simulink model "MIL4L3_SW6_V1_20220211"  (R2018b)
settings: Solver=FixedStepAuto  StartTime=0.0  StopTime=inf  FixedStep=0.001  RelTol=1e-3
PreLoadFcn:
  | A0_MILtest;
undefined symbols (not defined in the file or in its folder): Clb_ICADirect_LaneDisp_StateFive, Clb_ICADirect_LaneDisp_StateFour, Clb_ICADirect_LaneDisp_StateOne, Clb_ICADirect_LaneDisp_StateThree, Clb_ICADirect_LaneDisp_StateTwo, Clb_ICADirect_LaneDisp_StateZero, Clb_ICADirect_LaneDispSW, Clb_ICADirect_TrnLghtsCom_Switch, Clb_ICADirect_TrnLghtsCom_Value, Clb_ICADirect_TrnLghtsCrtl_Inhb, IMAP_Clb_ACU_Driver_Belt, IMAP_Clb_ACU_Driver_Belt_Over, IMAP_Clb_ACU_Passenger_Belt, IMAP_Clb_ACU_Passenger_Belt_Over, IMAP_Clb_ACU_RearLeft_Belt, IMAP_Clb_ACU_RearLeft_Belt_Over, IMAP_Clb_ACU_RearMiddle_Belt, IMAP_Clb_ACU_RearMiddle_Belt_Over, IMAP_Clb_ACU_RearRight_Belt, IMAP_Clb_ACU_RearRight_Belt_Over, IMAP_Clb_AEB_Switch, IMAP_Clb_AEB_Switch_Over, IMAP_Clb_ALC_TLC_Mode, IMAP_Clb_ALC_TLC_Mode_Over, IMAP_Clb_BCM_Battery_Voltage, IMAP_Clb_BCM_Battery_Voltage_Over, IMAP_Clb_BCM_BrakeLamp_State, IMAP_Clb_BCM_BrakeLamp_State_Over, IMAP_Clb_BCM_CHMSL_Status, IMAP_Clb_BCM_CHMSL_Status_Over, IMAP_Clb_BCM_Door_Lock_State, IMAP_Clb_BCM_Door_Lock_State_Over, IMAP_Clb_BCM_FrontWiper_State, IMAP_Clb_BCM_FrontWiper_State_Over, IMAP_Clb_BCM_FrontWiper_Switch, IMAP_Clb_BCM_FrontWiper_Switch_Over, IMAP_Clb_BCM_HazardLamp, IMAP_Clb_BCM_HazardLamp_Over, IMAP_Clb_BCM_HazardLamp_Switch, IMAP_Clb_BCM_HazardLamp_Switch_Over, IMAP_Clb_BCM_HighBeam_State, IMAP_Clb_BCM_HighBeam_State_Over, IMAP_Clb_BCM_Ignition_State, IMAP_Clb_BCM_Ignition_State_Over, IMAP_Clb_BCM_IHBC_Enabled, IMAP_Clb_BCM_IHBC_Enabled_Over, IMAP_Clb_BCM_Left_Light, IMAP_Clb_BCM_Left_Light_Over, IMAP_Clb_BCM_LeftTurn_Switch, IMAP_Clb_BCM_LeftTurn_Switch_Over, IMAP_Clb_BCM_LF_Door_State, IMAP_Clb_BCM_LF_Door_State_Over, IMAP_Clb_BCM_LowBeam_State, IMAP_Clb_BCM_LowBeam_State_Over, IMAP_Clb_BCM_LR_Door_State, IMAP_Clb_BCM_LR_Door_State_Over, IMAP_Clb_BCM_RF_Door_State, IMAP_Clb_BCM_RF_Door_State_Over, IMAP_Clb_BCM_Right_Light, IMAP_Clb_BCM_Right_Light_Over ... (+547)
libraries: CarMaker4SL x2153, simulink x292, dspstat3 x3, canmsglib x2, simulink_extras x1
(part 21 of 52)

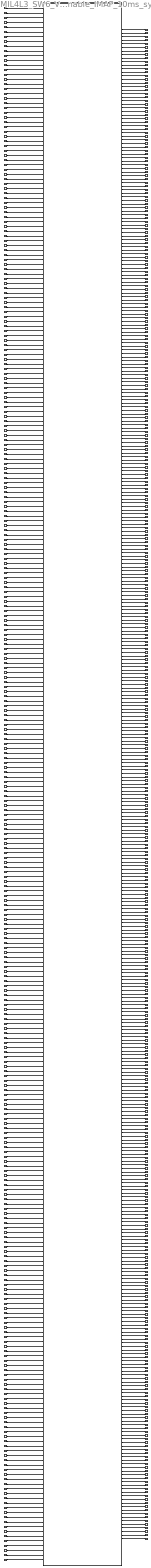
== system MIL4L3_SW6_V1_20220211/CarMaker/VehicleControl/Data Inport/IMAP/Runnable_IMAP_10ms_sys ==
  SWINve_y_ESC_ABSWorkLable : Inport  OutDataTypeStr=UInt8  PortDimensions=1
  SWINve_g_ESC_LongitudinalAcceleration : Inport  Port=2  OutDataTypeStr=T_M_Nm_Float32  PortDimensions=1
  SWINve_y_ESC_ESCOFF : Inport  Port=3  OutDataTypeStr=UInt8  PortDimensions=1
  SWINve_y_ESC_TCSCtlActive : Inport  Port=4  OutDataTypeStr=UInt8  PortDimensions=1
  SWINve_y_BCM_BrakeLampStaus : Inport  Port=5  OutDataTypeStr=UInt8  PortDimensions=1
  SWINve_y_BCM_CHMSLStaus : Inport  Port=6  OutDataTypeStr=UInt8  PortDimensions=1
  SWINve_y_BCM_FrontWiperWorkSt : Inport  Port=7  OutDataTypeStr=UInt8  PortDimensions=1
  SWINve_y_BCM_HazardLampSt : Inport  Port=8  OutDataTypeStr=UInt8  PortDimensions=1
  SWINve_y_EMS_BrakePedalSignal : Inport  Port=9  OutDataTypeStr=UInt8  PortDimensions=1
  SWINve_y_ESC_BrakingEffort : Inport  Port=10  OutDataTypeStr=UInt8  PortDimensions=1
  SWINve_y_ESC_DynamicSlope : Inport  Port=11  OutDataTypeStr=SInt8  PortDimensions=1
  SWINve_y_ESC_DynamicSlopeAccuracy : Inport  Port=12  OutDataTypeStr=UInt8  PortDimensions=1
  SWINve_y_EMS_WhetherACCRequestRealized : Inport  Port=13  OutDataTypeStr=UInt8  PortDimensions=1
  SWINve_y_EMS_ACCcontrolTorqueAvailable : Inport  Port=14  OutDataTypeStr=UInt8  PortDimensions=1
  SWINve_g_EMS_AccPedalPositionRaw : Inport  Port=15  OutDataTypeStr=T_M_Nm_Float32  PortDimensions=1
  SWINve_g_EMS_EngActualFlwTorque : Inport  Port=16  OutDataTypeStr=T_M_Nm_Float32  PortDimensions=1
  SWINve_d_EMS_RealizedPowertrainWheelTorq : Inport  Port=17  OutDataTypeStr=SInt16  PortDimensions=1
  SWINve_g_EMS_AccPedalPos : Inport  Port=18  OutDataTypeStr=T_M_Nm_Float32  PortDimensions=1
  SWINve_g_EMS_DriverTorque : Inport  Port=19  OutDataTypeStr=T_M_Nm_Float32  PortDimensions=1
  SWINve_g_EMS_EngSpd : Inport  Port=20  OutDataTypeStr=T_M_Nm_Float32  PortDimensions=1
  SWINve_y_EMS_EngRunningStatus : Inport  Port=21  OutDataTypeStr=UInt8  PortDimensions=1
  SWINve_y_EMS_ACCcontrolGearAvailable : Inport  Port=22  OutDataTypeStr=UInt8  PortDimensions=1
  SWINve_g_EMS_MaxPowertrainWheelTorque : Inport  Port=23  OutDataTypeStr=T_M_Nm_Float32  PortDimensions=1
  SWINve_g_EMS_NotControlableMaxPowertra : Inport  Port=24  OutDataTypeStr=T_M_Nm_Float32  PortDimensions=1
  SWINve_g_EMS_MinPowertrainWheelTorque : Inport  Port=25  OutDataTypeStr=T_M_Nm_Float32  PortDimensions=1
  SWINve_g_EMS_NotControlableMinPowertra : Inport  Port=26  OutDataTypeStr=T_M_Nm_Float32  PortDimensions=1
  SWINve_y_ESC_ESCWorkStatus : Inport  Port=27  OutDataTypeStr=UInt8  PortDimensions=1
  SWINve_y_ESC_FLWHeelPulseCounterValidity : Inport  Port=28  OutDataTypeStr=UInt8  PortDimensions=1
  SWINve_y_ESC_FRWHeelPulseCounterValidity : Inport  Port=29  OutDataTypeStr=UInt8  PortDimensions=1
  SWINve_y_BCM_IgnitionSt : Inport  Port=30  OutDataTypeStr=UInt8  PortDimensions=1
  SWINve_y_EMS_ACCFunctionIhibition : Inport  Port=31  OutDataTypeStr=UInt8  PortDimensions=1
  SWINve_y_EMS_ACCResponseStatus : Inport  Port=32  OutDataTypeStr=UInt8  PortDimensions=1
  SWINve_g_EMS_LowerestGearMaxTorque : Inport  Port=33  OutDataTypeStr=T_M_Nm_Float32  PortDimensions=1
  SWINve_g_EMS_HighestGearMinTorque : Inport  Port=34  OutDataTypeStr=T_M_Nm_Float32  PortDimensions=1
  SWINve_y_Mp5_ISASwitch : Inport  Port=35  OutDataTypeStr=UInt8  PortDimensions=1
  SWINve_y_Mp5_TSRSwitch : Inport  Port=36  OutDataTypeStr=UInt8  PortDimensions=1
  SWINve_y_SCC_LeftSteeringWheelSwitchSig : Inport  Port=37  OutDataTypeStr=UInt8  PortDimensions=1
  SWINve_y_SCC_RightSteeringWheelSwitchSig : Inport  Port=38  OutDataTypeStr=UInt8  PortDimensions=1
  SWINve_y_BCM_HazardSwitchrSt : Inport  Port=39  OutDataTypeStr=uint8  PortDimensions=1
  SWINve_y_MP5_HazardLampCtrlReq : Inport  Port=40  OutDataTypeStr=uint8  PortDimensions=1
  SWINve_y_T_box_RemoteHazardReq : Inport  Port=41  OutDataTypeStr=uint8  PortDimensions=1
  SWINve_y_BCM_HighBeamStatus : Inport  Port=42  OutDataTypeStr=UInt8  PortDimensions=1
  SWINve_y_MP5_FCWSwitch : Inport  Port=43  OutDataTypeStr=UInt8  PortDimensions=1
  SWINve_y_MP5_FCWSensitivity : Inport  Port=44  OutDataTypeStr=UInt8  PortDimensions=1
  SWINve_y_ACU_PassengerBeltSwitchSig : Inport  Port=45  OutDataTypeStr=UInt8  PortDimensions=1
  SWINve_y_ACU_DriverBeltSwitchSig : Inport  Port=46  OutDataTypeStr=UInt8  PortDimensions=1
  SWINve_y_SAS_SASFailureSts : Inport  Port=47  OutDataTypeStr=UInt8  PortDimensions=1
  SWINve_g_ESC_LateralAccelaration : Inport  Port=48  OutDataTypeStr=T_M_Nm_Float32  PortDimensions=1
  SWINve_y_Mp5_LSSMode : Inport  Port=49  OutDataTypeStr=UInt8  PortDimensions=1
  SWINve_y_Mp5_LSSSwitch : Inport  Port=50  OutDataTypeStr=UInt8  PortDimensions=1
  SWINve_y_ESC_BrakeReleasedFailsafe : Inport  Port=51  OutDataTypeStr=UInt8  PortDimensions=1
  SWINve_y_MP5_AEBSwitch : Inport  Port=52  OutDataTypeStr=UInt8  PortDimensions=1
  SWINve_y_ESC_MSRinRegulation : Inport  Port=53  OutDataTypeStr=UInt8  PortDimensions=1
  SWINve_g_ESC_FrontLeftWHeelSpd : Inport  Port=54  OutDataTypeStr=T_M_Nm_Float32  PortDimensions=1
  SWINve_g_ESC_FrontRightWHeelSpd : Inport  Port=55  OutDataTypeStr=T_M_Nm_Float32  PortDimensions=1
  SWINve_g_ESC_RearLeftWheelSpd : Inport  Port=56  OutDataTypeStr=T_M_Nm_Float32  PortDimensions=1
  SWINve_g_ESC_RearRightWheelSpd : Inport  Port=57  OutDataTypeStr=T_M_Nm_Float32  PortDimensions=1
  SWINve_g_IC_TotalOdemeter : Inport  Port=58  OutDataTypeStr=UInt32  PortDimensions=1
  SWINve_y_ESC_EPBStaus : Inport  Port=59  OutDataTypeStr=UInt8  PortDimensions=1
  SWINve_d_ESC_FLWHeelPulseCounter : Inport  Port=60  OutDataTypeStr=UInt16  PortDimensions=1
  SWINve_d_ESC_FRWHeelPulseCounter : Inport  Port=61  OutDataTypeStr=UInt16  PortDimensions=1
  SWINve_d_ESC_RLWHeelPulseCounter : Inport  Port=62  OutDataTypeStr=UInt16  PortDimensions=1
  SWINve_d_ESC_RRWHeelPulseCounter : Inport  Port=63  OutDataTypeStr=UInt16  PortDimensions=1
  SWINve_y_ESC_RLWHeelPulseCounterValidity : Inport  Port=64  OutDataTypeStr=UInt8  PortDimensions=1
  SWINve_y_ESC_RRWHeelPulseCounterValidity : Inport  Port=65  OutDataTypeStr=UInt8  PortDimensions=1
  SWINve_y_ESC_ESCAlarmSig : Inport  Port=66  OutDataTypeStr=UInt8  PortDimensions=1
  SWINve_y_EPS_SteeringHoldState : Inport  Port=67  OutDataTypeStr=UInt8  PortDimensions=1
  SWINve_y_EPS_LKAState : Inport  Port=68  OutDataTypeStr=UInt8  PortDimensions=1
  SWINve_y_ESC_Static_slope : Inport  Port=69  OutDataTypeStr=SInt8  PortDimensions=1
  SWINve_g_SAS_SteeringAngle : Inport  Port=70  OutDataTypeStr=T_M_Nm_Float32  PortDimensions=1
  SWINve_g_SAS_SteeringRotSpd : Inport  Port=71  OutDataTypeStr=T_M_Nm_Float32  PortDimensions=1
  SWINve_g_EPS_SteeringTorqueValue : Inport  Port=72  OutDataTypeStr=T_M_Nm_Float32  PortDimensions=1
  SWINve_y_SAS_CalibratedStatus : Inport  Port=73  OutDataTypeStr=UInt8  PortDimensions=1
  SWINve_y_SAS_TrimmingStatus : Inport  Port=74  OutDataTypeStr=UInt8  PortDimensions=1
  SWINve_y_TCU_TargetGear : Inport  Port=75  OutDataTypeStr=UInt8  PortDimensions=1
  SWINve_y_TCU_ATFailure : Inport  Port=76  OutDataTypeStr=UInt8  PortDimensions=1
  SWINve_y_GW_TCU_DCTClutchStatus : Inport  Port=77  OutDataTypeStr=UInt8  PortDimensions=1
  SWINve_y_TCU_ActialGear : Inport  Port=78  OutDataTypeStr=UInt8  PortDimensions=1
  SWINve_y_TCU_GearEngagement : Inport  Port=79  OutDataTypeStr=UInt8  PortDimensions=1
  SWINve_y_TCU_SelectedATMode : Inport  Port=80  OutDataTypeStr=UInt8  PortDimensions=1
  SWINve_g_ESC_BrakeOilPress : Inport  Port=81  OutDataTypeStr=T_M_Nm_Float32  PortDimensions=1
  SWINve_y_EPS_TorqueLimitationState : Inport  Port=82  OutDataTypeStr=UInt8  PortDimensions=1
  SWINve_y_ESC_VehicleStandstill : Inport  Port=83  OutDataTypeStr=UInt8  PortDimensions=1
  SWINve_y_ESC_VehDrivingDirection : Inport  Port=84  OutDataTypeStr=UInt8  PortDimensions=1
  SWINve_y_ESC_VehicleHoldStatus : Inport  Port=85  OutDataTypeStr=UInt8  PortDimensions=1
  SWINve_g_ESC_VeSpd : Inport  Port=86  OutDataTypeStr=T_M_Nm_Float32  PortDimensions=1
  SWINve_y_ESC_VehSpdValidFlag : Inport  Port=87  OutDataTypeStr=UInt8  PortDimensions=1
  SWINve_g_ESC_YawRate : Inport  Port=88  OutDataTypeStr=T_M_Nm_Float32  PortDimensions=1
  SWINve_g_ESC_UnfilteredYawRate : Inport  Port=89  OutDataTypeStr=T_M_Nm_Float32  PortDimensions=1
  System_Clock : Inport  Port=90  OutDataTypeStr=UInt16  PortDimensions=1
  SDFAve_d_sensor_status : Inport  Port=91  OutDataTypeStr=UInt16  PortDimensions=1
  SDFAve_d_sen_sta_LF_radar : Inport  Port=92  OutDataTypeStr=UInt16  PortDimensions=1
  SDFAve_d_sen_sta_RF_radar : Inport  Port=93  OutDataTypeStr=UInt16  PortDimensions=1
  SDFAve_d_sen_sta_LB_radar : Inport  Port=94  OutDataTypeStr=UInt16  PortDimensions=1
  SDFAve_d_sen_sta_RB_radar : Inport  Port=95  OutDataTypeStr=UInt16  PortDimensions=1
  SDFAve_d_fusion_status : Inport  Port=96  OutDataTypeStr=UInt16  PortDimensions=1
  SDFAve_d_fusion_time_stamp : Inport  Port=97  OutDataTypeStr=UInt16  PortDimensions=1
  SDFAve_d_obj_Num : Inport  Port=98  OutDataTypeStr=UInt16  PortDimensions=1
  SDFAva_y_obj_id : Inport  Port=99  OutDataTypeStr=UInt8  PortDimensions=40
  SDFAva_g_obj_pos_x : Inport  Port=100  OutDataTypeStr=T_M_Nm_Float32  PortDimensions=40
  SDFAva_g_obj_pos_y : Inport  Port=101  OutDataTypeStr=T_M_Nm_Float32  PortDimensions=40
  SDFAva_g_obj_vel_x : Inport  Port=102  OutDataTypeStr=T_M_Nm_Float32  PortDimensions=40
  SDFAva_g_obj_vel_y : Inport  Port=103  OutDataTypeStr=T_M_Nm_Float32  PortDimensions=40
  SDFAva_g_obj_acc_x : Inport  Port=104  OutDataTypeStr=T_M_Nm_Float32  PortDimensions=40
  SDFAva_g_obj_acc_y : Inport  Port=105  OutDataTypeStr=T_M_Nm_Float32  PortDimensions=40
  SDFAva_g_obj_pos_var_x : Inport  Port=106  OutDataTypeStr=T_M_Nm_Float32  PortDimensions=40
  SDFAva_g_obj_pos_var_y : Inport  Port=107  OutDataTypeStr=T_M_Nm_Float32  PortDimensions=40
  SDFAva_g_obj_pos_var_xy : Inport  Port=108  OutDataTypeStr=T_M_Nm_Float32  PortDimensions=40
  SDFAva_g_obj_width : Inport  Port=109  OutDataTypeStr=T_M_Nm_Float32  PortDimensions=40
  SDFAva_g_obj_length : Inport  Port=110  OutDataTypeStr=T_M_Nm_Float32  PortDimensions=40
  SDFAva_y_obj_class : Inport  Port=111  OutDataTypeStr=UInt8  PortDimensions=40
  SDFAva_y_obj_lane : Inport  Port=112  OutDataTypeStr=UInt8  PortDimensions=40
  SDFAva_d_obj_status : Inport  Port=113  OutDataTypeStr=UInt16  PortDimensions=40
  SDFAva_d_obj_age : Inport  Port=114  OutDataTypeStr=UInt16  PortDimensions=40
  SDFAva_y_obj_TurnLight : Inport  Port=115  OutDataTypeStr=UInt8  PortDimensions=40
  SDFAva_y_obj_BrakeLight : Inport  Port=116  OutDataTypeStr=UInt8  PortDimensions=40
  SDFAva_y_obj_MotionStatus : Inport  Port=117  OutDataTypeStr=UInt8  PortDimensions=40
  SDFAve_y_ROAD_TYPE : Inport  Port=118  OutDataTypeStr=UInt8  PortDimensions=1
  SDFAve_g_L0_C0_COEF : Inport  Port=119  OutDataTypeStr=T_M_Nm_Float32  PortDimensions=1
  SDFAve_g_L0_C1_COEF : Inport  Port=120  OutDataTypeStr=T_M_Nm_Float32  PortDimensions=1
  SDFAve_g_L0_C2_COEF : Inport  Port=121  OutDataTypeStr=T_M_Nm_Float32  PortDimensions=1
  SDFAve_g_L0_C3_COEF : Inport  Port=122  OutDataTypeStr=T_M_Nm_Float32  PortDimensions=1
  SDFAve_g_L0_VIEW_RANGE : Inport  Port=123  OutDataTypeStr=T_M_Nm_Float32  PortDimensions=1
  SDFAve_y_L0_DETECT_QUALITY : Inport  Port=124  OutDataTypeStr=UInt8  PortDimensions=1
  SDFAve_d_L0_LINE_TYPE : Inport  Port=125  OutDataTypeStr=UInt16  PortDimensions=1
  SDFAve_g_L0_MARK_WIDTH : Inport  Port=126  OutDataTypeStr=T_M_Nm_Float32  PortDimensions=1
  SDFAve_g_R0_C0_COEF : Inport  Port=127  OutDataTypeStr=T_M_Nm_Float32  PortDimensions=1
  SDFAve_g_R0_C1_COEF : Inport  Port=128  OutDataTypeStr=T_M_Nm_Float32  PortDimensions=1
  SDFAve_g_R0_C2_COEF : Inport  Port=129  OutDataTypeStr=T_M_Nm_Float32  PortDimensions=1
  SDFAve_g_R0_C3_COEF : Inport  Port=130  OutDataTypeStr=T_M_Nm_Float32  PortDimensions=1
  SDFAve_g_R0_VIEW_RANGE : Inport  Port=131  OutDataTypeStr=T_M_Nm_Float32  PortDimensions=1
  SDFAve_y_R0_DETECT_QUALITY : Inport  Port=132  OutDataTypeStr=UInt8  PortDimensions=1
  SDFAve_d_R0_LINE_TYPE : Inport  Port=133  OutDataTypeStr=UInt16  PortDimensions=1
  SDFAve_g_R0_MARK_WIDTH : Inport  Port=134  OutDataTypeStr=T_M_Nm_Float32  PortDimensions=1
  SDFAve_g_L1_C0_COEF : Inport  Port=135  OutDataTypeStr=T_M_Nm_Float32  PortDimensions=1
  SDFAve_g_L1_C1_COEF : Inport  Port=136  OutDataTypeStr=T_M_Nm_Float32  PortDimensions=1
  SDFAve_g_L1_C2_COEF : Inport  Port=137  OutDataTypeStr=T_M_Nm_Float32  PortDimensions=1
  SDFAve_g_L1_C3_COEF : Inport  Port=138  OutDataTypeStr=T_M_Nm_Float32  PortDimensions=1
  SDFAve_g_L1_VIEW_RANGE : Inport  Port=139  OutDataTypeStr=T_M_Nm_Float32  PortDimensions=1
  SDFAve_y_L1_DETECT_QUALITY : Inport  Port=140  OutDataTypeStr=UInt8  PortDimensions=1
  SDFAve_d_L1_LINE_TYPE : Inport  Port=141  OutDataTypeStr=UInt16  PortDimensions=1
  SDFAve_g_L1_MARK_WIDTH : Inport  Port=142  OutDataTypeStr=T_M_Nm_Float32  PortDimensions=1
  SDFAve_g_R1_C0_COEF : Inport  Port=143  OutDataTypeStr=T_M_Nm_Float32  PortDimensions=1
  SDFAve_g_R1_C1_COEF : Inport  Port=144  OutDataTypeStr=T_M_Nm_Float32  PortDimensions=1
  SDFAve_g_R1_C2_COEF : Inport  Port=145  OutDataTypeStr=T_M_Nm_Float32  PortDimensions=1
  SDFAve_g_R1_C3_COEF : Inport  Port=146  OutDataTypeStr=T_M_Nm_Float32  PortDimensions=1
  SDFAve_g_R1_VIEW_RANGE : Inport  Port=147  OutDataTypeStr=T_M_Nm_Float32  PortDimensions=1
  SDFAve_y_R1_DETECT_QUALITY : Inport  Port=148  OutDataTypeStr=UInt8  PortDimensions=1
  SDFAve_d_R1_LINE_TYPE : Inport  Port=149  OutDataTypeStr=UInt16  PortDimensions=1
  SDFAve_g_R1_MARK_WIDTH : Inport  Port=150  OutDataTypeStr=T_M_Nm_Float32  PortDimensions=1
  SDFAve_g_L0_C0_BACK_COEF : Inport  Port=151  OutDataTypeStr=T_M_Nm_Float32  PortDimensions=1
  SDFAve_g_L0_C1_BACK_COEF : Inport  Port=152  OutDataTypeStr=T_M_Nm_Float32  PortDimensions=1
  SDFAve_g_L0_C2_BACK_COEF : Inport  Port=153  OutDataTypeStr=T_M_Nm_Float32  PortDimensions=1
  SDFAve_g_L0_C3_BACK_COEF : Inport  Port=154  OutDataTypeStr=T_M_Nm_Float32  PortDimensions=1
  SDFAve_g_L0_BACK_RANGE : Inport  Port=155  OutDataTypeStr=T_M_Nm_Float32  PortDimensions=1
  SDFAve_g_R0_C0_BACK_COEF : Inport  Port=156  OutDataTypeStr=T_M_Nm_Float32  PortDimensions=1
  SDFAve_g_R0_C1_BACK_COEF : Inport  Port=157  OutDataTypeStr=T_M_Nm_Float32  PortDimensions=1
  SDFAve_g_R0_C2_BACK_COEF : Inport  Port=158  OutDataTypeStr=T_M_Nm_Float32  PortDimensions=1
  SDFAve_g_R0_C3_BACK_COEF : Inport  Port=159  OutDataTypeStr=T_M_Nm_Float32  PortDimensions=1
  SDFAve_g_R0_BACK_RANGE : Inport  Port=160  OutDataTypeStr=T_M_Nm_Float32  PortDimensions=1
  SDFAve_g_L1_C0_BACK_COEF : Inport  Port=161  OutDataTypeStr=T_M_Nm_Float32  PortDimensions=1
  SDFAve_g_L1_C1_BACK_COEF : Inport  Port=162  OutDataTypeStr=T_M_Nm_Float32  PortDimensions=1
  SDFAve_g_L1_C2_BACK_COEF : Inport  Port=163  OutDataTypeStr=T_M_Nm_Float32  PortDimensions=1
  SDFAve_g_L1_C3_BACK_COEF : Inport  Port=164  OutDataTypeStr=T_M_Nm_Float32  PortDimensions=1
  SDFAve_g_L1_BACK_RANGE : Inport  Port=165  OutDataTypeStr=T_M_Nm_Float32  PortDimensions=1
  SDFAve_g_R1_C0_BACK_COEF : Inport  Port=166  OutDataTypeStr=T_M_Nm_Float32  PortDimensions=1
  SDFAve_g_R1_C1_BACK_COEF : Inport  Port=167  OutDataTypeStr=T_M_Nm_Float32  PortDimensions=1
  SDFAve_g_R1_C2_BACK_COEF : Inport  Port=168  OutDataTypeStr=T_M_Nm_Float32  PortDimensions=1
  SDFAve_g_R1_C3_BACK_COEF : Inport  Port=169  OutDataTypeStr=T_M_Nm_Float32  PortDimensions=1
  SDFAve_g_R1_BACK_RANGE : Inport  Port=170  OutDataTypeStr=T_M_Nm_Float32  PortDimensions=1
  SDFAve_g_Lrg_C0_BACK_COEF : Inport  Port=171  OutDataTypeStr=T_M_Nm_Float32
  SDFAve_g_Lrg_C1_BACK_COEF : Inport  Port=172  OutDataTypeStr=T_M_Nm_Float32
  SDFAve_g_Lrg_C2_BACK_COEF : Inport  Port=173  OutDataTypeStr=T_M_Nm_Float32
  SDFAve_g_Lrg_C3_BACK_COEF : Inport  Port=174  OutDataTypeStr=T_M_Nm_Float32
  SDFAve_g_Lrg_VIEW_RANGE_start : Inport  Port=175  OutDataTypeStr=T_M_Nm_Float32
  SDFAve_g_Lrg_VIEW_RANGE_end : Inport  Port=176  OutDataTypeStr=T_M_Nm_Float32
  SDFAve_y_Lrg_DETECT_QUALITY : Inport  Port=177  OutDataTypeStr=UInt8
  SDFAve_y_Lrg_LINE_TYPE : Inport  Port=178  OutDataTypeStr=UInt8
  SDFAve_g_Rrg_C0_BACK_COEF : Inport  Port=179  OutDataTypeStr=T_M_Nm_Float32
  SDFAve_g_Rrg_C1_BACK_COEF : Inport  Port=180  OutDataTypeStr=T_M_Nm_Float32
  SDFAve_g_Rrg_C2_BACK_COEF : Inport  Port=181  OutDataTypeStr=T_M_Nm_Float32
  SDFAve_g_Rrg_C3_BACK_COEF : Inport  Port=182  OutDataTypeStr=T_M_Nm_Float32
  SDFAve_g_Rrg_VIEW_RANGE_start : Inport  Port=183  OutDataTypeStr=T_M_Nm_Float32
  SDFAve_g_Rrg_VIEW_RANGE_end : Inport  Port=184  OutDataTypeStr=T_M_Nm_Float32
  SDFAve_y_Rrg_DETECT_QUALITY : Inport  Port=185  OutDataTypeStr=UInt8
  SDFAve_y_Rrg_LINE_TYPE : Inport  Port=186  OutDataTypeStr=UInt8
  SDFAve_y_ISAValue : Inport  Port=187  OutDataTypeStr=UInt8  PortDimensions=1
  SDFAve_y_ISAPopupMessage : Inport  Port=188  OutDataTypeStr=uint8
  SDFAve_y_ISASignType : Inport  Port=189  OutDataTypeStr=uint8
  SDFAve_y_ISAStatus : Inport  Port=190  OutDataTypeStr=uint8
  SDFAve_y_TSR_Sign_Type : Inport  Port=191  OutDataTypeStr=UInt8  PortDimensions=1
  SDFAve_g_CameraSignalFault : Inport  Port=192  OutDataTypeStr=T_M_Nm_Float32  PortDimensions=1
  SDFAve_y_Radar_State : Inport  Port=193  OutDataTypeStr=UInt8  PortDimensions=1
  SDFAve_y_OperatingStatus : Inport  Port=194  OutDataTypeStr=UInt8  PortDimensions=1
  SDFAve_y_Radar_FaultBitSetting_Signal : Inport  Port=195
  SWINve_y_ESC_FLWDirection : Inport  Port=196  OutDataTypeStr=UInt8  PortDimensions=1
  SWINve_y_ESC_FRWDirection : Inport  Port=197  OutDataTypeStr=UInt8  PortDimensions=1
  SWINve_y_ESC_TCSErrorStatus : Inport  Port=198  OutDataTypeStr=UInt8  PortDimensions=1
  SWINve_y_ESC-RLWDirection : Inport  Port=199  OutDataTypeStr=UInt8  PortDimensions=1
  SWINve_y_ESC_RRWDirection : Inport  Port=200  OutDataTypeStr=UInt8  PortDimensions=1
  SWINve_y_ESC_EPBErrorStatus : Inport  Port=201  OutDataTypeStr=UInt8  PortDimensions=1
  SWINve_y_EPS_SteeringAngle_Flag : Inport  Port=202  OutDataTypeStr=UInt8  PortDimensions=1
  SWINve_g_EPS_SteeringAngle : Inport  Port=203  OutDataTypeStr=T_M_Nm_Float32  PortDimensions=1
  SWINve_y_EPS_DriverOverride : Inport  Port=204  OutDataTypeStr=UInt8  PortDimensions=1
  SWINve_y_EPS_DriverInitializedESA : Inport  Port=205  OutDataTypeStr=UInt8
  SWINve_y_EPS_ESAState : Inport  Port=206  OutDataTypeStr=UInt8
  SWINve_y_ACU_RearLeftBeltSwitchSig : Inport  Port=207  OutDataTypeStr=UInt8
  SWINve_y_ACU_RearMiddleBeltSwitchSig : Inport  Port=208  OutDataTypeStr=UInt8
  SWINve_y_ACU_RearRightBeltSwitchSig : Inport  Port=209  OutDataTypeStr=UInt8
  SWINve_y_EMS_PowertrainControlSt : Inport  Port=210  OutDataTypeStr=UInt8
  SWINve_y_TCU_TCUAvailable : Inport  Port=211  OutDataTypeStr=UInt8
  SWINve_y_BCM_LeftTurnSwitchSt : Inport  Port=212  OutDataTypeStr=UInt8
  SWINve_y_BCM_RightTurnSwitchSt : Inport  Port=213  OutDataTypeStr=UInt8
  SWINve_y_BCM_FrontWiperSwitchSt : Inport  Port=214  OutDataTypeStr=UInt8
  SWINve_y_BCM_IHBC_Function_Enable : Inport  Port=215  OutDataTypeStr=UInt8
  SWINve_y_MP5_WorkSt : Inport  Port=216  OutDataTypeStr=UInt8
  SWINve_y_MP5_APAModeSelect : Inport  Port=217  OutDataTypeStr=UInt8
  SWINve_y_MP5_Language_Set : Inport  Port=218  OutDataTypeStr=UInt8
  SWINve_y_MP5_UPA_switch : Inport  Port=219  OutDataTypeStr=UInt8
  SWINve_y_MP5_FLKAActivation : Inport  Port=220  OutDataTypeStr=UInt8
  SWINve_y_MP5_AutoPilotSwitch : Inport  Port=221  OutDataTypeStr=UInt8
  SWINve_y_MP5_MDS_Message_type : Inport  Port=222  OutDataTypeStr=UInt8
  SWINve_y_MP5_DMS_SystemEnable : Inport  Port=223  OutDataTypeStr=UInt8
  SWINve_y_MP5_DMS_DeleteUserNum : Inport  Port=224  OutDataTypeStr=UInt8
  SWINve_y_MP5_DMS_Sensity : Inport  Port=225  OutDataTypeStr=UInt8
  SWINve_y_MP5_DMS_EyeFatigueMonitor : Inport  Port=226  OutDataTypeStr=UInt8
  SWINve_y_MP5_DMS_LongtimeDriveMonitor : Inport  Port=227  OutDataTypeStr=UInt8
  SWINve_y_MP5_DMS_SideViewMonitor : Inport  Port=228  OutDataTypeStr=UInt8
  SWINve_y_MP5_DMS_UsingPhoneMonitor : Inport  Port=229  OutDataTypeStr=UInt8
  SWINve_y_MP5_DMS_SmokingMonitor : Inport  Port=230  OutDataTypeStr=UInt8
  SWINve_y_MP5_DMS_DrinkWaterMonitor : Inport  Port=231  OutDataTypeStr=UInt8
  SWINve_y_MP5_DMS_UserAccount : Inport  Port=232  OutDataTypeStr=UInt8
  SWINve_y_Mp5_ISAMode : Inport  Port=233  OutDataTypeStr=UInt8  PortDimensions=1
  SWINve_y_Mp5_LDWWarningMode : Inport  Port=234  OutDataTypeStr=UInt8  PortDimensions=1
  SWINve_y_MP5_ADASSpeedLimit : Inport  Port=235  OutDataTypeStr=UInt8  PortDimensions=1
  SWINve_y_MP5_TLCModeSelection : Inport  Port=236  OutDataTypeStr=UInt8  PortDimensions=1
  SWINve_y_MP5_ESASwitch : Inport  Port=237  OutDataTypeStr=UInt8  PortDimensions=1
  SWINve_y_Mp5_ELKSwitch : Inport  Port=238  OutDataTypeStr=UInt8  PortDimensions=1
  SWINve_y_PEPS_RKECommand : Inport  Port=239  OutDataTypeStr=UInt8  PortDimensions=1
  SWINve_y_MP5_BSD_LCW_Activation : Inport  Port=240  OutDataTypeStr=UInt8  PortDimensions=1
  SWINve_y_MP5_FCTAActivation : Inport  Port=241  OutDataTypeStr=UInt8  PortDimensions=1
  SWINve_y_MP5_RCTAActivation : Inport  Port=242  OutDataTypeStr=UInt8  PortDimensions=1
  SWINve_y_MP5_DOWActivation : Inport  Port=243  OutDataTypeStr=UInt8
  SWINve_y_MP5_JA_Modes : Inport  Port=244  OutDataTypeStr=UInt8
  SWINve_y_MP5_JA_Alert_Switch : Inport  Port=245  OutDataTypeStr=UInt8
  SWINve_y_ESC_BLRequest : Inport  Port=246  OutDataTypeStr=UInt8  PortDimensions=1
  SWINve_y_PEPS_DoorLockReq : Inport  Port=247  OutDataTypeStr=UInt8  PortDimensions=1
  SWINve_y_BCM_DoorLockSt : Inport  Port=248  OutDataTypeStr=UInt8  PortDimensions=1
  SWINve_y_BCM_LowBeamStatus : Inport  Port=249  OutDataTypeStr=UInt8  PortDimensions=1
  SWINve_g_BCM_BattVolt : Inport  Port=250  OutDataTypeStr=T_M_Nm_Float32  PortDimensions=1
  SWINve_d_TBOX_LocalTimeYear : Inport  Port=251  OutDataTypeStr=UInt16  PortDimensions=1
  SWINve_y_TBOX_LocalTimeMounth : Inport  Port=252  OutDataTypeStr=UInt8  PortDimensions=1
  SWINve_y_TBOX_LocalTimeDate : Inport  Port=253  OutDataTypeStr=UInt8  PortDimensions=1
  SWINve_y_TBOX_LocalTimeHour : Inport  Port=254  OutDataTypeStr=UInt8  PortDimensions=1
  SWINve_y_TBOX_LocalTimeMinute : Inport  Port=255  OutDataTypeStr=UInt8
  SWINve_y_TBOX_LocalTimeSecond : Inport  Port=256  OutDataTypeStr=UInt8
  SWINve_y_TBOX_LocalTimeValid : Inport  Port=257  OutDataTypeStr=UInt8
  SWINve_g_AC_AmbTemp : Inport  Port=258  OutDataTypeStr=T_M_Nm_Float32
  SWINve_y_EPS_SteerintTorqueSensorSt : Inport  Port=259  OutDataTypeStr=UInt8  PortDimensions=1
  SWINve_g_EPS_LKACurrentOverlay : Inport  Port=260  OutDataTypeStr=T_M_Nm_Float32  PortDimensions=1
  SWINve_y_EPS_WarmingLampSt : Inport  Port=261  OutDataTypeStr=UInt8  PortDimensions=1
  SWINve_g_EPS_ElectPowerConsumption : Inport  Port=262  OutDataTypeStr=T_M_Nm_Float32  PortDimensions=1
  SWINve_g_EMS_EngActualIndTorque : Inport  Port=263  OutDataTypeStr=T_M_Nm_Float32  PortDimensions=1
  SWINve_y_EMS_AccPedalFaultBit : Inport  Port=264  OutDataTypeStr=UInt8  PortDimensions=1
  SWINve_y_TCU_PRNDLStatus : Inport  Port=265  OutDataTypeStr=UInt8  PortDimensions=1
  SWINve_y_TCU_ShiftLeverPosValidFlag : Inport  Port=266  OutDataTypeStr=UInt8  PortDimensions=1
  SWINve_y_ESC_LateralAccelarationValidity : Inport  Port=267  OutDataTypeStr=UInt8  PortDimensions=1
  SWINve_y_ESC_YawrateValidity : Inport  Port=268  OutDataTypeStr=UInt8
  SWINve_y_ESC_LongitudinalAccelervalidity : Inport  Port=269  OutDataTypeStr=UInt8
  SWINve_y_ESC_ABSValidity : Inport  Port=270  OutDataTypeStr=UInt8
  SWINve_y_ESC_ABSAlarmSig : Inport  Port=271  OutDataTypeStr=UInt8
  SWINve_y_ESC_FLWHeelSpdFaultSignal : Inport  Port=272  OutDataTypeStr=UInt8
  SWINve_y_ESC_FRWHeelSpdFaultSignal : Inport  Port=273  OutDataTypeStr=UInt8
  SWINve_y_ESC_RLWHeelSpdFaultSignal : Inport  Port=274  OutDataTypeStr=UInt8
  SWINve_y_ESC_RRWHeelSpdFaultSignal : Inport  Port=275  OutDataTypeStr=UInt8
  SWINve_y_ESC_AEBAvailable : Inport  Port=276  OutDataTypeStr=UInt8
  SWINve_y_ESC_AEBActive : Inport  Port=277  OutDataTypeStr=UInt8
  SWINve_y_ESC_ACCAvailable : Inport  Port=278  OutDataTypeStr=UInt8
  SWINve_y_ESC_ACCActive : Inport  Port=279  OutDataTypeStr=UInt8
  SWINve_y_ESC_EPBDisplayMessageReq : Inport  Port=280  OutDataTypeStr=UInt8
  SWINve_y_ESC_EPBWarmingIndicationReq : Inport  Port=281  OutDataTypeStr=UInt8
  SWINve_y_ESC_EPBSwitchStatics : Inport  Port=282  OutDataTypeStr=UInt8
  SWINve_y_ESC_EPBSwitchStaticsValidity : Inport  Port=283  OutDataTypeStr=UInt8
  SWINve_y_ESC_EBDAlarmSig : Inport  Port=284  OutDataTypeStr=UInt8
  SWINve_y_ESC_AVHStatus : Inport  Port=285  OutDataTypeStr=UInt8
  SWINve_y_BCM_LeftlightSt : Inport  Port=286  OutDataTypeStr=UInt8  PortDimensions=1
  SWINve_y_BCM_RightlightSt : Inport  Port=287  OutDataTypeStr=UInt8  PortDimensions=1
  SWINve_y_BCM_TrunkSt : Inport  Port=288  OutDataTypeStr=UInt8  PortDimensions=1
  SWINve_y_BCM_LFDoorSwitchSt : Inport  Port=289  OutDataTypeStr=UInt8  PortDimensions=1
  SWINve_y_BCM_RFDoorSwitchSt : Inport  Port=290  OutDataTypeStr=UInt8  PortDimensions=1
  SWINve_y_BCM_RRDoorSwitchSt : Inport  Port=291  OutDataTypeStr=UInt8  PortDimensions=1
  SWINve_y_BCM_LRDoorSwitchSt : Inport  Port=292  OutDataTypeStr=UInt8  PortDimensions=1
  SWINve_g_ESC_BrakeWheelCylinderPressure : Inport  Port=293  OutDataTypeStr=T_M_Nm_Float32  PortDimensions=1
  FAPAve_Cnt_AdvancedParkingAssist : Inport  Port=294  OutDataTypeStr=T_Cnt_Num_1_1_u8
  SDFAve_d_ORI_CIPV_ID : Inport  Port=295  OutDataTypeStr=uint16
  SDFAve_d_ORI_Obj_Num : Inport  Port=296  OutDataTypeStr=uint16
  SDFAva_d_ORI_Obj_Class : Inport  Port=297  OutDataTypeStr=uint16  PortDimensions=20
  SDFAva_d_ORI_Obj_ID : Inport  Port=298  OutDataTypeStr=uint16  PortDimensions=20
  SDFAva_g_ORI_Obj_AbsAx : Inport  Port=299  OutDataTypeStr=single  PortDimensions=20
  SDFAva_g_ORI_Obj_AbsAy : Inport  Port=300  OutDataTypeStr=single  PortDimensions=20
  SDFAva_g_ORI_Obj_RelVel : Inport  Port=301  OutDataTypeStr=single  PortDimensions=20
  SDFAva_g_ORI_Obj_RelVely : Inport  Port=302  OutDataTypeStr=single  PortDimensions=20
  SDFAva_g_ORI_Obj_LongDis : Inport  Port=303  OutDataTypeStr=single  PortDimensions=20
  SDFAva_g_ORI_Obj_LateralDis : Inport  Port=304  OutDataTypeStr=single  PortDimensions=20
  SDFAve_g_ORI_L0_C3 : Inport  Port=305  OutDataTypeStr=single
  SDFAve_g_ORI_L0_C2 : Inport  Port=306  OutDataTypeStr=single
  SDFAve_g_ORI_L0_C1 : Inport  Port=307  OutDataTypeStr=single
  SDFAve_g_ORI_L0_C0 : Inport  Port=308  OutDataTypeStr=single
  SDFAve_d_ORI_L0_Type : Inport  Port=309  OutDataTypeStr=uint16
  SDFAve_g_ORI_L0_VR : Inport  Port=310  OutDataTypeStr=single
  SDFAve_g_ORI_L1_C3 : Inport  Port=311  OutDataTypeStr=single
  SDFAve_g_ORI_L1_C2 : Inport  Port=312  OutDataTypeStr=single
  SDFAve_g_ORI_L1_C1 : Inport  Port=313  OutDataTypeStr=single
  SDFAve_g_ORI_L1_C0 : Inport  Port=314  OutDataTypeStr=single
  SDFAve_d_ORI_L1_Type : Inport  Port=315  OutDataTypeStr=uint16
  SDFAve_g_ORI_L1_VR : Inport  Port=316  OutDataTypeStr=single
  SDFAve_g_ORI_R0_C3 : Inport  Port=317  OutDataTypeStr=single
  SDFAve_g_ORI_R0_C2 : Inport  Port=318  OutDataTypeStr=single
  SDFAve_g_ORI_R0_C1 : Inport  Port=319  OutDataTypeStr=single
  SDFAve_g_ORI_R0_C0 : Inport  Port=320  OutDataTypeStr=single
  SDFAve_d_ORI_R0_LT : Inport  Port=321  OutDataTypeStr=uint16
  SDFAve_g_ORI_R0_VR : Inport  Port=322  OutDataTypeStr=single
  SDFAve_g_ORI_R1_C3 : Inport  Port=323  OutDataTypeStr=single
  SDFAve_g_ORI_R1_C2 : Inport  Port=324  OutDataTypeStr=single
  SDFAve_g_ORI_R1_C1 : Inport  Port=325  OutDataTypeStr=single
  SDFAve_g_ORI_R1_C0 : Inport  Port=326  OutDataTypeStr=single
  SDFAve_d_ORI_R1_LT : Inport  Port=327  OutDataTypeStr=uint16
  SDFAve_g_ORI_R1_VR : Inport  Port=328  OutDataTypeStr=single
  Runnable_IMAP_10ms_sys : Subsystem  TreatAsAtomicUnit=on
  IMAPve_d_LKA_Main_Switch : Outport  OutDataTypeStr=UInt16  PortDimensions=1
  IMAPve_d_LKA_Mode : Outport  Port=2  OutDataTypeStr=UInt16  PortDimensions=1
  IMAPve_d_AEB_Switch : Outport  Port=3  OutDataTypeStr=UInt16  PortDimensions=1
  IMAPve_d_FCW_Switch : Outport  Port=4  OutDataTypeStr=UInt16  PortDimensions=1
  IMAPve_d_FCW_Sensitivity : Outport  Port=5  OutDataTypeStr=UInt16  PortDimensions=1
  IMAPve_d_ISA_Switch : Outport  Port=6  OutDataTypeStr=UInt16  PortDimensions=1
  IMAPve_d_TSR_Switch : Outport  Port=7  OutDataTypeStr=UInt16  PortDimensions=1
  IMAPve_d_ISA_ISLC_Mode : Outport  Port=8  OutDataTypeStr=UInt16  PortDimensions=1
  IMAPve_d_LDW_Warn_Mode : Outport  Port=9  OutDataTypeStr=UInt16  PortDimensions=1
  IMAPve_d_Speed_Limit : Outport  Port=10  OutDataTypeStr=UInt16  PortDimensions=1
  IMAPve_d_ALC_TLC_Mode : Outport  Port=11  OutDataTypeStr=UInt16  PortDimensions=1
  IMAPve_d_ESA_Switch : Outport  Port=12  OutDataTypeStr=UInt16  PortDimensions=1
  IMAPve_d_ELK_Switch : Outport  Port=13  OutDataTypeStr=UInt16  PortDimensions=1
  IMAPve_d_PEPS_RKE_Command : Outport  Port=14  OutDataTypeStr=UInt16  PortDimensions=1
  IMAPve_d_BSD_LCW_Switch : Outport  Port=15  OutDataTypeStr=UInt16  PortDimensions=1
  IMAPve_d_FCTA_Switch : Outport  Port=16  OutDataTypeStr=UInt16  PortDimensions=1
  IMAPve_d_RCTA_Swtich : Outport  Port=17  OutDataTypeStr=UInt16  PortDimensions=1
  IMAPve_d_DOW_Switch : Outport  Port=18  OutDataTypeStr=UInt16  PortDimensions=1
  IMAPve_d_JA_Brake_Switch : Outport  Port=19  OutDataTypeStr=UInt16  PortDimensions=1
  IMAPve_d_JA_Alert_Switch : Outport  Port=20  OutDataTypeStr=UInt16  PortDimensions=1
  IMAPve_d_EPS_LKA_State : Outport  Port=21  OutDataTypeStr=UInt16  PortDimensions=1
  IMAPve_g_EPS_SW_Trq : Outport  Port=22  OutDataTypeStr=T_M_Nm_Float32  PortDimensions=1
  IMAPve_d_EPS_Trq_State : Outport  Port=23  OutDataTypeStr=UInt16  PortDimensions=1
  IMAPve_d_SAS_Clb_State : Outport  Port=24  OutDataTypeStr=UInt16  PortDimensions=1
  IMAPve_d_SAS_Trim_State : Outport  Port=25  OutDataTypeStr=UInt16  PortDimensions=1
  IMAPve_d_EPS_TrqLim_State : Outport  Port=26  OutDataTypeStr=UInt16  PortDimensions=1
  IMAPve_g_EPS_LKA_Current : Outport  Port=27  OutDataTypeStr=T_M_Nm_Float32  PortDimensions=1
  IMAPve_g_ESC_LatAcc : Outport  Port=28  OutDataTypeStr=T_M_Nm_Float32  PortDimensions=1
  IMAPve_d_ESC_LatAcc_Valid : Outport  Port=29  OutDataTypeStr=UInt16  PortDimensions=1
  IMAPve_g_ESC_YawRate : Outport  Port=30  OutDataTypeStr=T_M_Nm_Float32  PortDimensions=1
  IMAPve_d_ESC_YawRate_Valid : Outport  Port=31  OutDataTypeStr=UInt16  PortDimensions=1
  IMAPve_g_ESC_UnYawRate : Outport  Port=32  OutDataTypeStr=T_M_Nm_Float32  PortDimensions=1
  IMAPve_g_ESC_VehSpd : Outport  Port=33  OutDataTypeStr=T_M_Nm_Float32  PortDimensions=1
  IMAPve_g_ESC_LonAcc : Outport  Port=34  OutDataTypeStr=T_M_Nm_Float32  PortDimensions=1
  IMAPve_d_ESC_LonAcc_Valid : Outport  Port=35  OutDataTypeStr=UInt16  PortDimensions=1
  IMAPve_g_ESC_Brake_Press : Outport  Port=36  OutDataTypeStr=T_M_Nm_Float32  PortDimensions=1
  IMAPve_g_ESC_Static_Slope : Outport  Port=37  OutDataTypeStr=T_M_Nm_Float32  PortDimensions=1
  IMAPve_g_ESC_DySlope_Accuracy : Outport  Port=38  OutDataTypeStr=T_M_Nm_Float32  PortDimensions=1
  IMAPve_g_ESC_DySlope : Outport  Port=39  OutDataTypeStr=T_M_Nm_Float32  PortDimensions=1
  IMAPve_g_SW_Angle : Outport  Port=40  OutDataTypeStr=T_M_Nm_Float32  PortDimensions=1
  IMAPve_g_SW_Angle_Speed : Outport  Port=41  OutDataTypeStr=T_M_Nm_Float32  PortDimensions=1
  IMAPve_d_BCM_HazardLamp : Outport  Port=42  OutDataTypeStr=UInt16  PortDimensions=1
  IMAPve_d_BCM_Left_Light : Outport  Port=43  OutDataTypeStr=UInt16  PortDimensions=1
  IMAPve_d_BCM_Right_Light : Outport  Port=44  OutDataTypeStr=UInt16  PortDimensions=1
  IMAPve_d_ESC_BrakeLamp_Req : Outport  Port=45  OutDataTypeStr=UInt16  PortDimensions=1
  IMAPve_d_BCM_Opening_State : Outport  Port=46  OutDataTypeStr=UInt16  PortDimensions=1
  IMAPve_d_BCM_Trunk_State : Outport  Port=47  OutDataTypeStr=UInt16  PortDimensions=1
  IMAPve_d_BCM_LF_Door_State : Outport  Port=48  OutDataTypeStr=UInt16  PortDimensions=1
  IMAPve_d_BCM_RF_Door_State : Outport  Port=49  OutDataTypeStr=UInt16  PortDimensions=1
  IMAPve_d_BCM_RR_Door_State : Outport  Port=50  OutDataTypeStr=UInt16  PortDimensions=1
  IMAPve_d_BCM_LR_Door_State : Outport  Port=51  OutDataTypeStr=UInt16  PortDimensions=1
  IMAPve_d_SCC_Left_SwitchSig : Outport  Port=52  OutDataTypeStr=UInt16  PortDimensions=1
  IMAPve_d_SCC_Right_SwitchSig : Outport  Port=53  OutDataTypeStr=UInt16  PortDimensions=1
  IMAPve_d_BCM_HazardLamp_Switch : Outport  Port=54  OutDataTypeStr=UInt16
  IMAPve_d_PEPS_Door_Lock_Req : Outport  Port=55  OutDataTypeStr=UInt16  PortDimensions=1
  IMAPve_d_BCM_Door_Lock_State : Outport  Port=56  OutDataTypeStr=UInt16  PortDimensions=1
  IMAPve_d_EMS_ACC_Status : Outport  Port=57  OutDataTypeStr=UInt16  PortDimensions=1
  IMAPve_g_EMS_Pot_WhlT_Max : Outport  Port=58  OutDataTypeStr=T_M_Nm_Float32  PortDimensions=1
  IMAPve_g_EMS_Pot_WhlT_Min : Outport  Port=59  OutDataTypeStr=T_M_Nm_Float32  PortDimensions=1
  IMAPve_g_EMS_RealPedal : Outport  Port=60  OutDataTypeStr=T_M_Nm_Float32  PortDimensions=1
  IMAPve_g_EMS_MaxTWhl : Outport  Port=61  OutDataTypeStr=T_M_Nm_Float32  PortDimensions=1
  IMAPve_g_EMS_MaxTWhl_Offset : Outport  Port=62  OutDataTypeStr=T_M_Nm_Float32  PortDimensions=1
  IMAPve_g_EMS_MinTWhl : Outport  Port=63  OutDataTypeStr=T_M_Nm_Float32  PortDimensions=1
  IMAPve_g_EMS_MinTWhl_Offset : Outport  Port=64  OutDataTypeStr=T_M_Nm_Float32  PortDimensions=1
  IMAPve_g_EMS_Actual_FlwT : Outport  Port=65  OutDataTypeStr=T_M_Nm_Float32  PortDimensions=1
  IMAPve_g_EMS_Actual_IndT : Outport  Port=66  OutDataTypeStr=T_M_Nm_Float32  PortDimensions=1
  IMAPve_g_EMS_Realize_TWhl : Outport  Port=67  OutDataTypeStr=T_M_Nm_Float32  PortDimensions=1
  IMAPve_g_EMS_ACC_VirtualPedal : Outport  Port=68  OutDataTypeStr=T_M_Nm_Float32  PortDimensions=1
  IMAPve_d_EMS_AccPedal_Fault : Outport  Port=69  OutDataTypeStr=UInt16  PortDimensions=1
  IMAPve_g_EMS_Driver_Torque : Outport  Port=70  OutDataTypeStr=T_M_Nm_Float32  PortDimensions=1
  IMAPve_d_ESC_Brake_Effort : Outport  Port=71  OutDataTypeStr=UInt16  PortDimensions=1
  IMAPve_g_EMS_Engine_Speed : Outport  Port=72  OutDataTypeStr=T_M_Nm_Float32  PortDimensions=1
  IMAPve_d_ESC_Veh_Standstill : Outport  Port=73  OutDataTypeStr=UInt16  PortDimensions=1
  IMAPve_d_TCU_Actual_Gear : Outport  Port=74  OutDataTypeStr=UInt16  PortDimensions=1
  IMAPve_d_TCU_Target_Gear : Outport  Port=75  OutDataTypeStr=UInt16  PortDimensions=1
  IMAPve_d_TCU_PRND_State : Outport  Port=76  OutDataTypeStr=UInt16  PortDimensions=1
  IMAPve_d_BCM_Ignition_State : Outport  Port=77  OutDataTypeStr=UInt16  PortDimensions=1
  IMAPve_d_ACU_Driver_Belt : Outport  Port=78  OutDataTypeStr=UInt16  PortDimensions=1
  IMAPve_d_SWS_Failure_Status : Outport  Port=79  OutDataTypeStr=UInt16  PortDimensions=1
  IMAPve_d_ESC_OFF : Outport  Port=80  OutDataTypeStr=UInt16  PortDimensions=1
  IMAPve_d_ESC_AlarmSig : Outport  Port=81  OutDataTypeStr=UInt16  PortDimensions=1
  IMAPve_d_ESC_ESC_Active : Outport  Port=82  OutDataTypeStr=UInt16  PortDimensions=1
  IMAPve_d_ESC_MSR_Active : Outport  Port=83  OutDataTypeStr=UInt16  PortDimensions=1
  IMAPve_d_ESC_TCS_Active : Outport  Port=84  OutDataTypeStr=UInt16  PortDimensions=1
  IMAPve_d_ESC_VehSpd_Valid : Outport  Port=85  OutDataTypeStr=UInt16  PortDimensions=1
  IMAPve_d_ESC_ABS_Active : Outport  Port=86  OutDataTypeStr=UInt16  PortDimensions=1
  IMAPve_d_ESC_ABS_Valid : Outport  Port=87  OutDataTypeStr=UInt16  PortDimensions=1
  IMAPve_d_ESC_ABS_AlarmSig : Outport  Port=88  OutDataTypeStr=UInt16  PortDimensions=1
  IMAPve_d_ESC_FL_WheelPulVal : Outport  Port=89  OutDataTypeStr=UInt16  PortDimensions=1
  IMAPve_d_ESC_FR_WheelPulVal : Outport  Port=90  OutDataTypeStr=UInt16  PortDimensions=1
  IMAPve_d_ESC_RL_WheelPulVal : Outport  Port=91  OutDataTypeStr=UInt16  PortDimensions=1
  IMAPve_d_ESC_RR_WheelPulVal : Outport  Port=92  OutDataTypeStr=UInt16  PortDimensions=1
  IMAPve_g_ESC_FL_WhlSpd : Outport  Port=93  OutDataTypeStr=T_M_Nm_Float32  PortDimensions=1
  IMAPve_d_ESC_FL_WhlSpd_Fault : Outport  Port=94  OutDataTypeStr=UInt16  PortDimensions=1
  IMAPve_g_ESC_FR_WhlSpd : Outport  Port=95  OutDataTypeStr=T_M_Nm_Float32  PortDimensions=1
  IMAPve_d_ESC_FR_WhlSpd_Fault : Outport  Port=96  OutDataTypeStr=UInt16  PortDimensions=1
  IMAPve_g_ESC_RL_WhlSpd : Outport  Port=97  OutDataTypeStr=T_M_Nm_Float32  PortDimensions=1
  IMAPve_d_ESC_RL_WhlSpd_Fault : Outport  Port=98  OutDataTypeStr=UInt16  PortDimensions=1
  IMAPve_g_ESC_RR_WhlSpd : Outport  Port=99  OutDataTypeStr=T_M_Nm_Float32  PortDimensions=1
  IMAPve_d_ESC_RR_WhlSpd_Fault : Outport  Port=100  OutDataTypeStr=UInt16  PortDimensions=1
  IMAPve_d_ESC_FL_Wheel_Pulse : Outport  Port=101  OutDataTypeStr=UInt16  PortDimensions=1
  IMAPve_d_ESC_FR_Wheel_Pulse : Outport  Port=102  OutDataTypeStr=UInt16  PortDimensions=1
  IMAPve_d_ESC_RL_Wheel_Pulse : Outport  Port=103  OutDataTypeStr=UInt16  PortDimensions=1
  IMAPve_d_ESC_RR_Wheel_Pulse : Outport  Port=104  OutDataTypeStr=UInt16  PortDimensions=1
  IMAPve_d_TCU_AT_Failure : Outport  Port=105  OutDataTypeStr=UInt16  PortDimensions=1
  IMAPve_d_TCU_Shift_Valid : Outport  Port=106  OutDataTypeStr=UInt16  PortDimensions=1
  IMAPve_d_TCU_DCT_Clutch_State : Outport  Port=107  OutDataTypeStr=UInt16  PortDimensions=1
  IMAPve_d_TCU_Gear_Engage : Outport  Port=108  OutDataTypeStr=UInt16  PortDimensions=1
  IMAPve_d_TCU_Select_ATMode : Outport  Port=109  OutDataTypeStr=UInt16  PortDimensions=1
  IMAPve_d_EMS_Engine_Status : Outport  Port=110  OutDataTypeStr=UInt16  PortDimensions=1
  IMAPve_d_EMS_Gearbox_CtlAvail : Outport  Port=111  OutDataTypeStr=UInt16  PortDimensions=1
  IMAPve_d_ESC_Brake_Failsafe : Outport  Port=112  OutDataTypeStr=UInt16  PortDimensions=1
  IMAPve_d_ESC_AEB_Available : Outport  Port=113  OutDataTypeStr=UInt16  PortDimensions=1
  IMAPve_d_ESC_AEB_Active : Outport  Port=114  OutDataTypeStr=UInt16  PortDimensions=1
  IMAPve_d_ESC_ACC_Available : Outport  Port=115  OutDataTypeStr=UInt16  PortDimensions=1
  IMAPve_d_ESC_ACC_Active : Outport  Port=116  OutDataTypeStr=UInt16  PortDimensions=1
  IMAPve_d_EMS_ACC_Effective : Outport  Port=117  OutDataTypeStr=UInt16  PortDimensions=1
  IMAPve_d_BCM_FrontWiper_State : Outport  Port=118  OutDataTypeStr=UInt16  PortDimensions=1
  IMAPve_d_BCM_CHMSL_Status : Outport  Port=119  OutDataTypeStr=UInt16  PortDimensions=1
  IMAPve_d_BCM_BrakeLamp_State : Outport  Port=120  OutDataTypeStr=UInt16  PortDimensions=1
  IMAPve_d_ACU_Passenger_Belt : Outport  Port=121  OutDataTypeStr=UInt16  PortDimensions=1
  IMAPve_d_EMS_ACC_CtlAvail : Outport  Port=122  OutDataTypeStr=UInt16  PortDimensions=1
  IMAPve_d_EMS_ACC_Inhibited : Outport  Port=123  OutDataTypeStr=UInt16  PortDimensions=1
  IMAPve_d_EMS_Brake_Pedal : Outport  Port=124  OutDataTypeStr=UInt16  PortDimensions=1
  IMAPve_d_BCM_LowBeam_State : Outport  Port=125  OutDataTypeStr=UInt16  PortDimensions=1
  IMAPve_d_BCM_HighBeam_State : Outport  Port=126  OutDataTypeStr=UInt16  PortDimensions=1
  IMAPve_d_EPB_Status : Outport  Port=127  OutDataTypeStr=UInt16  PortDimensions=1
  IMAPve_d_EPB_Display_Req : Outport  Port=128  OutDataTypeStr=UInt16  PortDimensions=1
  IMAPve_d_EPB_Warn_Req : Outport  Port=129  OutDataTypeStr=UInt16  PortDimensions=1
  IMAPve_d_EPB_Switch_State : Outport  Port=130  OutDataTypeStr=UInt16  PortDimensions=1
  IMAPve_d_EPB_Switch_Valid : Outport  Port=131  OutDataTypeStr=UInt16  PortDimensions=1
  IMAPve_d_ESC_Drive_Direction : Outport  Port=132  OutDataTypeStr=UInt16  PortDimensions=1
  IMAPve_d_ESC_Hold_State : Outport  Port=133  OutDataTypeStr=UInt16  PortDimensions=1
  IMAPve_d_EPS_Steer_Hold_State : Outport  Port=134  OutDataTypeStr=UInt16  PortDimensions=1
  IMAPve_d_EPS_Warning_State : Outport  Port=135  OutDataTypeStr=UInt16  PortDimensions=1
  IMAPve_g_EPS_PowerCon : Outport  Port=136  OutDataTypeStr=T_M_Nm_Float32  PortDimensions=1
  IMAPve_d_ESC_EBD_AlarmSig : Outport  Port=137  OutDataTypeStr=UInt16  PortDimensions=1
  IMAPve_d_ESC_AVH_Status : Outport  Port=138  OutDataTypeStr=UInt16  PortDimensions=1
  IMAPve_g_BCM_Battery_Voltage : Outport  Port=139  OutDataTypeStr=T_M_Nm_Float32  PortDimensions=1
  IMAPve_d_TBOX_LocalTimeY : Outport  Port=140  OutDataTypeStr=UInt16  PortDimensions=1
  IMAPve_d_TBOX_LocalTimeM : Outport  Port=141  OutDataTypeStr=UInt16  PortDimensions=1
  IMAPve_d_TBOX_LocalTimeD : Outport  Port=142  OutDataTypeStr=UInt16  PortDimensions=1
  IMAPve_d_TBOX_LocalTimeH : Outport  Port=143  OutDataTypeStr=UInt16  PortDimensions=1
  IMAPve_d_TBOX_LocalTimeMin : Outport  Port=144  OutDataTypeStr=UInt16  PortDimensions=1
  IMAPve_d_TBOX_LocalTimeS : Outport  Port=145  OutDataTypeStr=UInt16  PortDimensions=1
  IMAPve_d_TBOX_LocalTime_Valid : Outport  Port=146  OutDataTypeStr=UInt16  PortDimensions=1
  IMAPve_d_Radar_State : Outport  Port=147  OutDataTypeStr=UInt16  PortDimensions=1
  IMAPve_d_Time_System_Clock : Outport  Port=148  OutDataTypeStr=UInt16  PortDimensions=1
  IMAPve_g_GW_IC_Odometer : Outport  Port=149  OutDataTypeStr=UInt32  PortDimensions=1
  IMAPve_d_Outside_Temp : Outport  Port=150  OutDataTypeStr=UInt16  PortDimensions=1
  IMAPve_d_ORI_CIPV_ID : Outport  Port=151  OutDataTypeStr=UInt16  PortDimensions=1
  IMAPve_d_ORI_Obj_Num : Outport  Port=152  OutDataTypeStr=UInt16  PortDimensions=1
  IMAPva_d_ORI_Obj_Class : Outport  Port=153  OutDataTypeStr=UInt16  PortDimensions=20
  IMAPva_g_ORI_Obj_RelVel : Outport  Port=154  OutDataTypeStr=T_M_Nm_Float32  PortDimensions=20
  IMAPva_g_ORI_Obj_LongDis : Outport  Port=155  OutDataTypeStr=T_M_Nm_Float32  PortDimensions=20
  IMAPva_g_ORI_Obj_LAngle : Outport  Port=156  OutDataTypeStr=T_M_Nm_Float32  PortDimensions=20
  IMAPva_g_ORI_Obj_RAngle : Outport  Port=157  OutDataTypeStr=T_M_Nm_Float32  PortDimensions=20
  IMAPva_g_ORI_Obj_Width : Outport  Port=158  OutDataTypeStr=T_M_Nm_Float32  PortDimensions=20
  IMAPva_d_ORI_Obj_ID : Outport  Port=159  OutDataTypeStr=UInt16  PortDimensions=20
  IMAPve_g_ORI_L0_C3 : Outport  Port=160  OutDataTypeStr=T_M_Nm_Float32  PortDimensions=1
  IMAPve_g_ORI_L0_C2 : Outport  Port=161  OutDataTypeStr=T_M_Nm_Float32  PortDimensions=1
  IMAPve_g_ORI_L0_C1 : Outport  Port=162  OutDataTypeStr=T_M_Nm_Float32  PortDimensions=1
  IMAPve_g_ORI_L0_C0 : Outport  Port=163  OutDataTypeStr=T_M_Nm_Float32  PortDimensions=1
  IMAPve_d_ORI_L0_Type : Outport  Port=164  OutDataTypeStr=UInt16  PortDimensions=1
  IMAPve_g_ORI_L0_VR : Outport  Port=165  OutDataTypeStr=T_M_Nm_Float32  PortDimensions=1
  IMAPve_g_ORI_L0_W : Outport  Port=166  OutDataTypeStr=T_M_Nm_Float32  PortDimensions=1
  IMAPve_g_ORI_L1_C3 : Outport  Port=167  OutDataTypeStr=T_M_Nm_Float32  PortDimensions=1
  IMAPve_g_ORI_L1_C2 : Outport  Port=168  OutDataTypeStr=T_M_Nm_Float32  PortDimensions=1
  IMAPve_g_ORI_L1_C1 : Outport  Port=169  OutDataTypeStr=T_M_Nm_Float32  PortDimensions=1
  IMAPve_g_ORI_L1_C0 : Outport  Port=170  OutDataTypeStr=T_M_Nm_Float32  PortDimensions=1
  IMAPve_d_ORI_L1_Type : Outport  Port=171  OutDataTypeStr=UInt16  PortDimensions=1
  IMAPve_g_ORI_L1_VR : Outport  Port=172  OutDataTypeStr=T_M_Nm_Float32  PortDimensions=1
  IMAPve_g_ORI_L1_W : Outport  Port=173  OutDataTypeStr=T_M_Nm_Float32  PortDimensions=1
  IMAPve_g_ORI_R0_C3 : Outport  Port=174  OutDataTypeStr=T_M_Nm_Float32  PortDimensions=1
  IMAPve_g_ORI_R0_C2 : Outport  Port=175  OutDataTypeStr=T_M_Nm_Float32  PortDimensions=1
  IMAPve_g_ORI_R0_C1 : Outport  Port=176  OutDataTypeStr=T_M_Nm_Float32  PortDimensions=1
  IMAPve_g_ORI_R0_C0 : Outport  Port=177  OutDataTypeStr=T_M_Nm_Float32  PortDimensions=1
  IMAPve_d_ORI_R0_LT : Outport  Port=178  OutDataTypeStr=UInt16  PortDimensions=1
  IMAPve_g_ORI_R0_VR : Outport  Port=179  OutDataTypeStr=T_M_Nm_Float32  PortDimensions=1
  IMAPve_g_ORI_R0_W : Outport  Port=180  OutDataTypeStr=T_M_Nm_Float32  PortDimensions=1
  IMAPve_g_ORI_R1_C3 : Outport  Port=181  OutDataTypeStr=T_M_Nm_Float32  PortDimensions=1
  IMAPve_g_ORI_R1_C2 : Outport  Port=182  OutDataTypeStr=T_M_Nm_Float32  PortDimensions=1
  IMAPve_g_ORI_R1_C1 : Outport  Port=183  OutDataTypeStr=T_M_Nm_Float32  PortDimensions=1
  IMAPve_g_ORI_R1_C0 : Outport  Port=184  OutDataTypeStr=T_M_Nm_Float32  PortDimensions=1
  IMAPve_d_ORI_R1_LT : Outport  Port=185  OutDataTypeStr=UInt16  PortDimensions=1
  IMAPve_g_ORI_R1_VR : Outport  Port=186  OutDataTypeStr=T_M_Nm_Float32  PortDimensions=1
  IMAPve_g_ORI_R1_W : Outport  Port=187  OutDataTypeStr=T_M_Nm_Float32  PortDimensions=1
  IMAPve_d_Sensor_Status : Outport  Port=188  OutDataTypeStr=UInt16  PortDimensions=1
  IMAPve_d_LF_Radar_Status : Outport  Port=189  OutDataTypeStr=UInt16  PortDimensions=1
  IMAPve_d_RF_Radar_Status : Outport  Port=190  OutDataTypeStr=UInt16  PortDimensions=1
  IMAPve_d_LR_Radar_Status : Outport  Port=191  OutDataTypeStr=UInt16  PortDimensions=1
  IMAPve_d_RR_Radar_Status : Outport  Port=192  OutDataTypeStr=UInt16  PortDimensions=1
  IMAPve_d_Fusion_Status : Outport  Port=193  OutDataTypeStr=UInt16  PortDimensions=1
  IMAPve_d_Fusion_Time_Stamp : Outport  Port=194  OutDataTypeStr=UInt16  PortDimensions=1
  IMAPve_d_obj_Num : Outport  Port=195  OutDataTypeStr=UInt16  PortDimensions=1
  IMAPva_d_obj_id : Outport  Port=196  OutDataTypeStr=UInt16  PortDimensions=40
  IMAPva_g_obj_pos_x : Outport  Port=197  OutDataTypeStr=T_M_Nm_Float32  PortDimensions=40
  IMAPva_g_obj_pos_y : Outport  Port=198  OutDataTypeStr=T_M_Nm_Float32  PortDimensions=40
  IMAPva_g_obj_vel_x : Outport  Port=199  OutDataTypeStr=T_M_Nm_Float32  PortDimensions=40
  IMAPva_g_obj_vel_y : Outport  Port=200  OutDataTypeStr=T_M_Nm_Float32  PortDimensions=40
  IMAPva_g_obj_acc_x : Outport  Port=201  OutDataTypeStr=T_M_Nm_Float32  PortDimensions=40
  IMAPva_g_obj_acc_y : Outport  Port=202  OutDataTypeStr=T_M_Nm_Float32  PortDimensions=40
  IMAPva_g_obj_pos_var_x : Outport  Port=203  OutDataTypeStr=T_M_Nm_Float32  PortDimensions=40
  IMAPva_g_obj_pos_var_y : Outport  Port=204  OutDataTypeStr=T_M_Nm_Float32  PortDimensions=40
  IMAPva_g_obj_pos_var_xy : Outport  Port=205  OutDataTypeStr=T_M_Nm_Float32  PortDimensions=40
  IMAPva_g_obj_width : Outport  Port=206  OutDataTypeStr=T_M_Nm_Float32  PortDimensions=40
  IMAPva_g_obj_length : Outport  Port=207  OutDataTypeStr=T_M_Nm_Float32  PortDimensions=40
  IMAPva_d_obj_class : Outport  Port=208  OutDataTypeStr=UInt16  PortDimensions=40
  IMAPva_d_obj_lane : Outport  Port=209  OutDataTypeStr=UInt16  PortDimensions=40
  IMAPva_d_obj_status : Outport  Port=210  OutDataTypeStr=UInt16  PortDimensions=40
  IMAPva_d_obj_age : Outport  Port=211  OutDataTypeStr=UInt16  PortDimensions=40
  IMAPva_d_obj_TurnLight : Outport  Port=212  OutDataTypeStr=UInt16  PortDimensions=40
  IMAPva_d_obj_BrakeLight : Outport  Port=213  OutDataTypeStr=UInt16  PortDimensions=40
  IMAPva_d_obj_MotionStatus : Outport  Port=214  OutDataTypeStr=UInt16  PortDimensions=40
  IMAPve_d_Road_Type : Outport  Port=215  OutDataTypeStr=UInt16  PortDimensions=1
  IMAPve_g_L0_C0 : Outport  Port=216  OutDataTypeStr=T_M_Nm_Float32  PortDimensions=1
  IMAPve_g_L0_C1 : Outport  Port=217  OutDataTypeStr=T_M_Nm_Float32  PortDimensions=1
  IMAPve_g_L0_C2 : Outport  Port=218  OutDataTypeStr=T_M_Nm_Float32  PortDimensions=1
  IMAPve_g_L0_C3 : Outport  Port=219  OutDataTypeStr=T_M_Nm_Float32  PortDimensions=1
  IMAPve_g_L0_VR : Outport  Port=220  OutDataTypeStr=T_M_Nm_Float32  PortDimensions=1
  IMAPve_d_L0_Q : Outport  Port=221  OutDataTypeStr=UInt16  PortDimensions=1
  IMAPve_d_L0_Type : Outport  Port=222  OutDataTypeStr=UInt16  PortDimensions=1
  IMAPve_g_L0_W : Outport  Port=223  OutDataTypeStr=T_M_Nm_Float32  PortDimensions=1
  IMAPve_g_R0_C0 : Outport  Port=224  OutDataTypeStr=T_M_Nm_Float32  PortDimensions=1
  IMAPve_g_R0_C1 : Outport  Port=225  OutDataTypeStr=T_M_Nm_Float32  PortDimensions=1
  IMAPve_g_R0_C2 : Outport  Port=226  OutDataTypeStr=T_M_Nm_Float32  PortDimensions=1
  IMAPve_g_R0_C3 : Outport  Port=227  OutDataTypeStr=T_M_Nm_Float32  PortDimensions=1
  IMAPve_g_R0_VR : Outport  Port=228  OutDataTypeStr=T_M_Nm_Float32  PortDimensions=1
  IMAPve_d_R0_Q : Outport  Port=229  OutDataTypeStr=UInt16  PortDimensions=1
  IMAPve_d_R0_Type : Outport  Port=230  OutDataTypeStr=UInt16  PortDimensions=1
  IMAPve_g_R0_W : Outport  Port=231  OutDataTypeStr=T_M_Nm_Float32  PortDimensions=1
  IMAPve_g_L1_C0 : Outport  Port=232  OutDataTypeStr=T_M_Nm_Float32  PortDimensions=1
  IMAPve_g_L1_C1 : Outport  Port=233  OutDataTypeStr=T_M_Nm_Float32  PortDimensions=1
  IMAPve_g_L1_C2 : Outport  Port=234  OutDataTypeStr=T_M_Nm_Float32  PortDimensions=1
  IMAPve_g_L1_C3 : Outport  Port=235  OutDataTypeStr=T_M_Nm_Float32  PortDimensions=1
  IMAPve_g_L1_VR : Outport  Port=236  OutDataTypeStr=T_M_Nm_Float32  PortDimensions=1
  IMAPve_d_L1_Q : Outport  Port=237  OutDataTypeStr=UInt16  PortDimensions=1
  IMAPve_d_L1_Type : Outport  Port=238  OutDataTypeStr=UInt16  PortDimensions=1
  IMAPve_g_L1_W : Outport  Port=239  OutDataTypeStr=T_M_Nm_Float32  PortDimensions=1
  IMAPve_g_R1_C0 : Outport  Port=240  OutDataTypeStr=T_M_Nm_Float32  PortDimensions=1
  IMAPve_g_R1_C1 : Outport  Port=241  OutDataTypeStr=T_M_Nm_Float32  PortDimensions=1
  IMAPve_g_R1_C2 : Outport  Port=242  OutDataTypeStr=T_M_Nm_Float32  PortDimensions=1
  IMAPve_g_R1_C3 : Outport  Port=243  OutDataTypeStr=T_M_Nm_Float32  PortDimensions=1
  IMAPve_g_R1_VR : Outport  Port=244  OutDataTypeStr=T_M_Nm_Float32  PortDimensions=1
  IMAPve_d_R1_Q : Outport  Port=245  OutDataTypeStr=UInt16  PortDimensions=1
  IMAPve_d_R1_Type : Outport  Port=246  OutDataTypeStr=UInt16  PortDimensions=1
  IMAPve_g_R1_W : Outport  Port=247  OutDataTypeStr=T_M_Nm_Float32  PortDimensions=1
  IMAPve_g_L0_C0_Back : Outport  Port=248  OutDataTypeStr=T_M_Nm_Float32  PortDimensions=1
  IMAPve_g_L0_C1_Back : Outport  Port=249  OutDataTypeStr=T_M_Nm_Float32  PortDimensions=1
  IMAPve_g_L0_C2_Back : Outport  Port=250  OutDataTypeStr=T_M_Nm_Float32  PortDimensions=1
  IMAPve_g_L0_C3_Back : Outport  Port=251  OutDataTypeStr=T_M_Nm_Float32  PortDimensions=1
  IMAPve_g_L0_Range_Back : Outport  Port=252  OutDataTypeStr=T_M_Nm_Float32  PortDimensions=1
  IMAPve_g_R0_C0_Back : Outport  Port=253  OutDataTypeStr=T_M_Nm_Float32  PortDimensions=1
  IMAPve_g_R0_C1_Back : Outport  Port=254  OutDataTypeStr=T_M_Nm_Float32  PortDimensions=1
  IMAPve_g_R0_C2_Back : Outport  Port=255  OutDataTypeStr=T_M_Nm_Float32  PortDimensions=1
  IMAPve_g_R0_C3_Back : Outport  Port=256  OutDataTypeStr=T_M_Nm_Float32  PortDimensions=1
  IMAPve_g_R0_Range_Back : Outport  Port=257  OutDataTypeStr=T_M_Nm_Float32  PortDimensions=1
  IMAPve_g_L1_C0_Back : Outport  Port=258  OutDataTypeStr=T_M_Nm_Float32  PortDimensions=1
  IMAPve_g_L1_C1_Back : Outport  Port=259  OutDataTypeStr=T_M_Nm_Float32  PortDimensions=1
  IMAPve_g_L1_C2_Back : Outport  Port=260  OutDataTypeStr=T_M_Nm_Float32  PortDimensions=1
  IMAPve_g_L1_C3_Back : Outport  Port=261  OutDataTypeStr=T_M_Nm_Float32  PortDimensions=1
  IMAPve_g_L1_Range_Back : Outport  Port=262  OutDataTypeStr=T_M_Nm_Float32  PortDimensions=1
  IMAPve_g_R1_C0_Back : Outport  Port=263  OutDataTypeStr=T_M_Nm_Float32  PortDimensions=1
  IMAPve_g_R1_C1_Back : Outport  Port=264  OutDataTypeStr=T_M_Nm_Float32  PortDimensions=1
  IMAPve_g_R1_C2_Back : Outport  Port=265  OutDataTypeStr=T_M_Nm_Float32  PortDimensions=1
  IMAPve_g_R1_C3_Back : Outport  Port=266  OutDataTypeStr=T_M_Nm_Float32  PortDimensions=1
  IMAPve_g_R1_Range_Back : Outport  Port=267  OutDataTypeStr=T_M_Nm_Float32  PortDimensions=1
  IMAPve_g_Lrg_C0_BACK : Outport  Port=268  OutDataTypeStr=T_M_Nm_Float32
  IMAPve_g_Lrg_C1_BACK : Outport  Port=269  OutDataTypeStr=T_M_Nm_Float32
  IMAPve_g_Lrg_C2_BACK : Outport  Port=270  OutDataTypeStr=T_M_Nm_Float32
  IMAPve_g_Lrg_C3_BACK : Outport  Port=271  OutDataTypeStr=T_M_Nm_Float32
  IMAPve_g_Lrg_VR_Start_BACK : Outport  Port=272  OutDataTypeStr=T_M_Nm_Float32
  IMAPve_g_Lrg_VR_End_BACK : Outport  Port=273  OutDataTypeStr=T_M_Nm_Float32
  IMAPve_d_Lrg_Q_BACK : Outport  Port=274  OutDataTypeStr=UInt16
  IMAPve_d_Lrg_TYPE_BACK : Outport  Port=275  OutDataTypeStr=UInt16
  IMAPve_g_Rrg_C0_BACK : Outport  Port=276  OutDataTypeStr=T_M_Nm_Float32
  IMAPve_g_Rrg_C1_BACK : Outport  Port=277  OutDataTypeStr=T_M_Nm_Float32
  IMAPve_g_Rrg_C2_BACK : Outport  Port=278  OutDataTypeStr=T_M_Nm_Float32
  IMAPve_g_Rrg_C3_BACK : Outport  Port=279  OutDataTypeStr=T_M_Nm_Float32
  IMAPve_g_Rrg_VR_Start_BACK : Outport  Port=280  OutDataTypeStr=T_M_Nm_Float32
  IMAPve_g_Rrg_VR_End_BACK : Outport  Port=281  OutDataTypeStr=T_M_Nm_Float32
  IMAPve_d_Rrg_Q_BACK : Outport  Port=282  OutDataTypeStr=UInt16
  IMAPve_d_Rrg_TYPE_BACK : Outport  Port=283  OutDataTypeStr=UInt16
  IMAPve_d_Sign_ISA_Value : Outport  Port=284  OutDataTypeStr=UInt16  PortDimensions=1
  IMAPve_d_ISA_Popup_Message : Outport  Port=285  OutDataTypeStr=UInt16
  IMAPve_d_ISA_Sign_Type : Outport  Port=286  OutDataTypeStr=UInt16
  IMAPve_d_ISA_Status : Outport  Port=287  OutDataTypeStr=UInt16
  IMAPve_d_TSR_Sign_Type : Outport  Port=288  OutDataTypeStr=UInt16  PortDimensions=1
  IMAPve_g_Camera_Signal_Fault : Outport  Port=289  OutDataTypeStr=T_M_Nm_Float32  PortDimensions=1
  IMAPve_d_Camera_State : Outport  Port=290  OutDataTypeStr=UInt16  PortDimensions=1
  IMAPve_d_Radar_FaultBitSetting_Signal : Outport  Port=291
  IMAPve_d_Camera_Status : Outport  Port=292  OutDataTypeStr=UInt16  PortDimensions=1
  IMAPve_d_ESC_FLW_Direction : Outport  Port=293  OutDataTypeStr=UInt16
  IMAPve_d_ESC_FRW_Direction : Outport  Port=294  OutDataTypeStr=UInt16
  IMAPve_d_ESC_TCS_ErrorStatus : Outport  Port=295  OutDataTypeStr=UInt16
  IMAPve_d_ESC_RLW_Direction : Outport  Port=296  OutDataTypeStr=UInt16
  IMAPve_d_ESC_RRW_Direction : Outport  Port=297  OutDataTypeStr=UInt16
  IMAPve_d_ESC_EPB_ErrorStatus : Outport  Port=298  OutDataTypeStr=UInt16
  IMAPve_d_EPS_SteeringAngle_Flag : Outport  Port=299  OutDataTypeStr=UInt16
  IMAPve_g_EPS_SteeringAngle : Outport  Port=300  OutDataTypeStr=T_M_Nm_Float32
  IMAPve_d_EPS_Driver_Override : Outport  Port=301  OutDataTypeStr=UInt16
  IMAPve_d_EPS_Driver_Active_ESA : Outport  Port=302  OutDataTypeStr=UInt16
  IMAPve_d_EPS_ESA_State : Outport  Port=303  OutDataTypeStr=UInt16
  IMAPve_d_ACU_RearLeft_Belt : Outport  Port=304  OutDataTypeStr=UInt16
  IMAPve_d_ACU_RearMiddle_Belt : Outport  Port=305  OutDataTypeStr=UInt16
  IMAPve_d_ACU_RearRight_Belt : Outport  Port=306  OutDataTypeStr=UInt16
  IMAPve_d_EMS_PowertrainCtl_State : Outport  Port=307  OutDataTypeStr=UInt16
  IMAPve_d_TCU_TCU_Available : Outport  Port=308  OutDataTypeStr=UInt16
  IMAPve_d_BCM_LeftTurn_Switch : Outport  Port=309  OutDataTypeStr=UInt16
  IMAPve_d_BCM_RightTurn_Switch : Outport  Port=310  OutDataTypeStr=UInt16
  IMAPve_d_BCM_FrontWiper_Switch : Outport  Port=311  OutDataTypeStr=UInt16
  IMAPve_d_BCM_IHBC_Enabled : Outport  Port=312  OutDataTypeStr=UInt16
  IMAPve_d_MP5_Work_State : Outport  Port=313  OutDataTypeStr=UInt16
  IMAPve_d_MP5_APA_ModeSelect : Outport  Port=314  OutDataTypeStr=UInt16
  IMAPve_d_MP5_LanguageSet : Outport  Port=315  OutDataTypeStr=UInt16
  IMAPve_d_MP5_UPA_Switch : Outport  Port=316  OutDataTypeStr=UInt16
  IMAPve_d_MP5_FLK_Activation : Outport  Port=317  OutDataTypeStr=UInt16
  IMAPve_d_MP5_AutoPilot_Switch : Outport  Port=318  OutDataTypeStr=UInt16
  IMAPve_d_MP5_DMS_MessageType : Outport  Port=319  OutDataTypeStr=UInt16
  IMAPve_d_MP5_DMS_SystemEnable : Outport  Port=320  OutDataTypeStr=UInt16
  IMAPve_d_MP5_DMS_DelUserNum : Outport  Port=321  OutDataTypeStr=UInt16
  IMAPve_d_MP5_DMS_Sensity : Outport  Port=322  OutDataTypeStr=UInt16
  IMAPve_d_MP5_DMS_EyeFatigue : Outport  Port=323  OutDataTypeStr=UInt16
  IMAPve_d_MP5_DMS_LongtimeDrive : Outport  Port=324  OutDataTypeStr=UInt16
  IMAPve_d_MP5_DMS_SideView : Outport  Port=325  OutDataTypeStr=UInt16
  IMAPve_d_MP5_DMS_UsingPhone : Outport  Port=326  OutDataTypeStr=UInt16
  IMAPve_d_MP5_DMS_Smoking : Outport  Port=327  OutDataTypeStr=UInt16
  IMAPve_d_MP5_DMS_DrinkWater : Outport  Port=328  OutDataTypeStr=UInt16
  IMAPve_d_MP5_DMS_UserAccount : Outport  Port=329  OutDataTypeStr=UInt16
  IMAPve_g_ESC_BrkWhlCylinder_Pressure : Outport  Port=330  OutDataTypeStr=T_M_Nm_Float32
  IMAPva_d_ORI_Obj_TimeStamp : Outport  Port=331  OutDataTypeStr=UInt16  PortDimensions=20
  IMAPve_d_ORI_FS_OutOfCalib : Outport  Port=332  OutDataTypeStr=UInt16
  IMAPve_d_ORI_FS_Rain : Outport  Port=333  OutDataTypeStr=UInt16
  IMAPve_d_ORI_FS_Fog : Outport  Port=334  OutDataTypeStr=UInt16
  IMAPve_d_ORI_FS_Splashes0 : Outport  Port=335  OutDataTypeStr=UInt16
  IMAPve_d_ORI_FS_SunRay0 : Outport  Port=336  OutDataTypeStr=UInt16
  IMAPve_d_ORI_FS_LowSun0 : Outport  Port=337  OutDataTypeStr=UInt16
  IMAPve_d_ORI_FS_BlurImage0 : Outport  Port=338  OutDataTypeStr=UInt16
  IMAPve_d_ORI_FS_PartialBlockage0 : Outport  Port=339  OutDataTypeStr=UInt16
  IMAPve_d_ORI_FS_FullBlockage0 : Outport  Port=340  OutDataTypeStr=UInt16
  IMAPve_d_ORI_FS_FrozenWindshield0 : Outport  Port=341  OutDataTypeStr=UInt16
  IMAPve_d_ORI_FS_OutOfFocus0 : Outport  Port=342  OutDataTypeStr=UInt16
  IMAPva_g_ORI_Obj_AbsAx : Outport  Port=343  OutDataTypeStr=T_M_Nm_Float32  PortDimensions=20
  IMAPva_g_ORI_Obj_AbsAy : Outport  Port=344  OutDataTypeStr=T_M_Nm_Float32  PortDimensions=20
  IMAPva_g_ORI_Obj_TTIPCStdDev : Outport  Port=345  OutDataTypeStr=T_M_Nm_Float32  PortDimensions=20
  IMAPva_g_ORI_Obj_RelVely : Outport  Port=346  OutDataTypeStr=T_M_Nm_Float32  PortDimensions=20
  IMAPva_g_ORI_Obj_LateralDis : Outport  Port=347  OutDataTypeStr=T_M_Nm_Float32  PortDimensions=20
  IMAPva_g_ORI_Obj_AbsAxStdDev : Outport  Port=348  OutDataTypeStr=T_M_Nm_Float32  PortDimensions=20
  IMAPva_g_ORI_Obj_AbsAyStdDev : Outport  Port=349  OutDataTypeStr=T_M_Nm_Float32  PortDimensions=20
  IMAPva_g_ORI_Obj_RelVelStdDev : Outport  Port=350  OutDataTypeStr=T_M_Nm_Float32  PortDimensions=20
  IMAPva_g_ORI_Obj_RelVelyStdDev : Outport  Port=351  OutDataTypeStr=T_M_Nm_Float32  PortDimensions=20
  IMAPva_g_ORI_Obj_LongDisStdDev : Outport  Port=352  OutDataTypeStr=T_M_Nm_Float32  PortDimensions=20
  IMAPva_g_ORI_Obj_LateralDisStdDev : Outport  Port=353  OutDataTypeStr=T_M_Nm_Float32  PortDimensions=20
  IMAPva_d_ORI_Obj_RelVelValid : Outport  Port=354  OutDataTypeStr=UInt16  PortDimensions=20
  IMAPva_d_ORI_Obj_RelVelyValid : Outport  Port=355  OutDataTypeStr=UInt16  PortDimensions=20
  IMAPva_d_ORI_Obj_RelVelStdDevValid : Outport  Port=356  OutDataTypeStr=UInt16  PortDimensions=20
  IMAPva_d_ORI_Obj_RelVelyStdDevValid : Outport  Port=357  OutDataTypeStr=UInt16  PortDimensions=20
  IMAPva_g_ORI_Obj_ExistProb : Outport  Port=358  OutDataTypeStr=T_M_Nm_Float32  PortDimensions=20
  IMAPva_g_ORI_Obj_ClassProb : Outport  Port=359  OutDataTypeStr=T_M_Nm_Float32  PortDimensions=20
  IMAPva_g_ORI_Obj_Height : Outport  Port=360  OutDataTypeStr=T_M_Nm_Float32  PortDimensions=20
  IMAPva_g_ORI_Obj_LengthStdDev : Outport  Port=361  OutDataTypeStr=T_M_Nm_Float32  PortDimensions=20
  IMAPva_g_ORI_Obj_WidthStdDev : Outport  Port=362  OutDataTypeStr=T_M_Nm_Float32  PortDimensions=20
  IMAPva_g_ORI_Obj_HeightStdDev : Outport  Port=363  OutDataTypeStr=T_M_Nm_Float32  PortDimensions=20
  IMAPva_g_ORI_Obj_3DAngle : Outport  Port=364  OutDataTypeStr=T_M_Nm_Float32  PortDimensions=20
  IMAPva_g_ORI_Obj_LAngleStdDev : Outport  Port=365  OutDataTypeStr=T_M_Nm_Float32  PortDimensions=20
  IMAPva_g_ORI_Obj_RAngleStdDev : Outport  Port=366  OutDataTypeStr=T_M_Nm_Float32  PortDimensions=20
  IMAPva_g_ORI_Obj_3DAngleStdDev : Outport  Port=367  OutDataTypeStr=T_M_Nm_Float32  PortDimensions=20
  IMAPva_g_ORI_Obj_AngleRate : Outport  Port=368  OutDataTypeStr=T_M_Nm_Float32  PortDimensions=20
  IMAPva_g_ORI_Obj_AngleRateStdDev : Outport  Port=369  OutDataTypeStr=T_M_Nm_Float32  PortDimensions=20
  IMAPva_g_ORI_Obj_PhiBottom : Outport  Port=370  OutDataTypeStr=T_M_Nm_Float32  PortDimensions=20
  IMAPva_g_ORI_Obj_PhiBottomStdDev : Outport  Port=371  OutDataTypeStr=T_M_Nm_Float32  PortDimensions=20
  IMAPva_d_ORI_Obj_Measured : Outport  Port=372  OutDataTypeStr=UInt16  PortDimensions=20
  IMAPva_g_ORI_Obj_Heading : Outport  Port=373  OutDataTypeStr=T_M_Nm_Float32  PortDimensions=20
  IMAPva_g_ORI_Obj_HeadingStdDev : Outport  Port=374  OutDataTypeStr=T_M_Nm_Float32  PortDimensions=20
  IMAPva_d_ORI_Obj_HeadOrientation : Outport  Port=375  OutDataTypeStr=UInt16  PortDimensions=20
  IMAPva_g_ORI_Obj_TTIPC : Outport  Port=376  OutDataTypeStr=T_M_Nm_Float32  PortDimensions=20
  IMAPva_d_ORI_Obj_DirectionIndicator : Outport  Port=377  OutDataTypeStr=UInt16  PortDimensions=20
  IMAPva_d_ORI_Obj_BrakeLight : Outport  Port=378  OutDataTypeStr=UInt16  PortDimensions=20
  IMAPve_d_ORI_L0_ID : Outport  Port=379  OutDataTypeStr=UInt16
  IMAPve_g_ORI_L0_ExistProb : Outport  Port=380  OutDataTypeStr=T_M_Nm_Float32
  IMAPve_g_ORI_L0_DxStart : Outport  Port=381  OutDataTypeStr=T_M_Nm_Float32
  IMAPve_d_ORI_L0_ColorClass : Outport  Port=382  OutDataTypeStr=UInt16
  IMAPve_d_ORI_L0_MeasureType : Outport  Port=383  OutDataTypeStr=UInt16
  IMAPve_g_ORI_L0_TypeConf : Outport  Port=384  OutDataTypeStr=T_M_Nm_Float32
  IMAPve_d_ORI_R0_ID : Outport  Port=385  OutDataTypeStr=UInt16
  IMAPve_g_ORI_R0_ExistProb : Outport  Port=386  OutDataTypeStr=T_M_Nm_Float32
  IMAPve_g_ORI_R0_Dxstart : Outport  Port=387  OutDataTypeStr=T_M_Nm_Float32
  IMAPve_d_ORI_R0_ColorClass : Outport  Port=388  OutDataTypeStr=UInt16
  IMAPve_d_ORI_R0_MeasureType : Outport  Port=389  OutDataTypeStr=UInt16
  IMAPve_g_ORI_R0_TypeConf : Outport  Port=390  OutDataTypeStr=T_M_Nm_Float32
  IMAPve_d_ORI_L1_ID : Outport  Port=391  OutDataTypeStr=UInt16
  IMAPve_g_ORI_L1_ExistProb : Outport  Port=392  OutDataTypeStr=T_M_Nm_Float32
  IMAPve_g_ORI_L1_Dxstart : Outport  Port=393  OutDataTypeStr=T_M_Nm_Float32
  IMAPve_d_ORI_L1_ColorClass : Outport  Port=394  OutDataTypeStr=UInt16
  IMAPve_d_ORI_L1_MeasureType : Outport  Port=395  OutDataTypeStr=UInt16
  IMAPve_g_ORI_L1_TypeConf : Outport  Port=396  OutDataTypeStr=T_M_Nm_Float32
  IMAPve_d_ORI_R1_ID : Outport  Port=397  OutDataTypeStr=UInt16
  IMAPve_g_ORI_R1_ExistProb : Outport  Port=398  OutDataTypeStr=T_M_Nm_Float32
  IMAPve_g_ORI_R1_Dxstart : Outport  Port=399  OutDataTypeStr=T_M_Nm_Float32
  IMAPve_d_ORI_R1_ColorClass : Outport  Port=400  OutDataTypeStr=UInt16
  IMAPve_d_ORI_R1_MeasureType : Outport  Port=401  OutDataTypeStr=UInt16
  IMAPve_g_ORI_R1_TypeConf : Outport  Port=402  OutDataTypeStr=T_M_Nm_Float32
  IMAPve_d_ORI_RoadedgeL0_ID : Outport  Port=403  OutDataTypeStr=UInt16
  IMAPve_g_ORI_RoadedgeL0_ExistProb : Outport  Port=404  OutDataTypeStr=T_M_Nm_Float32
  IMAPve_g_ORI_RoadedgeL0_DxStart : Outport  Port=405  OutDataTypeStr=T_M_Nm_Float32
  IMAPve_g_ORI_RoadedgeL0_DxEnd : Outport  Port=406  OutDataTypeStr=T_M_Nm_Float32
  IMAPve_g_ORI_RoadedgeL0_C1 : Outport  Port=407  OutDataTypeStr=T_M_Nm_Float32
  IMAPve_g_ORI_RoadedgeL0_C0 : Outport  Port=408  OutDataTypeStr=T_M_Nm_Float32
  IMAPve_g_ORI_RoadedgeL0_C3 : Outport  Port=409  OutDataTypeStr=T_M_Nm_Float32
  IMAPve_g_ORI_RoadedgeL0_C2 : Outport  Port=410  OutDataTypeStr=T_M_Nm_Float32
  IMAPve_d_ORI_RoadedgeL0_MeasureType : Outport  Port=411  OutDataTypeStr=UInt16
  IMAPve_d_ORI_RoadedgeL0_Type : Outport  Port=412  OutDataTypeStr=UInt16
  IMAPve_d_ORI_RoadedgeR0_ID : Outport  Port=413  OutDataTypeStr=UInt16
  IMAPve_g_ORI_RoadedgeR0_ExistProb : Outport  Port=414  OutDataTypeStr=T_M_Nm_Float32
  IMAPve_g_ORI_RoadedgeR0_DxStart : Outport  Port=415  OutDataTypeStr=T_M_Nm_Float32
  IMAPve_g_ORI_RoadedgeR0_DxEnd : Outport  Port=416  OutDataTypeStr=T_M_Nm_Float32
  IMAPve_g_ORI_RoadedgeR0_C1 : Outport  Port=417  OutDataTypeStr=T_M_Nm_Float32
  IMAPve_g_ORI_RoadedgeR0_C0 : Outport  Port=418  OutDataTypeStr=T_M_Nm_Float32
  IMAPve_g_ORI_RoadedgeR0_C3 : Outport  Port=419  OutDataTypeStr=T_M_Nm_Float32
  IMAPve_g_ORI_RoadedgeR0_C2 : Outport  Port=420  OutDataTypeStr=T_M_Nm_Float32
  IMAPve_d_ORI_RoadedgeR0_MeasureType : Outport  Port=421  OutDataTypeStr=UInt16
  IMAPve_d_ORI_RoadedgeR0_Type : Outport  Port=422  OutDataTypeStr=UInt16
  IMAPve_d_APA_AutoPark_WorkSt : Outport  Port=423  OutDataTypeStr=UInt16
  IMAPve_g_ob020H_100 : Outport  Port=424  OutDataTypeStr=UInt32
  IMAPve_g_ob020L_100 : Outport  Port=425  OutDataTypeStr=UInt32
  wires:
  SDFAva_g_ORI_Obj_RelVely/1 -> Runnable_IMAP_10ms_sys/302(SDFAva_g_ORI_Obj_RelVely)
  SWINve_y_EMS_ACCResponseStatus/1 -> Runnable_IMAP_10ms_sys/32(SWINve_y_GW_EMS_EMS_Status_ACC)
  Runnable_IMAP_10ms_sys/397(IMAPve_d_ORI_R1_ID) -> IMAPve_d_ORI_R1_ID/1
  SDFAve_y_Lrg_LINE_TYPE/1 -> Runnable_IMAP_10ms_sys/178(SDFAve_y_Lrg_LINE_TYPE)
  Runnable_IMAP_10ms_sys/141(IMAPve_d_TBOX_LocalTimeM) -> IMAPve_d_TBOX_LocalTimeM/1
  Runnable_IMAP_10ms_sys/309(IMAPve_d_BCM_LeftTurn_Switch) -> IMAPve_d_BCM_LeftTurn_Switch/1
  Runnable_IMAP_10ms_sys/303(IMAPve_d_EPS_ESA_State) -> IMAPve_d_EPS_ESA_State/1
  SDFAva_g_ORI_Obj_LateralDis/1 -> Runnable_IMAP_10ms_sys/304(SDFAva_g_ORI_Obj_LateralDis)
  Runnable_IMAP_10ms_sys/352(IMAPva_g_ORI_Obj_LongDisStdDev) -> IMAPva_g_ORI_Obj_LongDisStdDev/1
  SWINve_g_ESC_BrakeWheelCylinderPressure/1 -> Runnable_IMAP_10ms_sys/293(SWINve_g_ESC_BrakeWheelCylinderPressure)
  Runnable_IMAP_10ms_sys/425(IMAPve_g_ob020L_100) -> IMAPve_g_ob020L_100/1
  SDFAva_d_ORI_Obj_ID/1 -> Runnable_IMAP_10ms_sys/298(SDFAva_d_ORI_Obj_ID)
  Runnable_IMAP_10ms_sys/16(IMAPve_d_FCTA_Switch) -> IMAPve_d_FCTA_Switch/1
  Runnable_IMAP_10ms_sys/129(IMAPve_d_EPB_Warn_Req) -> IMAPve_d_EPB_Warn_Req/1
  SDFAva_g_obj_acc_x/1 -> Runnable_IMAP_10ms_sys/104(SDFAva_g_obj_acc_x)
  SDFAve_g_ORI_R0_C0/1 -> Runnable_IMAP_10ms_sys/320(SDFAve_g_ORI_R0_C0)
  SDFAve_d_ORI_Obj_Num/1 -> Runnable_IMAP_10ms_sys/296(SDFAve_d_ORI_Obj_Num)
  SWINve_y_ESC_EPBErrorStatus/1 -> Runnable_IMAP_10ms_sys/201(SWINve_y_ESC_EPBErrorStatus)
  Runnable_IMAP_10ms_sys/273(IMAPve_g_Lrg_VR_End_BACK) -> IMAPve_g_Lrg_VR_End_BACK/1
  SDFAve_g_ORI_R0_C1/1 -> Runnable_IMAP_10ms_sys/319(SDFAve_g_ORI_R0_C1)
  SDFAva_d_obj_status/1 -> Runnable_IMAP_10ms_sys/113(SDFAva_d_obj_status)
  SDFAve_g_ORI_L1_C1/1 -> Runnable_IMAP_10ms_sys/313(SDFAve_g_ORI_L1_C1)
  System_Clock/1 -> Runnable_IMAP_10ms_sys/90(System_Clock)
  Runnable_IMAP_10ms_sys/406(IMAPve_g_ORI_RoadedgeL0_DxEnd) -> IMAPve_g_ORI_RoadedgeL0_DxEnd/1
  Runnable_IMAP_10ms_sys/228(IMAPve_g_R0_VR) -> IMAPve_g_R0_VR/1
  Runnable_IMAP_10ms_sys/52(IMAPve_d_SCC_Left_SwitchSig) -> IMAPve_d_SCC_Left_SwitchSig/1
  SDFAve_g_ORI_L0_C1/1 -> Runnable_IMAP_10ms_sys/307(SDFAve_g_ORI_L0_C1)
  Runnable_IMAP_10ms_sys/84(IMAPve_d_ESC_TCS_Active) -> IMAPve_d_ESC_TCS_Active/1
  Runnable_IMAP_10ms_sys/88(IMAPve_d_ESC_ABS_AlarmSig) -> IMAPve_d_ESC_ABS_AlarmSig/1
  Runnable_IMAP_10ms_sys/419(IMAPve_g_ORI_RoadedgeR0_C3) -> IMAPve_g_ORI_RoadedgeR0_C3/1
  SDFAva_d_ORI_Obj_Class/1 -> Runnable_IMAP_10ms_sys/297(SDFAva_d_ORI_Obj_Class)
  SDFAve_g_R0_C1_COEF/1 -> Runnable_IMAP_10ms_sys/128(SDFAve_g_R0_C1_COEF)
  Runnable_IMAP_10ms_sys/376(IMAPva_g_ORI_Obj_TTIPC) -> IMAPva_g_ORI_Obj_TTIPC/1
  Runnable_IMAP_10ms_sys/404(IMAPve_g_ORI_RoadedgeL0_ExistProb) -> IMAPve_g_ORI_RoadedgeL0_ExistProb/1
  SDFAve_g_ORI_L1_C3/1 -> Runnable_IMAP_10ms_sys/311(SDFAve_g_ORI_L1_C3)
  SDFAve_d_ORI_L1_Type/1 -> Runnable_IMAP_10ms_sys/315(SDFAve_d_ORI_L1_Type)
  Runnable_IMAP_10ms_sys/86(IMAPve_d_ESC_ABS_Active) -> IMAPve_d_ESC_ABS_Active/1
  Runnable_IMAP_10ms_sys/41(IMAPve_g_SW_Angle_Speed) -> IMAPve_g_SW_Angle_Speed/1
  SDFAve_g_ORI_R0_C3/1 -> Runnable_IMAP_10ms_sys/317(SDFAve_g_ORI_R0_C3)
  SDFAve_g_ORI_R0_C2/1 -> Runnable_IMAP_10ms_sys/318(SDFAve_g_ORI_R0_C2)
  SWINve_y_BCM_RFDoorSwitchSt/1 -> Runnable_IMAP_10ms_sys/290(SWINve_y_BCM_RFDoorSwitchSt)
  SWINve_g_EPS_ElectPowerConsumption/1 -> Runnable_IMAP_10ms_sys/262(SWINve_g_EPS_ElectPowerConsumption)
  Runnable_IMAP_10ms_sys/357(IMAPva_d_ORI_Obj_RelVelyStdDevValid) -> IMAPva_d_ORI_Obj_RelVelyStdDevValid/1
  Runnable_IMAP_10ms_sys/270(IMAPve_g_Lrg_C2_BACK) -> IMAPve_g_Lrg_C2_BACK/1
  SDFAve_g_ORI_R0_VR/1 -> Runnable_IMAP_10ms_sys/322(SDFAve_g_ORI_R0_VR)
  Runnable_IMAP_10ms_sys/377(IMAPva_d_ORI_Obj_DirectionIndicator) -> IMAPva_d_ORI_Obj_DirectionIndicator/1
  SDFAva_g_ORI_Obj_RelVel/1 -> Runnable_IMAP_10ms_sys/301(SDFAva_g_ORI_Obj_RelVel)
  Runnable_IMAP_10ms_sys/386(IMAPve_g_ORI_R0_ExistProb) -> IMAPve_g_ORI_R0_ExistProb/1
  Runnable_IMAP_10ms_sys/154(IMAPva_g_ORI_Obj_RelVel) -> IMAPva_g_ORI_Obj_RelVel/1
  SWINve_y_SAS_CalibratedStatus/1 -> Runnable_IMAP_10ms_sys/73(SWINve_y_SWS_calibration)
  Runnable_IMAP_10ms_sys/202(IMAPva_g_obj_acc_y) -> IMAPva_g_obj_acc_y/1
  Runnable_IMAP_10ms_sys/203(IMAPva_g_obj_pos_var_x) -> IMAPva_g_obj_pos_var_x/1
  Runnable_IMAP_10ms_sys/317(IMAPve_d_MP5_FLK_Activation) -> IMAPve_d_MP5_FLK_Activation/1
  SDFAve_g_ORI_L0_VR/1 -> Runnable_IMAP_10ms_sys/310(SDFAve_g_ORI_L0_VR)
  SDFAve_d_ORI_R1_LT/1 -> Runnable_IMAP_10ms_sys/327(SDFAve_d_ORI_R1_LT)
  Runnable_IMAP_10ms_sys/362(IMAPva_g_ORI_Obj_WidthStdDev) -> IMAPva_g_ORI_Obj_WidthStdDev/1
  SDFAva_g_ORI_Obj_LongDis/1 -> Runnable_IMAP_10ms_sys/303(SDFAva_g_ORI_Obj_LongDis)
  Runnable_IMAP_10ms_sys/382(IMAPve_d_ORI_L0_ColorClass) -> IMAPve_d_ORI_L0_ColorClass/1
  Runnable_IMAP_10ms_sys/333(IMAPve_d_ORI_FS_Rain) -> IMAPve_d_ORI_FS_Rain/1
  SDFAve_d_ORI_CIPV_ID/1 -> Runnable_IMAP_10ms_sys/295(SDFAve_d_ORI_CIPV_ID)
  Runnable_IMAP_10ms_sys/85(IMAPve_d_ESC_VehSpd_Valid) -> IMAPve_d_ESC_VehSpd_Valid/1
  Runnable_IMAP_10ms_sys/56(IMAPve_d_BCM_Door_Lock_State) -> IMAPve_d_BCM_Door_Lock_State/1
  Runnable_IMAP_10ms_sys/307(IMAPve_d_EMS_PowertrainCtl_State) -> IMAPve_d_EMS_PowertrainCtl_State/1
  Runnable_IMAP_10ms_sys/398(IMAPve_g_ORI_R1_ExistProb) -> IMAPve_g_ORI_R1_ExistProb/1
  Runnable_IMAP_10ms_sys/48(IMAPve_d_BCM_LF_Door_State) -> IMAPve_d_BCM_LF_Door_State/1
  Runnable_IMAP_10ms_sys/78(IMAPve_d_ACU_Driver_Belt) -> IMAPve_d_ACU_Driver_Belt/1
  SDFAve_d_ORI_L0_Type/1 -> Runnable_IMAP_10ms_sys/309(SDFAve_d_ORI_L0_Type)
  SDFAve_g_ORI_L0_C0/1 -> Runnable_IMAP_10ms_sys/308(SDFAve_g_ORI_L0_C0)
  SWINve_y_BCM_LFDoorSwitchSt/1 -> Runnable_IMAP_10ms_sys/289(SWINve_y_BCM_LFDoorSwitchSt)
  Runnable_IMAP_10ms_sys/215(IMAPve_d_Road_Type) -> IMAPve_d_Road_Type/1
  Runnable_IMAP_10ms_sys/300(IMAPve_g_EPS_SteeringAngle) -> IMAPve_g_EPS_SteeringAngle/1
  SDFAve_d_sen_sta_LF_radar/1 -> Runnable_IMAP_10ms_sys/92(SDFAve_d_sen_sta_LF_radar)
  Runnable_IMAP_10ms_sys/363(IMAPva_g_ORI_Obj_HeightStdDev) -> IMAPva_g_ORI_Obj_HeightStdDev/1
  SDFAve_g_ORI_L0_C3/1 -> Runnable_IMAP_10ms_sys/305(SDFAve_g_ORI_L0_C3)
  Runnable_IMAP_10ms_sys/392(IMAPve_g_ORI_L1_ExistProb) -> IMAPve_g_ORI_L1_ExistProb/1
  SDFAve_d_ORI_R0_LT/1 -> Runnable_IMAP_10ms_sys/321(SDFAve_d_ORI_R0_LT)
  Runnable_IMAP_10ms_sys/385(IMAPve_d_ORI_R0_ID) -> IMAPve_d_ORI_R0_ID/1
  Runnable_IMAP_10ms_sys/383(IMAPve_d_ORI_L0_MeasureType) -> IMAPve_d_ORI_L0_MeasureType/1
  SDFAve_g_ORI_L1_VR/1 -> Runnable_IMAP_10ms_sys/316(SDFAve_g_ORI_L1_VR)
  SDFAve_y_OperatingStatus/1 -> Runnable_IMAP_10ms_sys/194(SDFAve_y_OperatingStatus)
  Runnable_IMAP_10ms_sys/395(IMAPve_d_ORI_L1_MeasureType) -> IMAPve_d_ORI_L1_MeasureType/1
  Runnable_IMAP_10ms_sys/411(IMAPve_d_ORI_RoadedgeL0_MeasureType) -> IMAPve_d_ORI_RoadedgeL0_MeasureType/1
  Runnable_IMAP_10ms_sys/407(IMAPve_g_ORI_RoadedgeL0_C1) -> IMAPve_g_ORI_RoadedgeL0_C1/1
  SWINve_g_EMS_EngActualFlwTorque/1 -> Runnable_IMAP_10ms_sys/16(SWINve_g_EMS_Actual_torque)
  SWINve_g_EMS_DriverTorque/1 -> Runnable_IMAP_10ms_sys/19(SWINve_g_EMS_Driver_wheel_torque)
  SWINve_y_BCM_CHMSLStaus/1 -> Runnable_IMAP_10ms_sys/6(SWINve_y_BCM_CHMSLStatus)
  SWINve_g_ESC_LongitudinalAcceleration/1 -> Runnable_IMAP_10ms_sys/2(SWINve_g_ACCEL_LONGI_CALIB)
  SWINve_y_ESC_BrakingEffort/1 -> Runnable_IMAP_10ms_sys/10(SWINve_y_Braking_effort)
  Runnable_IMAP_10ms_sys/308(IMAPve_d_TCU_TCU_Available) -> IMAPve_d_TCU_TCU_Available/1
  Runnable_IMAP_10ms_sys/348(IMAPva_g_ORI_Obj_AbsAxStdDev) -> IMAPva_g_ORI_Obj_AbsAxStdDev/1
  SWINve_y_EMS_WhetherACCRequestRealized/1 -> Runnable_IMAP_10ms_sys/13(SWINve_y_EMS_ACC_Effecitive_EMS)
  SWINve_y_ESC_ACCAvailable/1 -> Runnable_IMAP_10ms_sys/278(SWINve_y_ESC_ACCAvailable)
  SWINve_y_ESC_EPBSwitchStatics/1 -> Runnable_IMAP_10ms_sys/282(SWINve_y_ESC_EPBSwitchStatics)
  SWINve_y_ESC_EPBSwitchStaticsValidity/1 -> Runnable_IMAP_10ms_sys/283(SWINve_y_ESC_EPBSwitchStaticsValidity)
  SWINve_g_EMS_EngActualIndTorque/1 -> Runnable_IMAP_10ms_sys/263(SWINve_g_EMS_EngActualIndTorque)
  SWINve_y_ESC_FLWHeelSpdFaultSignal/1 -> Runnable_IMAP_10ms_sys/272(SWINve_y_ESC_FLWHeelSpdFaultSignal)
  SWINve_y_ESC_ABSValidity/1 -> Runnable_IMAP_10ms_sys/270(SWINve_y_ESC_ABSValidity)
  SWINve_g_AC_AmbTemp/1 -> Runnable_IMAP_10ms_sys/258(SWINve_g_AC_AmbTemp)
  SWINve_y_MP5_WorkSt/1 -> Runnable_IMAP_10ms_sys/216(SWINve_y_MP5_WorkSt)
  SWINve_y_ESC_FRWHeelSpdFaultSignal/1 -> Runnable_IMAP_10ms_sys/273(SWINve_y_ESC_FRWHeelSpdFaultSignal)
  SWINve_y_Mp5_ISAMode/1 -> Runnable_IMAP_10ms_sys/233(SWINve_y_Mp5_ISAMode)
  SWINve_y_MP5_RCTAActivation/1 -> Runnable_IMAP_10ms_sys/242(SWINve_y_MP5_RCTAActivation)
  SWINve_y_Mp5_LDWWarningMode/1 -> Runnable_IMAP_10ms_sys/234(SWINve_y_Mp5_LDWWarningMode)
  SWINve_y_MP5_BSD_LCW_Activation/1 -> Runnable_IMAP_10ms_sys/240(SWINve_y_MP5_BSD_LCW_Activation)
  SWINve_y_MP5_DMS_SideViewMonitor/1 -> Runnable_IMAP_10ms_sys/228(SWINve_y_MP5_DMS_SideViewMonitor)
  SWINve_y_ESC_EPBWarmingIndicationReq/1 -> Runnable_IMAP_10ms_sys/281(SWINve_y_ESC_EPBWarningIndicationReq)
  SWINve_y_MP5_DMS_SystemEnable/1 -> Runnable_IMAP_10ms_sys/223(SWINve_y_MP5_DMS_SystemEnable)
  SWINve_y_MP5_DMS_LongtimeDriveMonitor/1 -> Runnable_IMAP_10ms_sys/227(SWINve_y_MP5_DMS_LongtimeDriveMonitor)
  SDFAve_g_R0_C3_BACK_COEF/1 -> Runnable_IMAP_10ms_sys/159(SDFAve_g_R0_C3_BACK_COEF)
  SWINve_y_MP5_FLKAActivation/1 -> Runnable_IMAP_10ms_sys/220(SWINve_y_MP5_FLKActivation)
  SWINve_y_MP5_APAModeSelect/1 -> Runnable_IMAP_10ms_sys/217(SWINve_y_MP5_APAModeSelect)
  SWINve_y_BCM_IHBC_Function_Enable/1 -> Runnable_IMAP_10ms_sys/215(SWINve_y_BCM_IHBC_Function_Enabled)
  SWINve_y_EPS_ESAState/1 -> Runnable_IMAP_10ms_sys/206(SWINve_y_EPS_ESAState)
  SWINve_y_BCM_RightTurnSwitchSt/1 -> Runnable_IMAP_10ms_sys/213(SWINve_y_BCM_RightTurnSwitchSt)
  SWINve_y_BCM_LeftTurnSwitchSt/1 -> Runnable_IMAP_10ms_sys/212(SWINve_y_BCM_LeftTurnSwitchSt)
  SWINve_y_ESC_FRWDirection/1 -> Runnable_IMAP_10ms_sys/197(SWINve_y_ESC_FRWDirection)
  SWINve_y_ACU_RearMiddleBeltSwitchSig/1 -> Runnable_IMAP_10ms_sys/208(SWINve_y_ACU_RearMiddleBeltSwitchSig)
  SWINve_y_ESC_RRWDirection/1 -> Runnable_IMAP_10ms_sys/200(SWINve_y_ESC_RRWDirection)
  SWINve_y_EPS_DriverOverride/1 -> Runnable_IMAP_10ms_sys/204(SWINve_y_EPS_DriverOverride)
  SWINve_y_ESC_TCSErrorStatus/1 -> Runnable_IMAP_10ms_sys/198(SWINve_y_ESC_TCSErrorStatus)
  SWINve_y_MP5_UPA_switch/1 -> Runnable_IMAP_10ms_sys/219(SWINve_y_MP5_UPASwitch)
  SWINve_y_ESC_FLWDirection/1 -> Runnable_IMAP_10ms_sys/196(SWINve_y_ESC_FLWDirection)
  SDFAve_g_ORI_L0_C2/1 -> Runnable_IMAP_10ms_sys/306(SDFAve_g_ORI_L0_C2)
  SWINve_g_EPS_SteeringAngle/1 -> Runnable_IMAP_10ms_sys/203(SWINve_g_EPS_SteeringAngle)
  SDFAve_y_Rrg_DETECT_QUALITY/1 -> Runnable_IMAP_10ms_sys/185(SDFAve_y_Rrg_DETECT_QUALITY)
  SDFAve_g_Rrg_VIEW_RANGE_start/1 -> Runnable_IMAP_10ms_sys/183(SDFAve_g_Rrg_VIEW_RANGE_start)
  SDFAve_y_ISAPopupMessage/1 -> Runnable_IMAP_10ms_sys/188(SDFAve_y_ISAPopupMessage)
  Runnable_IMAP_10ms_sys/334(IMAPve_d_ORI_FS_Fog) -> IMAPve_d_ORI_FS_Fog/1
  SDFAve_g_Lrg_C3_BACK_COEF/1 -> Runnable_IMAP_10ms_sys/174(SDFAve_g_Lrg_C3_BACK_COEF)
  SDFAve_g_Rrg_C3_BACK_COEF/1 -> Runnable_IMAP_10ms_sys/182(SDFAve_g_Rrg_C3_BACK_COEF)
  SDFAve_g_Lrg_VIEW_RANGE_end/1 -> Runnable_IMAP_10ms_sys/176(SDFAve_g_Lrg_VIEW_RANGE_end)
  SDFAve_g_Lrg_VIEW_RANGE_start/1 -> Runnable_IMAP_10ms_sys/175(SDFAve_g_Lrg_VIEW_RANGE_start)
  SWINve_y_TCU_ATFailure/1 -> Runnable_IMAP_10ms_sys/76(SWINve_y_TCU_ATFailure)
  SDFAve_g_Lrg_C2_BACK_COEF/1 -> Runnable_IMAP_10ms_sys/173(SDFAve_g_Lrg_C2_BACK_COEF)
  SDFAve_g_R0_C2_BACK_COEF/1 -> Runnable_IMAP_10ms_sys/158(SDFAve_g_R0_C2_BACK_COEF)
  SDFAve_g_Lrg_C0_BACK_COEF/1 -> Runnable_IMAP_10ms_sys/171(SDFAve_g_Lrg_C0_BACK_COEF)
  SDFAve_g_R1_C2_BACK_COEF/1 -> Runnable_IMAP_10ms_sys/168(SDFAve_g_R1_C2_BACK_COEF)
  SDFAve_g_R1_C1_BACK_COEF/1 -> Runnable_IMAP_10ms_sys/167(SDFAve_g_R1_C1_BACK_COEF)
  SWINve_y_MP5_DMS_Sensity/1 -> Runnable_IMAP_10ms_sys/225(SWINve_y_MP5_DMS_Sensity)
  SDFAve_g_L1_BACK_RANGE/1 -> Runnable_IMAP_10ms_sys/165(SDFAve_g_L1_BACK_RANGE)
  SWINve_y_BCM_FrontWiperWorkSt/1 -> Runnable_IMAP_10ms_sys/7(SWINve_y_BCM_State_Front_Wiper)
  SWINve_y_ESC_LongitudinalAccelervalidity/1 -> Runnable_IMAP_10ms_sys/269(SWINve_y_ESC_LongitudinalAccelerationValidity)
  Runnable_IMAP_10ms_sys/71(IMAPve_d_ESC_Brake_Effort) -> IMAPve_d_ESC_Brake_Effort/1
  SDFAve_g_R1_MARK_WIDTH/1 -> Runnable_IMAP_10ms_sys/150(SDFAve_g_R1_MARK_WIDTH)
  SDFAve_g_L0_C3_BACK_COEF/1 -> Runnable_IMAP_10ms_sys/154(SDFAve_g_L0_C3_BACK_COEF)
  SDFAve_g_L0_C2_BACK_COEF/1 -> Runnable_IMAP_10ms_sys/153(SDFAve_g_L0_C2_BACK_COEF)
  SDFAve_g_L1_MARK_WIDTH/1 -> Runnable_IMAP_10ms_sys/142(SDFAve_g_L1_MARK_WIDTH)
  Runnable_IMAP_10ms_sys/240(IMAPve_g_R1_C0) -> IMAPve_g_R1_C0/1
  SDFAve_g_L1_C1_COEF/1 -> Runnable_IMAP_10ms_sys/136(SDFAve_g_L1_C1_COEF)
  SDFAve_g_L1_VIEW_RANGE/1 -> Runnable_IMAP_10ms_sys/139(SDFAve_g_L1_VIEW_RANGE)
  SDFAve_g_R1_C3_COEF/1 -> Runnable_IMAP_10ms_sys/146(SDFAve_g_R1_C3_COEF)
  SDFAve_g_R1_C2_COEF/1 -> Runnable_IMAP_10ms_sys/145(SDFAve_g_R1_C2_COEF)
  SDFAve_d_R0_LINE_TYPE/1 -> Runnable_IMAP_10ms_sys/133(SDFAve_d_R0_LINE_TYPE)
  SDFAve_y_R0_DETECT_QUALITY/1 -> Runnable_IMAP_10ms_sys/132(SDFAve_y_R0_DETECT_QUALITY)
  SDFAve_y_L0_DETECT_QUALITY/1 -> Runnable_IMAP_10ms_sys/124(SDFAve_y_L0_DETECT_QUALITY)
  SWINve_g_EMS_AccPedalPositionRaw/1 -> Runnable_IMAP_10ms_sys/15(SWINve_g_EMS_Acceleration_pedal_position)
  SDFAve_g_R0_C2_COEF/1 -> Runnable_IMAP_10ms_sys/129(SDFAve_g_R0_C2_COEF)
  SDFAve_g_L0_VIEW_RANGE/1 -> Runnable_IMAP_10ms_sys/123(SDFAve_g_L0_VIEW_RANGE)
  SDFAve_g_L0_C0_COEF/1 -> Runnable_IMAP_10ms_sys/119(SDFAve_g_L0_C0_COEF)
  SDFAve_g_L0_C0_BACK_COEF/1 -> Runnable_IMAP_10ms_sys/151(SDFAve_g_L0_C0_BACK_COEF)
  SDFAva_y_obj_class/1 -> Runnable_IMAP_10ms_sys/111(SDFAva_y_obj_class)
  SWINve_y_BCM_LowBeamStatus/1 -> Runnable_IMAP_10ms_sys/249(SWINve_y_BCM_LowBeamStatus)
  SDFAva_y_obj_TurnLight/1 -> Runnable_IMAP_10ms_sys/115(SDFAva_y_obj_TurnLight)
  SDFAve_g_Rrg_C2_BACK_COEF/1 -> Runnable_IMAP_10ms_sys/181(SDFAve_g_Rrg_C2_BACK_COEF)
  SDFAva_g_obj_acc_y/1 -> Runnable_IMAP_10ms_sys/105(SDFAva_g_obj_acc_y)
  SDFAva_y_obj_id/1 -> Runnable_IMAP_10ms_sys/99(SDFAva_y_obj_id)
  SWINve_g_ESC_YawRate/1 -> Runnable_IMAP_10ms_sys/88(SWINve_g_Yaw_speed)
  SWINve_y_EMS_ACCcontrolTorqueAvailable/1 -> Runnable_IMAP_10ms_sys/14(SWINve_y_EMS_ACCcontrol_Available)
  SDFAve_d_sensor_status/1 -> Runnable_IMAP_10ms_sys/91(SDFAve_d_sensor_status)
  SDFAve_d_sen_sta_RB_radar/1 -> Runnable_IMAP_10ms_sys/95(SDFAve_d_sen_sta_RB_radar)
  Runnable_IMAP_10ms_sys/123(IMAPve_d_EMS_ACC_Inhibited) -> IMAPve_d_EMS_ACC_Inhibited/1
  SWINve_g_ESC_VeSpd/1 -> Runnable_IMAP_10ms_sys/86(SWINve_g_Vehicle_speed_of_wheelsensor)
  SWINve_y_ESC_VehicleHoldStatus/1 -> Runnable_IMAP_10ms_sys/85(SWINve_y_Vehicle_Hold_Status)
  SWINve_y_TCU_ActialGear/1 -> Runnable_IMAP_10ms_sys/78(SWINve_y_TCU_Gear_lever_position)
  SWINve_y_GW_TCU_DCTClutchStatus/1 -> Runnable_IMAP_10ms_sys/77(SWINve_y_TCU_DCTClutchStatus)
  SWINve_y_EPS_SteeringHoldState/1 -> Runnable_IMAP_10ms_sys/67(SWINve_y_State_indicating_steer_or_not)
  SWINve_g_EPS_SteeringTorqueValue/1 -> Runnable_IMAP_10ms_sys/72(SWINve_g_Steering_wheel_torque)
  SWINve_y_ESC_Static_slope/1 -> Runnable_IMAP_10ms_sys/69(SWINve_g_Static_slope)
  SWINve_g_SAS_SteeringAngle/1 -> Runnable_IMAP_10ms_sys/70(SWINve_g_Steering_wheel_angle)
  SWINve_y_ESC_EPBStaus/1 -> Runnable_IMAP_10ms_sys/59(SWINve_y_Park_brake_function_status)
  SWINve_d_ESC_FRWHeelPulseCounter/1 -> Runnable_IMAP_10ms_sys/61(SWINve_g_Pulse_counter_front_right_wheel)
  SWINve_d_ESC_RLWHeelPulseCounter/1 -> Runnable_IMAP_10ms_sys/62(SWINve_g_Pulse_counter_rearleft_wheel)
  SDFAve_y_ROAD_TYPE/1 -> Runnable_IMAP_10ms_sys/118(SDFAve_y_ROAD_TYPE)
  SWINve_g_ESC_LateralAccelaration/1 -> Runnable_IMAP_10ms_sys/48(SWINve_g_Lateral_acceleration)
  SWINve_g_ESC_RearLeftWheelSpd/1 -> Runnable_IMAP_10ms_sys/56(SWINve_g_No_filtered_rear_left_speed)
  SWINve_g_ESC_FrontLeftWHeelSpd/1 -> Runnable_IMAP_10ms_sys/54(SWINve_g_No_filtered_front_left_speed)
  SDFAve_g_L1_C0_COEF/1 -> Runnable_IMAP_10ms_sys/135(SDFAve_g_L1_C0_COEF)
  SWINve_y_ACU_DriverBeltSwitchSig/1 -> Runnable_IMAP_10ms_sys/46(SWINve_y_IC_seat_bealt_driver_state)
  SDFAve_y_Rrg_LINE_TYPE/1 -> Runnable_IMAP_10ms_sys/186(SDFAve_y_Rrg_LINE_TYPE)
  SWINve_y_T_box_RemoteHazardReq/1 -> Runnable_IMAP_10ms_sys/41(SWINve_y_T_box_RemoteHazardReq)
  SDFAva_g_obj_pos_y/1 -> Runnable_IMAP_10ms_sys/101(SDFAva_g_obj_pos_y)
  SWINve_y_SAS_SASFailureSts/1 -> Runnable_IMAP_10ms_sys/47(SWINve_y_Internal_SWS_status)
  SDFAve_d_fusion_time_stamp/1 -> Runnable_IMAP_10ms_sys/97(SDFAve_d_fusion_time_stamp)
  SWINve_y_MP5_FCWSwitch/1 -> Runnable_IMAP_10ms_sys/43(SWINve_y_IC_Fcw_Activation_Config)
  SWINve_y_SCC_RightSteeringWheelSwitchSig/1 -> Runnable_IMAP_10ms_sys/38(SWINve_y_GW_SCC_RightSteeringWheelSwitch)
  SWINve_y_SAS_TrimmingStatus/1 -> Runnable_IMAP_10ms_sys/74(SWINve_y_SWS_trim)
  SWINve_g_EMS_LowerestGearMaxTorque/1 -> Runnable_IMAP_10ms_sys/33(SWINve_g_GW_EMS_Pot_WhlTrq_Max)
  SWINve_g_EMS_NotControlableMinPowertra/1 -> Runnable_IMAP_10ms_sys/26(SWINve_g_EMS_WhlTrq_min_offset)
  Runnable_IMAP_10ms_sys/145(IMAPve_d_TBOX_LocalTimeS) -> IMAPve_d_TBOX_LocalTimeS/1
  SWINve_g_EMS_NotControlableMaxPowertra/1 -> Runnable_IMAP_10ms_sys/24(SWINve_g_EMS_WhlTrq_max_offset)
  Runnable_IMAP_10ms_sys/187(IMAPve_g_ORI_R1_W) -> IMAPve_g_ORI_R1_W/1
  SWINve_g_BCM_BattVolt/1 -> Runnable_IMAP_10ms_sys/250(SWINve_g_BCM_BattVolt)
  Runnable_IMAP_10ms_sys/194(IMAPve_d_Fusion_Time_Stamp) -> IMAPve_d_Fusion_Time_Stamp/1
  SWINve_d_TBOX_LocalTimeYear/1 -> Runnable_IMAP_10ms_sys/251(SWINve_d_TBOX_LocalTimeYear)
  Runnable_IMAP_10ms_sys/185(IMAPve_d_ORI_R1_LT) -> IMAPve_d_ORI_R1_LT/1
  Runnable_IMAP_10ms_sys/175(IMAPve_g_ORI_R0_C2) -> IMAPve_g_ORI_R0_C2/1
  Runnable_IMAP_10ms_sys/168(IMAPve_g_ORI_L1_C2) -> IMAPve_g_ORI_L1_C2/1
  Runnable_IMAP_10ms_sys/260(IMAPve_g_L1_C2_Back) -> IMAPve_g_L1_C2_Back/1
  Runnable_IMAP_10ms_sys/142(IMAPve_d_TBOX_LocalTimeD) -> IMAPve_d_TBOX_LocalTimeD/1
  Runnable_IMAP_10ms_sys/182(IMAPve_g_ORI_R1_C2) -> IMAPve_g_ORI_R1_C2/1
  Runnable_IMAP_10ms_sys/176(IMAPve_g_ORI_R0_C1) -> IMAPve_g_ORI_R0_C1/1
  SDFAve_g_L1_C3_COEF/1 -> Runnable_IMAP_10ms_sys/138(SDFAve_g_L1_C3_COEF)
  Runnable_IMAP_10ms_sys/163(IMAPve_g_ORI_L0_C0) -> IMAPve_g_ORI_L0_C0/1
  Runnable_IMAP_10ms_sys/160(IMAPve_g_ORI_L0_C3) -> IMAPve_g_ORI_L0_C3/1
  Runnable_IMAP_10ms_sys/161(IMAPve_g_ORI_L0_C2) -> IMAPve_g_ORI_L0_C2/1
  Runnable_IMAP_10ms_sys/276(IMAPve_g_Rrg_C0_BACK) -> IMAPve_g_Rrg_C0_BACK/1
  Runnable_IMAP_10ms_sys/164(IMAPve_d_ORI_L0_Type) -> IMAPve_d_ORI_L0_Type/1
  Runnable_IMAP_10ms_sys/54(IMAPve_d_BCM_HazardLamp_Switch) -> IMAPve_d_BCM_HazardLamp_Switch/1
  Runnable_IMAP_10ms_sys/152(IMAPve_d_ORI_Obj_Num) -> IMAPve_d_ORI_Obj_Num/1
  SWINve_y_ESC_BrakeReleasedFailsafe/1 -> Runnable_IMAP_10ms_sys/51(SWINve_y_Message_from_ESC_informing)
  SWINve_y_ESC_RLWHeelPulseCounterValidity/1 -> Runnable_IMAP_10ms_sys/64(SWINve_y_Rear_Left_pulse_malfunction)
  Runnable_IMAP_10ms_sys/133(IMAPve_d_ESC_Hold_State) -> IMAPve_d_ESC_Hold_State/1
  Runnable_IMAP_10ms_sys/131(IMAPve_d_EPB_Switch_Valid) -> IMAPve_d_EPB_Switch_Valid/1
  SWINve_y_ESC_FRWHeelPulseCounterValidity/1 -> Runnable_IMAP_10ms_sys/29(SWINve_y_Front_right_pulse_malfunction)
  Runnable_IMAP_10ms_sys/147(IMAPve_d_Radar_State) -> IMAPve_d_Radar_State/1
  Runnable_IMAP_10ms_sys/184(IMAPve_g_ORI_R1_C0) -> IMAPve_g_ORI_R1_C0/1
  Runnable_IMAP_10ms_sys/148(IMAPve_d_Time_System_Clock) -> IMAPve_d_Time_System_Clock/1
  Runnable_IMAP_10ms_sys/149(IMAPve_g_GW_IC_Odometer) -> IMAPve_g_GW_IC_Odometer/1
  Runnable_IMAP_10ms_sys/132(IMAPve_d_ESC_Drive_Direction) -> IMAPve_d_ESC_Drive_Direction/1
  Runnable_IMAP_10ms_sys/128(IMAPve_d_EPB_Display_Req) -> IMAPve_d_EPB_Display_Req/1
  Runnable_IMAP_10ms_sys/130(IMAPve_d_EPB_Switch_State) -> IMAPve_d_EPB_Switch_State/1
  Runnable_IMAP_10ms_sys/188(IMAPve_d_Sensor_Status) -> IMAPve_d_Sensor_Status/1
  Runnable_IMAP_10ms_sys/111(IMAPve_d_EMS_Gearbox_CtlAvail) -> IMAPve_d_EMS_Gearbox_CtlAvail/1
  SWINve_y_ESC_VehDrivingDirection/1 -> Runnable_IMAP_10ms_sys/84(SWINve_y_Vehicle_driving_direction)
  SWINve_g_EMS_MaxPowertrainWheelTorque/1 -> Runnable_IMAP_10ms_sys/23(SWINve_g_EMS_WhlTrq_max)
  Runnable_IMAP_10ms_sys/180(IMAPve_g_ORI_R0_W) -> IMAPve_g_ORI_R0_W/1
  Runnable_IMAP_10ms_sys/126(IMAPve_d_BCM_HighBeam_State) -> IMAPve_d_BCM_HighBeam_State/1
  SWINve_g_EMS_AccPedalPos/1 -> Runnable_IMAP_10ms_sys/18(SWINve_g_EMS_Driver_request)
  SWINve_y_BCM_DoorLockSt/1 -> Runnable_IMAP_10ms_sys/248(SWINve_y_BCM_DoorLockSt)
  SDFAve_g_R0_BACK_RANGE/1 -> Runnable_IMAP_10ms_sys/160(SDFAve_g_R0_BACK_RANGE)
  Runnable_IMAP_10ms_sys/181(IMAPve_g_ORI_R1_C3) -> IMAPve_g_ORI_R1_C3/1
  SDFAva_g_obj_length/1 -> Runnable_IMAP_10ms_sys/110(SDFAva_g_obj_length)
  SDFAve_g_L0_C1_BACK_COEF/1 -> Runnable_IMAP_10ms_sys/152(SDFAve_g_L0_C1_BACK_COEF)
  Runnable_IMAP_10ms_sys/391(IMAPve_d_ORI_L1_ID) -> IMAPve_d_ORI_L1_ID/1
  Runnable_IMAP_10ms_sys/117(IMAPve_d_EMS_ACC_Effective) -> IMAPve_d_EMS_ACC_Effective/1
  Runnable_IMAP_10ms_sys/109(IMAPve_d_TCU_Select_ATMode) -> IMAPve_d_TCU_Select_ATMode/1
  Runnable_IMAP_10ms_sys/23(IMAPve_d_EPS_Trq_State) -> IMAPve_d_EPS_Trq_State/1
  Runnable_IMAP_10ms_sys/104(IMAPve_d_ESC_RR_Wheel_Pulse) -> IMAPve_d_ESC_RR_Wheel_Pulse/1
  SWINve_y_ESC_AEBAvailable/1 -> Runnable_IMAP_10ms_sys/276(SWINve_y_ESC_AEBAvailable)
  SWINve_y_ESC_ABSAlarmSig/1 -> Runnable_IMAP_10ms_sys/271(SWINve_y_ESC_ABSAlarmSig)
  Runnable_IMAP_10ms_sys/100(IMAPve_d_ESC_RR_WhlSpd_Fault) -> IMAPve_d_ESC_RR_WhlSpd_Fault/1
  Runnable_IMAP_10ms_sys/91(IMAPve_d_ESC_RL_WheelPulVal) -> IMAPve_d_ESC_RL_WheelPulVal/1
  Runnable_IMAP_10ms_sys/107(IMAPve_d_TCU_DCT_Clutch_State) -> IMAPve_d_TCU_DCT_Clutch_State/1
  Runnable_IMAP_10ms_sys/191(IMAPve_d_LR_Radar_Status) -> IMAPve_d_LR_Radar_Status/1
  SWINve_y_ESC_DynamicSlopeAccuracy/1 -> Runnable_IMAP_10ms_sys/12(SWINve_y_Dynamic_slope_accuracy)
  SWINve_y_MP5_DMS_DeleteUserNum/1 -> Runnable_IMAP_10ms_sys/224(SWINve_y_MP5_DMS_DeleteUserNum)
  Runnable_IMAP_10ms_sys/157(IMAPva_g_ORI_Obj_RAngle) -> IMAPva_g_ORI_Obj_RAngle/1
  Runnable_IMAP_10ms_sys/98(IMAPve_d_ESC_RL_WhlSpd_Fault) -> IMAPve_d_ESC_RL_WhlSpd_Fault/1
  Runnable_IMAP_10ms_sys/83(IMAPve_d_ESC_MSR_Active) -> IMAPve_d_ESC_MSR_Active/1
  Runnable_IMAP_10ms_sys/90(IMAPve_d_ESC_FR_WheelPulVal) -> IMAPve_d_ESC_FR_WheelPulVal/1
  Runnable_IMAP_10ms_sys/30(IMAPve_g_ESC_YawRate) -> IMAPve_g_ESC_YawRate/1
  SDFAve_g_ORI_R1_C0/1 -> Runnable_IMAP_10ms_sys/326(SDFAve_g_ORI_R1_C0)
  Runnable_IMAP_10ms_sys/347(IMAPva_g_ORI_Obj_LateralDis) -> IMAPva_g_ORI_Obj_LateralDis/1
  Runnable_IMAP_10ms_sys/81(IMAPve_d_ESC_AlarmSig) -> IMAPve_d_ESC_AlarmSig/1
  SDFAva_y_obj_BrakeLight/1 -> Runnable_IMAP_10ms_sys/116(SDFAva_y_obj_BrakeLight)
  Runnable_IMAP_10ms_sys/103(IMAPve_d_ESC_RL_Wheel_Pulse) -> IMAPve_d_ESC_RL_Wheel_Pulse/1
  Runnable_IMAP_10ms_sys/96(IMAPve_d_ESC_FR_WhlSpd_Fault) -> IMAPve_d_ESC_FR_WhlSpd_Fault/1
  Runnable_IMAP_10ms_sys/87(IMAPve_d_ESC_ABS_Valid) -> IMAPve_d_ESC_ABS_Valid/1
  SDFAve_g_R1_BACK_RANGE/1 -> Runnable_IMAP_10ms_sys/170(SDFAve_g_R1_BACK_RANGE)
  Runnable_IMAP_10ms_sys/94(IMAPve_d_ESC_FL_WhlSpd_Fault) -> IMAPve_d_ESC_FL_WhlSpd_Fault/1
  SWINve_y_BCM_LRDoorSwitchSt/1 -> Runnable_IMAP_10ms_sys/292(SWINve_y_BCM_LRDoorSwitchSt)
  Runnable_IMAP_10ms_sys/82(IMAPve_d_ESC_ESC_Active) -> IMAPve_d_ESC_ESC_Active/1
  Runnable_IMAP_10ms_sys/72(IMAPve_g_EMS_Engine_Speed) -> IMAPve_g_EMS_Engine_Speed/1
  SWINve_y_ESC_ACCActive/1 -> Runnable_IMAP_10ms_sys/279(SWINve_y_ESC_ACCActive)
  Runnable_IMAP_10ms_sys/64(IMAPve_g_EMS_MinTWhl_Offset) -> IMAPve_g_EMS_MinTWhl_Offset/1
  Runnable_IMAP_10ms_sys/93(IMAPve_g_ESC_FL_WhlSpd) -> IMAPve_g_ESC_FL_WhlSpd/1
  Runnable_IMAP_10ms_sys/55(IMAPve_d_PEPS_Door_Lock_Req) -> IMAPve_d_PEPS_Door_Lock_Req/1
  Runnable_IMAP_10ms_sys/69(IMAPve_d_EMS_AccPedal_Fault) -> IMAPve_d_EMS_AccPedal_Fault/1
  Runnable_IMAP_10ms_sys/65(IMAPve_g_EMS_Actual_FlwT) -> IMAPve_g_EMS_Actual_FlwT/1
  SWINve_y_SCC_LeftSteeringWheelSwitchSig/1 -> Runnable_IMAP_10ms_sys/37(SWINve_y_GW_SCC_LeftSteeringWheelSwitch)
  Runnable_IMAP_10ms_sys/192(IMAPve_d_RR_Radar_Status) -> IMAPve_d_RR_Radar_Status/1
  Runnable_IMAP_10ms_sys/105(IMAPve_d_TCU_AT_Failure) -> IMAPve_d_TCU_AT_Failure/1
  Runnable_IMAP_10ms_sys/73(IMAPve_d_ESC_Veh_Standstill) -> IMAPve_d_ESC_Veh_Standstill/1
  Runnable_IMAP_10ms_sys/70(IMAPve_g_EMS_Driver_Torque) -> IMAPve_g_EMS_Driver_Torque/1
  Runnable_IMAP_10ms_sys/127(IMAPve_d_EPB_Status) -> IMAPve_d_EPB_Status/1
  Runnable_IMAP_10ms_sys/66(IMAPve_g_EMS_Actual_IndT) -> IMAPve_g_EMS_Actual_IndT/1
  SDFAve_y_R1_DETECT_QUALITY/1 -> Runnable_IMAP_10ms_sys/148(SDFAve_y_R1_DETECT_QUALITY)
  Runnable_IMAP_10ms_sys/36(IMAPve_g_ESC_Brake_Press) -> IMAPve_g_ESC_Brake_Press/1
  Runnable_IMAP_10ms_sys/190(IMAPve_d_RF_Radar_Status) -> IMAPve_d_RF_Radar_Status/1
  Runnable_IMAP_10ms_sys/97(IMAPve_g_ESC_RL_WhlSpd) -> IMAPve_g_ESC_RL_WhlSpd/1
  Runnable_IMAP_10ms_sys/116(IMAPve_d_ESC_ACC_Active) -> IMAPve_d_ESC_ACC_Active/1
  Runnable_IMAP_10ms_sys/61(IMAPve_g_EMS_MaxTWhl) -> IMAPve_g_EMS_MaxTWhl/1
  Runnable_IMAP_10ms_sys/53(IMAPve_d_SCC_Right_SwitchSig) -> IMAPve_d_SCC_Right_SwitchSig/1
  SWINve_y_EPS_TorqueLimitationState/1 -> Runnable_IMAP_10ms_sys/82(SWINve_y_Torque_limitation_if_DAE_limit)
  SDFAve_d_R1_LINE_TYPE/1 -> Runnable_IMAP_10ms_sys/149(SDFAve_d_R1_LINE_TYPE)
  Runnable_IMAP_10ms_sys/63(IMAPve_g_EMS_MinTWhl) -> IMAPve_g_EMS_MinTWhl/1
  SDFAve_y_ISASignType/1 -> Runnable_IMAP_10ms_sys/189(SDFAve_y_ISASignType)
  SWINve_y_TBOX_LocalTimeHour/1 -> Runnable_IMAP_10ms_sys/254(SWINve_y_TBOX_LocalTimeHour)
  SDFAve_g_Rrg_C0_BACK_COEF/1 -> Runnable_IMAP_10ms_sys/179(SDFAve_g_Rrg_C0_BACK_COEF)
  SWINve_y_EMS_PowertrainControlSt/1 -> Runnable_IMAP_10ms_sys/210(SWINve_y_EMS_PowertrainControlSt)
  Runnable_IMAP_10ms_sys/21(IMAPve_d_EPS_LKA_State) -> IMAPve_d_EPS_LKA_State/1
  Runnable_IMAP_10ms_sys/346(IMAPva_g_ORI_Obj_RelVely) -> IMAPva_g_ORI_Obj_RelVely/1
  Runnable_IMAP_10ms_sys/27(IMAPve_g_EPS_LKA_Current) -> IMAPve_g_EPS_LKA_Current/1
  SDFAve_g_L0_MARK_WIDTH/1 -> Runnable_IMAP_10ms_sys/126(SDFAve_g_L0_MARK_WIDTH)
  Runnable_IMAP_10ms_sys/167(IMAPve_g_ORI_L1_C3) -> IMAPve_g_ORI_L1_C3/1
  SWINve_y_ESC_EBDAlarmSig/1 -> Runnable_IMAP_10ms_sys/284(SWINve_y_ESC_EBDAlarmSig)
  SDFAve_g_R0_C0_COEF/1 -> Runnable_IMAP_10ms_sys/127(SDFAve_g_R0_C0_COEF)
  SDFAve_g_L1_C3_BACK_COEF/1 -> Runnable_IMAP_10ms_sys/164(SDFAve_g_L1_C3_BACK_COEF)
  SDFAve_d_L0_LINE_TYPE/1 -> Runnable_IMAP_10ms_sys/125(SDFAve_d_L0_LINE_TYPE)
  Runnable_IMAP_10ms_sys/156(IMAPva_g_ORI_Obj_LAngle) -> IMAPva_g_ORI_Obj_LAngle/1
  Runnable_IMAP_10ms_sys/18(IMAPve_d_DOW_Switch) -> IMAPve_d_DOW_Switch/1
  Runnable_IMAP_10ms_sys/26(IMAPve_d_EPS_TrqLim_State) -> IMAPve_d_EPS_TrqLim_State/1
  Runnable_IMAP_10ms_sys/29(IMAPve_d_ESC_LatAcc_Valid) -> IMAPve_d_ESC_LatAcc_Valid/1
  SWINve_y_Mp5_ELKSwitch/1 -> Runnable_IMAP_10ms_sys/238(SWINve_y_Mp5_ELKSwitch)
  SDFAve_y_TSR_Sign_Type/1 -> Runnable_IMAP_10ms_sys/191(SDFAve_y_TSR_Sign_Type)
  Runnable_IMAP_10ms_sys/10(IMAPve_d_Speed_Limit) -> IMAPve_d_Speed_Limit/1
  SWINve_y_MP5_JA_Alert_Switch/1 -> Runnable_IMAP_10ms_sys/245(SWINve_y_MP5_JA_Alert_Switch)
  Runnable_IMAP_10ms_sys/5(IMAPve_d_FCW_Sensitivity) -> IMAPve_d_FCW_Sensitivity/1
  SWINve_y_BCM_RRDoorSwitchSt/1 -> Runnable_IMAP_10ms_sys/291(SWINve_y_BCM_RRDoorSwitchSt)
  FAPAve_Cnt_AdvancedParkingAssist/1 -> Runnable_IMAP_10ms_sys/294(FAPAve_Cnt_AdvancedParkingAssist)
  Runnable_IMAP_10ms_sys/8(IMAPve_d_ISA_ISLC_Mode) -> IMAPve_d_ISA_ISLC_Mode/1
  SDFAva_d_obj_age/1 -> Runnable_IMAP_10ms_sys/114(SDFAva_d_obj_age)
  SDFAve_d_L1_LINE_TYPE/1 -> Runnable_IMAP_10ms_sys/141(SDFAve_d_L1_LINE_TYPE)
  Runnable_IMAP_10ms_sys/39(IMAPve_g_ESC_DySlope) -> IMAPve_g_ESC_DySlope/1
  Runnable_IMAP_10ms_sys/3(IMAPve_d_AEB_Switch) -> IMAPve_d_AEB_Switch/1
  SWINve_y_BCM_RightlightSt/1 -> Runnable_IMAP_10ms_sys/287(SWINve_y_BCM_RightlightSt)
  Runnable_IMAP_10ms_sys/279(IMAPve_g_Rrg_C3_BACK) -> IMAPve_g_Rrg_C3_BACK/1
  Runnable_IMAP_10ms_sys/114(IMAPve_d_ESC_AEB_Active) -> IMAPve_d_ESC_AEB_Active/1
  Runnable_IMAP_10ms_sys/4(IMAPve_d_FCW_Switch) -> IMAPve_d_FCW_Switch/1
  Runnable_IMAP_10ms_sys/424(IMAPve_g_ob020H_100) -> IMAPve_g_ob020H_100/1
  SWINve_y_MP5_DMS_SmokingMonitor/1 -> Runnable_IMAP_10ms_sys/230(SWINve_y_MP5_DMS_SmokingMonitor)
  Runnable_IMAP_10ms_sys/230(IMAPve_d_R0_Type) -> IMAPve_d_R0_Type/1
  SDFAve_g_R1_C0_COEF/1 -> Runnable_IMAP_10ms_sys/143(SDFAve_g_R1_C0_COEF)
  SDFAve_g_CameraSignalFault/1 -> Runnable_IMAP_10ms_sys/192(SDFAve_g_CameraSignalFault)
  Runnable_IMAP_10ms_sys/418(IMAPve_g_ORI_RoadedgeR0_C0) -> IMAPve_g_ORI_RoadedgeR0_C0/1
  Runnable_IMAP_10ms_sys/405(IMAPve_g_ORI_RoadedgeL0_DxStart) -> IMAPve_g_ORI_RoadedgeL0_DxStart/1
  SDFAve_g_ORI_R1_C2/1 -> Runnable_IMAP_10ms_sys/324(SDFAve_g_ORI_R1_C2)
  Runnable_IMAP_10ms_sys/57(IMAPve_d_EMS_ACC_Status) -> IMAPve_d_EMS_ACC_Status/1
  Runnable_IMAP_10ms_sys/342(IMAPve_d_ORI_FS_OutOfFocus0) -> IMAPve_d_ORI_FS_OutOfFocus0/1
  Runnable_IMAP_10ms_sys/43(IMAPve_d_BCM_Left_Light) -> IMAPve_d_BCM_Left_Light/1
  Runnable_IMAP_10ms_sys/422(IMAPve_d_ORI_RoadedgeR0_Type) -> IMAPve_d_ORI_RoadedgeR0_Type/1
  SDFAve_g_L0_C2_COEF/1 -> Runnable_IMAP_10ms_sys/121(SDFAve_g_L0_C2_COEF)
  Runnable_IMAP_10ms_sys/125(IMAPve_d_BCM_LowBeam_State) -> IMAPve_d_BCM_LowBeam_State/1
  Runnable_IMAP_10ms_sys/423(IMAPve_d_APA_AutoPark_WorkSt) -> IMAPve_d_APA_AutoPark_WorkSt/1
  Runnable_IMAP_10ms_sys/412(IMAPve_d_ORI_RoadedgeL0_Type) -> IMAPve_d_ORI_RoadedgeL0_Type/1
  SWINve_g_ESC_FrontRightWHeelSpd/1 -> Runnable_IMAP_10ms_sys/55(SWINve_g_No_filtered_front_right_speed)
  Runnable_IMAP_10ms_sys/95(IMAPve_g_ESC_FR_WhlSpd) -> IMAPve_g_ESC_FR_WhlSpd/1
  SWINve_y_ESC_VehSpdValidFlag/1 -> Runnable_IMAP_10ms_sys/87(SWINve_y_Vehiclespd_unavailability_flag)
  SWINve_y_EMS_ACCcontrolGearAvailable/1 -> Runnable_IMAP_10ms_sys/22(SWINve_y_EMS_GearBox_ACC_Ctl_Available)
  Runnable_IMAP_10ms_sys/420(IMAPve_g_ORI_RoadedgeR0_C2) -> IMAPve_g_ORI_RoadedgeR0_C2/1
  SWINve_y_ESC_DynamicSlope/1 -> Runnable_IMAP_10ms_sys/11(SWINve_y_Dynamic_slope)
  SWINve_y_EPS_SteerintTorqueSensorSt/1 -> Runnable_IMAP_10ms_sys/259(SWINve_y_EPS_SteeringTorqueSensorSt)
  Runnable_IMAP_10ms_sys/343(IMAPva_g_ORI_Obj_AbsAx) -> IMAPva_g_ORI_Obj_AbsAx/1
  Runnable_IMAP_10ms_sys/413(IMAPve_d_ORI_RoadedgeR0_ID) -> IMAPve_d_ORI_RoadedgeR0_ID/1
  Runnable_IMAP_10ms_sys/62(IMAPve_g_EMS_MaxTWhl_Offset) -> IMAPve_g_EMS_MaxTWhl_Offset/1
  Runnable_IMAP_10ms_sys/195(IMAPve_d_obj_Num) -> IMAPve_d_obj_Num/1
  Runnable_IMAP_10ms_sys/40(IMAPve_g_SW_Angle) -> IMAPve_g_SW_Angle/1
  Runnable_IMAP_10ms_sys/15(IMAPve_d_BSD_LCW_Switch) -> IMAPve_d_BSD_LCW_Switch/1
  SWINve_y_MP5_DMS_UserAccount/1 -> Runnable_IMAP_10ms_sys/232(SWINve_y_MP5_DMS_UserAccount)
  Runnable_IMAP_10ms_sys/14(IMAPve_d_PEPS_RKE_Command) -> IMAPve_d_PEPS_RKE_Command/1
  SWINve_y_PEPS_RKECommand/1 -> Runnable_IMAP_10ms_sys/239(SWINve_y_PEPS_RKECommand)
  SWINve_y_BCM_HighBeamStatus/1 -> Runnable_IMAP_10ms_sys/42(SWINve_y_High_beam_state)
  Runnable_IMAP_10ms_sys/22(IMAPve_g_EPS_SW_Trq) -> IMAPve_g_EPS_SW_Trq/1
  SDFAve_g_L0_C1_COEF/1 -> Runnable_IMAP_10ms_sys/120(SDFAve_g_L0_C1_COEF)
  Runnable_IMAP_10ms_sys/417(IMAPve_g_ORI_RoadedgeR0_C1) -> IMAPve_g_ORI_RoadedgeR0_C1/1
  Runnable_IMAP_10ms_sys/101(IMAPve_d_ESC_FL_Wheel_Pulse) -> IMAPve_d_ESC_FL_Wheel_Pulse/1
  SWINve_y_ESC_EPBDisplayMessageReq/1 -> Runnable_IMAP_10ms_sys/280(SWINve_y_ESC_EPBDisplayMessageReq)
  SWINve_y_Mp5_TSRSwitch/1 -> Runnable_IMAP_10ms_sys/36(SWINve_y_GW_Mp5_TSR_Switch)
  Runnable_IMAP_10ms_sys/208(IMAPva_d_obj_class) -> IMAPva_d_obj_class/1
  Runnable_IMAP_10ms_sys/408(IMAPve_g_ORI_RoadedgeL0_C0) -> IMAPve_g_ORI_RoadedgeL0_C0/1
  SDFAve_d_sen_sta_RF_radar/1 -> Runnable_IMAP_10ms_sys/93(SDFAve_d_sen_sta_RF_radar)
  SDFAve_g_R1_C1_COEF/1 -> Runnable_IMAP_10ms_sys/144(SDFAve_g_R1_C1_COEF)
  Runnable_IMAP_10ms_sys/338(IMAPve_d_ORI_FS_BlurImage0) -> IMAPve_d_ORI_FS_BlurImage0/1
  Runnable_IMAP_10ms_sys/42(IMAPve_d_BCM_HazardLamp) -> IMAPve_d_BCM_HazardLamp/1
  SWINve_y_BCM_FrontWiperSwitchSt/1 -> Runnable_IMAP_10ms_sys/214(SWINve_y_BCM_FrontWiperSwitchSt)
  Runnable_IMAP_10ms_sys/258(IMAPve_g_L1_C0_Back) -> IMAPve_g_L1_C0_Back/1
  Runnable_IMAP_10ms_sys/399(IMAPve_g_ORI_R1_Dxstart) -> IMAPve_g_ORI_R1_Dxstart/1
  Runnable_IMAP_10ms_sys/400(IMAPve_d_ORI_R1_ColorClass) -> IMAPve_d_ORI_R1_ColorClass/1
  SWINve_y_MP5_Language_Set/1 -> Runnable_IMAP_10ms_sys/218(SWINve_y_MP5_LanguageSet)
  Runnable_IMAP_10ms_sys/38(IMAPve_g_ESC_DySlope_Accuracy) -> IMAPve_g_ESC_DySlope_Accuracy/1
  Runnable_IMAP_10ms_sys/158(IMAPva_g_ORI_Obj_Width) -> IMAPva_g_ORI_Obj_Width/1
  Runnable_IMAP_10ms_sys/403(IMAPve_d_ORI_RoadedgeL0_ID) -> IMAPve_d_ORI_RoadedgeL0_ID/1
  Runnable_IMAP_10ms_sys/262(IMAPve_g_L1_Range_Back) -> IMAPve_g_L1_Range_Back/1
  Runnable_IMAP_10ms_sys/354(IMAPva_d_ORI_Obj_RelVelValid) -> IMAPva_d_ORI_Obj_RelVelValid/1
  SWINve_y_Mp5_LSSSwitch/1 -> Runnable_IMAP_10ms_sys/50(SWINve_y_LKA_main_switch)
  SWINve_y_ESC_RRWHeelPulseCounterValidity/1 -> Runnable_IMAP_10ms_sys/65(SWINve_y_Rear_Right_pulse_malfunction)
  SDFAve_g_L1_C2_COEF/1 -> Runnable_IMAP_10ms_sys/137(SDFAve_g_L1_C2_COEF)
  SDFAve_g_R1_C0_BACK_COEF/1 -> Runnable_IMAP_10ms_sys/166(SDFAve_g_R1_C0_BACK_COEF)
  Runnable_IMAP_10ms_sys/75(IMAPve_d_TCU_Target_Gear) -> IMAPve_d_TCU_Target_Gear/1
  Runnable_IMAP_10ms_sys/393(IMAPve_g_ORI_L1_Dxstart) -> IMAPve_g_ORI_L1_Dxstart/1
  Runnable_IMAP_10ms_sys/304(IMAPve_d_ACU_RearLeft_Belt) -> IMAPve_d_ACU_RearLeft_Belt/1
  Runnable_IMAP_10ms_sys/137(IMAPve_d_ESC_EBD_AlarmSig) -> IMAPve_d_ESC_EBD_AlarmSig/1
  Runnable_IMAP_10ms_sys/396(IMAPve_g_ORI_L1_TypeConf) -> IMAPve_g_ORI_L1_TypeConf/1
  SDFAva_g_ORI_Obj_AbsAy/1 -> Runnable_IMAP_10ms_sys/300(SDFAva_g_ORI_Obj_AbsAy)
  SWINve_y_BCM_TrunkSt/1 -> Runnable_IMAP_10ms_sys/288(SWINve_y_BCM_TrunkSt)
  Runnable_IMAP_10ms_sys/268(IMAPve_g_Lrg_C0_BACK) -> IMAPve_g_Lrg_C0_BACK/1
  Runnable_IMAP_10ms_sys/388(IMAPve_d_ORI_R0_ColorClass) -> IMAPve_d_ORI_R0_ColorClass/1
  SWINve_y_PEPS_DoorLockReq/1 -> Runnable_IMAP_10ms_sys/247(SWINve_y_PEPS_DoorLockReq)
  SDFAve_g_R0_VIEW_RANGE/1 -> Runnable_IMAP_10ms_sys/131(SDFAve_g_R0_VIEW_RANGE)
  SWINve_y_MP5_HazardLampCtrlReq/1 -> Runnable_IMAP_10ms_sys/40(SWINve_y_MP5_HazardLampCtrlReq)
  Runnable_IMAP_10ms_sys/390(IMAPve_g_ORI_R0_TypeConf) -> IMAPve_g_ORI_R0_TypeConf/1
  SWINve_y_BCM_HazardSwitchrSt/1 -> Runnable_IMAP_10ms_sys/39(SWINve_y_BCM_HazardSwitchrSt)
  Runnable_IMAP_10ms_sys/77(IMAPve_d_BCM_Ignition_State) -> IMAPve_d_BCM_Ignition_State/1
  Runnable_IMAP_10ms_sys/35(IMAPve_d_ESC_LonAcc_Valid) -> IMAPve_d_ESC_LonAcc_Valid/1
  Runnable_IMAP_10ms_sys/243(IMAPve_g_R1_C3) -> IMAPve_g_R1_C3/1
  Runnable_IMAP_10ms_sys/159(IMAPva_d_ORI_Obj_ID) -> IMAPva_d_ORI_Obj_ID/1
  Runnable_IMAP_10ms_sys/32(IMAPve_g_ESC_UnYawRate) -> IMAPve_g_ESC_UnYawRate/1
  Runnable_IMAP_10ms_sys/115(IMAPve_d_ESC_ACC_Available) -> IMAPve_d_ESC_ACC_Available/1
  Runnable_IMAP_10ms_sys/140(IMAPve_d_TBOX_LocalTimeY) -> IMAPve_d_TBOX_LocalTimeY/1
  Runnable_IMAP_10ms_sys/284(IMAPve_d_Sign_ISA_Value) -> IMAPve_d_Sign_ISA_Value/1
  Runnable_IMAP_10ms_sys/402(IMAPve_g_ORI_R1_TypeConf) -> IMAPve_g_ORI_R1_TypeConf/1
  Runnable_IMAP_10ms_sys/324(IMAPve_d_MP5_DMS_LongtimeDrive) -> IMAPve_d_MP5_DMS_LongtimeDrive/1
  Runnable_IMAP_10ms_sys/335(IMAPve_d_ORI_FS_Splashes0) -> IMAPve_d_ORI_FS_Splashes0/1
  SDFAve_y_ISAValue/1 -> Runnable_IMAP_10ms_sys/187(SDFAve_y_ISAValue)
  SDFAve_g_L1_C2_BACK_COEF/1 -> Runnable_IMAP_10ms_sys/163(SDFAve_g_L1_C2_BACK_COEF)
  Runnable_IMAP_10ms_sys/380(IMAPve_g_ORI_L0_ExistProb) -> IMAPve_g_ORI_L0_ExistProb/1
  Runnable_IMAP_10ms_sys/34(IMAPve_g_ESC_LonAcc) -> IMAPve_g_ESC_LonAcc/1
  Runnable_IMAP_10ms_sys/237(IMAPve_d_L1_Q) -> IMAPve_d_L1_Q/1
  Runnable_IMAP_10ms_sys/329(IMAPve_d_MP5_DMS_UserAccount) -> IMAPve_d_MP5_DMS_UserAccount/1
  Runnable_IMAP_10ms_sys/381(IMAPve_g_ORI_L0_DxStart) -> IMAPve_g_ORI_L0_DxStart/1
  Runnable_IMAP_10ms_sys/235(IMAPve_g_L1_C3) -> IMAPve_g_L1_C3/1
  Runnable_IMAP_10ms_sys/118(IMAPve_d_BCM_FrontWiper_State) -> IMAPve_d_BCM_FrontWiper_State/1
  Runnable_IMAP_10ms_sys/375(IMAPva_d_ORI_Obj_HeadOrientation) -> IMAPva_d_ORI_Obj_HeadOrientation/1
  Runnable_IMAP_10ms_sys/9(IMAPve_d_LDW_Warn_Mode) -> IMAPve_d_LDW_Warn_Mode/1
  SWINve_y_MP5_ESASwitch/1 -> Runnable_IMAP_10ms_sys/237(SWINve_y_MP5_ESASwitch)
  Runnable_IMAP_10ms_sys/281(IMAPve_g_Rrg_VR_End_BACK) -> IMAPve_g_Rrg_VR_End_BACK/1
  Runnable_IMAP_10ms_sys/31(IMAPve_d_ESC_YawRate_Valid) -> IMAPve_d_ESC_YawRate_Valid/1
  Runnable_IMAP_10ms_sys/60(IMAPve_g_EMS_RealPedal) -> IMAPve_g_EMS_RealPedal/1
  Runnable_IMAP_10ms_sys/369(IMAPva_g_ORI_Obj_AngleRateStdDev) -> IMAPva_g_ORI_Obj_AngleRateStdDev/1
  Runnable_IMAP_10ms_sys/371(IMAPva_g_ORI_Obj_PhiBottomStdDev) -> IMAPva_g_ORI_Obj_PhiBottomStdDev/1
  SDFAve_g_Rrg_VIEW_RANGE_end/1 -> Runnable_IMAP_10ms_sys/184(SDFAve_g_Rrg_VIEW_RANGE_end)
  SDFAva_g_obj_pos_var_x/1 -> Runnable_IMAP_10ms_sys/106(SDFAva_g_obj_pos_var_x)
  SDFAve_g_L1_C1_BACK_COEF/1 -> Runnable_IMAP_10ms_sys/162(SDFAve_g_L1_C1_BACK_COEF)
  Runnable_IMAP_10ms_sys/374(IMAPva_g_ORI_Obj_HeadingStdDev) -> IMAPva_g_ORI_Obj_HeadingStdDev/1
  Runnable_IMAP_10ms_sys/259(IMAPve_g_L1_C1_Back) -> IMAPve_g_L1_C1_Back/1
  Runnable_IMAP_10ms_sys/372(IMAPva_d_ORI_Obj_Measured) -> IMAPva_d_ORI_Obj_Measured/1
  Runnable_IMAP_10ms_sys/76(IMAPve_d_TCU_PRND_State) -> IMAPve_d_TCU_PRND_State/1
  Runnable_IMAP_10ms_sys/421(IMAPve_d_ORI_RoadedgeR0_MeasureType) -> IMAPve_d_ORI_RoadedgeR0_MeasureType/1
  Runnable_IMAP_10ms_sys/370(IMAPva_g_ORI_Obj_PhiBottom) -> IMAPva_g_ORI_Obj_PhiBottom/1
  Runnable_IMAP_10ms_sys/170(IMAPve_g_ORI_L1_C0) -> IMAPve_g_ORI_L1_C0/1
  Runnable_IMAP_10ms_sys/286(IMAPve_d_ISA_Sign_Type) -> IMAPve_d_ISA_Sign_Type/1
  SWINve_y_ESC_ESCWorkStatus/1 -> Runnable_IMAP_10ms_sys/27(SWINve_y_ESP_in_regulation)
  Runnable_IMAP_10ms_sys/359(IMAPva_g_ORI_Obj_ClassProb) -> IMAPva_g_ORI_Obj_ClassProb/1
  Runnable_IMAP_10ms_sys/119(IMAPve_d_BCM_CHMSL_Status) -> IMAPve_d_BCM_CHMSL_Status/1
  SDFAve_d_fusion_status/1 -> Runnable_IMAP_10ms_sys/96(SDFAve_d_fusion_status)
  Runnable_IMAP_10ms_sys/415(IMAPve_g_ORI_RoadedgeR0_DxStart) -> IMAPve_g_ORI_RoadedgeR0_DxStart/1
  Runnable_IMAP_10ms_sys/365(IMAPva_g_ORI_Obj_LAngleStdDev) -> IMAPva_g_ORI_Obj_LAngleStdDev/1
  SDFAve_g_Rrg_C1_BACK_COEF/1 -> Runnable_IMAP_10ms_sys/180(SDFAve_g_Rrg_C1_BACK_COEF)
  Runnable_IMAP_10ms_sys/320(IMAPve_d_MP5_DMS_SystemEnable) -> IMAPve_d_MP5_DMS_SystemEnable/1
  Runnable_IMAP_10ms_sys/183(IMAPve_g_ORI_R1_C1) -> IMAPve_g_ORI_R1_C1/1
  Runnable_IMAP_10ms_sys/173(IMAPve_g_ORI_L1_W) -> IMAPve_g_ORI_L1_W/1
  Runnable_IMAP_10ms_sys/414(IMAPve_g_ORI_RoadedgeR0_ExistProb) -> IMAPve_g_ORI_RoadedgeR0_ExistProb/1
  Runnable_IMAP_10ms_sys/113(IMAPve_d_ESC_AEB_Available) -> IMAPve_d_ESC_AEB_Available/1
  Runnable_IMAP_10ms_sys/360(IMAPva_g_ORI_Obj_Height) -> IMAPva_g_ORI_Obj_Height/1
  SDFAve_d_sen_sta_LB_radar/1 -> Runnable_IMAP_10ms_sys/94(SDFAve_d_sen_sta_LB_radar)
  SWINve_y_MP5_FCTAActivation/1 -> Runnable_IMAP_10ms_sys/241(SWINve_y_MP5_FCTAActivation)
  Runnable_IMAP_10ms_sys/361(IMAPva_g_ORI_Obj_LengthStdDev) -> IMAPva_g_ORI_Obj_LengthStdDev/1
  Runnable_IMAP_10ms_sys/368(IMAPva_g_ORI_Obj_AngleRate) -> IMAPva_g_ORI_Obj_AngleRate/1
  Runnable_IMAP_10ms_sys/314(IMAPve_d_MP5_APA_ModeSelect) -> IMAPve_d_MP5_APA_ModeSelect/1
  SWINve_y_TBOX_LocalTimeMounth/1 -> Runnable_IMAP_10ms_sys/252(SWINve_y_TBOX_LocalTimeMonth)
  Runnable_IMAP_10ms_sys/33(IMAPve_g_ESC_VehSpd) -> IMAPve_g_ESC_VehSpd/1
  Runnable_IMAP_10ms_sys/340(IMAPve_d_ORI_FS_FullBlockage0) -> IMAPve_d_ORI_FS_FullBlockage0/1
  Runnable_IMAP_10ms_sys/186(IMAPve_g_ORI_R1_VR) -> IMAPve_g_ORI_R1_VR/1
  Runnable_IMAP_10ms_sys/351(IMAPva_g_ORI_Obj_RelVelyStdDev) -> IMAPva_g_ORI_Obj_RelVelyStdDev/1
  Runnable_IMAP_10ms_sys/344(IMAPva_g_ORI_Obj_AbsAy) -> IMAPva_g_ORI_Obj_AbsAy/1
  Runnable_IMAP_10ms_sys/366(IMAPva_g_ORI_Obj_RAngleStdDev) -> IMAPva_g_ORI_Obj_RAngleStdDev/1
  SWINve_y_EMS_ACCFunctionIhibition/1 -> Runnable_IMAP_10ms_sys/31(SWINve_y_GW_EMS_ACC_Ihibited_By_Engine)
  Runnable_IMAP_10ms_sys/214(IMAPva_d_obj_MotionStatus) -> IMAPva_d_obj_MotionStatus/1
  Runnable_IMAP_10ms_sys/239(IMAPve_g_L1_W) -> IMAPve_g_L1_W/1
  SWINve_y_ESC_ESCAlarmSig/1 -> Runnable_IMAP_10ms_sys/66(SWINve_y_Request_to_light_fault_lamp)
  SWINve_y_EMS_BrakePedalSignal/1 -> Runnable_IMAP_10ms_sys/9(SWINve_y_Brake_secondary_contact)
  SDFAva_g_obj_pos_var_xy/1 -> Runnable_IMAP_10ms_sys/108(SDFAva_g_obj_pos_var_xy)
  Runnable_IMAP_10ms_sys/355(IMAPva_d_ORI_Obj_RelVelyValid) -> IMAPva_d_ORI_Obj_RelVelyValid/1
  SWINve_y_EPS_LKAState/1 -> Runnable_IMAP_10ms_sys/68(SWINve_y_State_of_EPS_for_LKA_function)
  Runnable_IMAP_10ms_sys/353(IMAPva_g_ORI_Obj_LateralDisStdDev) -> IMAPva_g_ORI_Obj_LateralDisStdDev/1
  SWINve_y_TCU_TargetGear/1 -> Runnable_IMAP_10ms_sys/75(SWINve_y_TCU_AGB_Target_position)
  SDFAva_g_obj_vel_y/1 -> Runnable_IMAP_10ms_sys/103(SDFAva_g_obj_vel_y)
  SDFAva_g_obj_vel_x/1 -> Runnable_IMAP_10ms_sys/102(SDFAva_g_obj_vel_x)
  Runnable_IMAP_10ms_sys/1(IMAPve_d_LKA_Main_Switch) -> IMAPve_d_LKA_Main_Switch/1
  Runnable_IMAP_10ms_sys/330(IMAPve_g_ESC_BrkWhlCylinder_Pressure) -> IMAPve_g_ESC_BrkWhlCylinder_Pressure/1
  Runnable_IMAP_10ms_sys/331(IMAPva_d_ORI_Obj_TimeStamp) -> IMAPva_d_ORI_Obj_TimeStamp/1
  Runnable_IMAP_10ms_sys/250(IMAPve_g_L0_C2_Back) -> IMAPve_g_L0_C2_Back/1
  SDFAva_y_obj_MotionStatus/1 -> Runnable_IMAP_10ms_sys/117(SDFAva_y_obj_MotionStatus)
  Runnable_IMAP_10ms_sys/337(IMAPve_d_ORI_FS_LowSun0) -> IMAPve_d_ORI_FS_LowSun0/1
  Runnable_IMAP_10ms_sys/401(IMAPve_d_ORI_R1_MeasureType) -> IMAPve_d_ORI_R1_MeasureType/1
  Runnable_IMAP_10ms_sys/120(IMAPve_d_BCM_BrakeLamp_State) -> IMAPve_d_BCM_BrakeLamp_State/1
  SWINve_g_EMS_HighestGearMinTorque/1 -> Runnable_IMAP_10ms_sys/34(SWINve_g_GW_EMS_Pot_WhlTrq_Min)
  Runnable_IMAP_10ms_sys/189(IMAPve_d_LF_Radar_Status) -> IMAPve_d_LF_Radar_Status/1
  Runnable_IMAP_10ms_sys/44(IMAPve_d_BCM_Right_Light) -> IMAPve_d_BCM_Right_Light/1
  Runnable_IMAP_10ms_sys/165(IMAPve_g_ORI_L0_VR) -> IMAPve_g_ORI_L0_VR/1
  SWINve_y_ACU_RearLeftBeltSwitchSig/1 -> Runnable_IMAP_10ms_sys/207(SWINve_y_ACU_RearLeftBeltSwitchSig)
  SWINve_y_MP5_DMS_UsingPhoneMonitor/1 -> Runnable_IMAP_10ms_sys/229(SWINve_y_MP5_DMS_UsingPhoneMonitor)
  Runnable_IMAP_10ms_sys/92(IMAPve_d_ESC_RR_WheelPulVal) -> IMAPve_d_ESC_RR_WheelPulVal/1
  SDFAva_y_obj_lane/1 -> Runnable_IMAP_10ms_sys/112(SDFAva_y_obj_lane)
  Runnable_IMAP_10ms_sys/263(IMAPve_g_R1_C0_Back) -> IMAPve_g_R1_C0_Back/1
  Runnable_IMAP_10ms_sys/332(IMAPve_d_ORI_FS_OutOfCalib) -> IMAPve_d_ORI_FS_OutOfCalib/1
  Runnable_IMAP_10ms_sys/221(IMAPve_d_L0_Q) -> IMAPve_d_L0_Q/1
  Runnable_IMAP_10ms_sys/11(IMAPve_d_ALC_TLC_Mode) -> IMAPve_d_ALC_TLC_Mode/1
  Runnable_IMAP_10ms_sys/379(IMAPve_d_ORI_L0_ID) -> IMAPve_d_ORI_L0_ID/1
  Runnable_IMAP_10ms_sys/110(IMAPve_d_EMS_Engine_Status) -> IMAPve_d_EMS_Engine_Status/1
  SDFAve_g_ORI_R1_VR/1 -> Runnable_IMAP_10ms_sys/328(SDFAve_g_ORI_R1_VR)
  Runnable_IMAP_10ms_sys/327(IMAPve_d_MP5_DMS_Smoking) -> IMAPve_d_MP5_DMS_Smoking/1
  Runnable_IMAP_10ms_sys/233(IMAPve_g_L1_C1) -> IMAPve_g_L1_C1/1
  Runnable_IMAP_10ms_sys/74(IMAPve_d_TCU_Actual_Gear) -> IMAPve_d_TCU_Actual_Gear/1
  Runnable_IMAP_10ms_sys/384(IMAPve_g_ORI_L0_TypeConf) -> IMAPve_g_ORI_L0_TypeConf/1
  Runnable_IMAP_10ms_sys/358(IMAPva_g_ORI_Obj_ExistProb) -> IMAPva_g_ORI_Obj_ExistProb/1
  Runnable_IMAP_10ms_sys/17(IMAPve_d_RCTA_Swtich) -> IMAPve_d_RCTA_Swtich/1
  SWINve_y_EPS_WarmingLampSt/1 -> Runnable_IMAP_10ms_sys/261(SWINve_y_EPS_WarningLampSt)
  Runnable_IMAP_10ms_sys/289(IMAPve_g_Camera_Signal_Fault) -> IMAPve_g_Camera_Signal_Fault/1
  Runnable_IMAP_10ms_sys/325(IMAPve_d_MP5_DMS_SideView) -> IMAPve_d_MP5_DMS_SideView/1
  SWINve_y_ESC-RLWDirection/1 -> Runnable_IMAP_10ms_sys/199(SWINve_y_ESC-RLWDirection)
  Runnable_IMAP_10ms_sys/326(IMAPve_d_MP5_DMS_UsingPhone) -> IMAPve_d_MP5_DMS_UsingPhone/1
  Runnable_IMAP_10ms_sys/345(IMAPva_g_ORI_Obj_TTIPCStdDev) -> IMAPva_g_ORI_Obj_TTIPCStdDev/1
  Runnable_IMAP_10ms_sys/45(IMAPve_d_ESC_BrakeLamp_Req) -> IMAPve_d_ESC_BrakeLamp_Req/1
  SDFAve_y_Radar_FaultBitSetting_Signal/1 -> Runnable_IMAP_10ms_sys/195(SDFAve_y_Radar_FaultBitSetting_Signal)
  Runnable_IMAP_10ms_sys/410(IMAPve_g_ORI_RoadedgeL0_C2) -> IMAPve_g_ORI_RoadedgeL0_C2/1
  SDFAve_g_R1_C3_BACK_COEF/1 -> Runnable_IMAP_10ms_sys/169(SDFAve_g_R1_C3_BACK_COEF)
  SDFAve_g_L1_C0_BACK_COEF/1 -> Runnable_IMAP_10ms_sys/161(SDFAve_g_L1_C0_BACK_COEF)
  Runnable_IMAP_10ms_sys/409(IMAPve_g_ORI_RoadedgeL0_C3) -> IMAPve_g_ORI_RoadedgeL0_C3/1
  Runnable_IMAP_10ms_sys/20(IMAPve_d_JA_Alert_Switch) -> IMAPve_d_JA_Alert_Switch/1
  Runnable_IMAP_10ms_sys/37(IMAPve_g_ESC_Static_Slope) -> IMAPve_g_ESC_Static_Slope/1
  Runnable_IMAP_10ms_sys/28(IMAPve_g_ESC_LatAcc) -> IMAPve_g_ESC_LatAcc/1
  SDFAve_g_ORI_L1_C0/1 -> Runnable_IMAP_10ms_sys/314(SDFAve_g_ORI_L1_C0)
  Runnable_IMAP_10ms_sys/251(IMAPve_g_L0_C3_Back) -> IMAPve_g_L0_C3_Back/1
  Runnable_IMAP_10ms_sys/216(IMAPve_g_L0_C0) -> IMAPve_g_L0_C0/1
  Runnable_IMAP_10ms_sys/225(IMAPve_g_R0_C1) -> IMAPve_g_R0_C1/1
  Runnable_IMAP_10ms_sys/318(IMAPve_d_MP5_AutoPilot_Switch) -> IMAPve_d_MP5_AutoPilot_Switch/1
  SWINve_y_ESC_LateralAccelarationValidity/1 -> Runnable_IMAP_10ms_sys/267(SWINve_y_ESC_LateralAccelarationValidity)
  Runnable_IMAP_10ms_sys/146(IMAPve_d_TBOX_LocalTime_Valid) -> IMAPve_d_TBOX_LocalTime_Valid/1
  Runnable_IMAP_10ms_sys/322(IMAPve_d_MP5_DMS_Sensity) -> IMAPve_d_MP5_DMS_Sensity/1
  Runnable_IMAP_10ms_sys/316(IMAPve_d_MP5_UPA_Switch) -> IMAPve_d_MP5_UPA_Switch/1
  Runnable_IMAP_10ms_sys/364(IMAPva_g_ORI_Obj_3DAngle) -> IMAPva_g_ORI_Obj_3DAngle/1
  Runnable_IMAP_10ms_sys/321(IMAPve_d_MP5_DMS_DelUserNum) -> IMAPve_d_MP5_DMS_DelUserNum/1
  Runnable_IMAP_10ms_sys/171(IMAPve_d_ORI_L1_Type) -> IMAPve_d_ORI_L1_Type/1
  SWINve_y_TBOX_LocalTimeMinute/1 -> Runnable_IMAP_10ms_sys/255(SWINve_y_TBOX_LocalTimeMinute)
  SWINve_g_ESC_UnfilteredYawRate/1 -> Runnable_IMAP_10ms_sys/89(SWINve_g_YawRate_Raw)
  SDFAve_y_ISAStatus/1 -> Runnable_IMAP_10ms_sys/190(SDFAve_y_ISAStatus)
  SWINve_y_MP5_JA_Modes/1 -> Runnable_IMAP_10ms_sys/244(SWINve_y_MP5_JA_Modes)
  Runnable_IMAP_10ms_sys/139(IMAPve_g_BCM_Battery_Voltage) -> IMAPve_g_BCM_Battery_Voltage/1
  Runnable_IMAP_10ms_sys/319(IMAPve_d_MP5_DMS_MessageType) -> IMAPve_d_MP5_DMS_MessageType/1
  Runnable_IMAP_10ms_sys/112(IMAPve_d_ESC_Brake_Failsafe) -> IMAPve_d_ESC_Brake_Failsafe/1
  SWINve_y_TBOX_LocalTimeSecond/1 -> Runnable_IMAP_10ms_sys/256(SWINve_y_TBOX_LocalTimeSecond)
  Runnable_IMAP_10ms_sys/302(IMAPve_d_EPS_Driver_Active_ESA) -> IMAPve_d_EPS_Driver_Active_ESA/1
  Runnable_IMAP_10ms_sys/336(IMAPve_d_ORI_FS_SunRay0) -> IMAPve_d_ORI_FS_SunRay0/1
  SWINve_y_ESC_VehicleStandstill/1 -> Runnable_IMAP_10ms_sys/83(SWINve_y_Vehicle_detected_as_stationary)
  Runnable_IMAP_10ms_sys/6(IMAPve_d_ISA_Switch) -> IMAPve_d_ISA_Switch/1
  SWINve_y_MP5_MDS_Message_type/1 -> Runnable_IMAP_10ms_sys/222(SWINve_y_MP5_DMS_MessageType)
  Runnable_IMAP_10ms_sys/301(IMAPve_d_EPS_Driver_Override) -> IMAPve_d_EPS_Driver_Override/1
  Runnable_IMAP_10ms_sys/150(IMAPve_d_Outside_Temp) -> IMAPve_d_Outside_Temp/1
  Runnable_IMAP_10ms_sys/207(IMAPva_g_obj_length) -> IMAPva_g_obj_length/1
  Runnable_IMAP_10ms_sys/89(IMAPve_d_ESC_FL_WheelPulVal) -> IMAPve_d_ESC_FL_WheelPulVal/1
  Runnable_IMAP_10ms_sys/211(IMAPva_d_obj_age) -> IMAPva_d_obj_age/1
  Runnable_IMAP_10ms_sys/59(IMAPve_g_EMS_Pot_WhlT_Min) -> IMAPve_g_EMS_Pot_WhlT_Min/1
  Runnable_IMAP_10ms_sys/315(IMAPve_d_MP5_LanguageSet) -> IMAPve_d_MP5_LanguageSet/1
  Runnable_IMAP_10ms_sys/306(IMAPve_d_ACU_RearRight_Belt) -> IMAPve_d_ACU_RearRight_Belt/1
  Runnable_IMAP_10ms_sys/387(IMAPve_g_ORI_R0_Dxstart) -> IMAPve_g_ORI_R0_Dxstart/1
  Runnable_IMAP_10ms_sys/313(IMAPve_d_MP5_Work_State) -> IMAPve_d_MP5_Work_State/1
  SDFAve_y_L1_DETECT_QUALITY/1 -> Runnable_IMAP_10ms_sys/140(SDFAve_y_L1_DETECT_QUALITY)
  Runnable_IMAP_10ms_sys/204(IMAPva_g_obj_pos_var_y) -> IMAPva_g_obj_pos_var_y/1
  Runnable_IMAP_10ms_sys/312(IMAPve_d_BCM_IHBC_Enabled) -> IMAPve_d_BCM_IHBC_Enabled/1
  Runnable_IMAP_10ms_sys/311(IMAPve_d_BCM_FrontWiper_Switch) -> IMAPve_d_BCM_FrontWiper_Switch/1
  Runnable_IMAP_10ms_sys/223(IMAPve_g_L0_W) -> IMAPve_g_L0_W/1
  SDFAve_y_Lrg_DETECT_QUALITY/1 -> Runnable_IMAP_10ms_sys/177(SDFAve_y_Lrg_DETECT_QUALITY)
  SWINve_y_MP5_AutoPilotSwitch/1 -> Runnable_IMAP_10ms_sys/221(SWINve_y_MP5_AutoPilotSwitch)
  Runnable_IMAP_10ms_sys/255(IMAPve_g_R0_C2_Back) -> IMAPve_g_R0_C2_Back/1
  Runnable_IMAP_10ms_sys/201(IMAPva_g_obj_acc_x) -> IMAPva_g_obj_acc_x/1
  Runnable_IMAP_10ms_sys/292(IMAPve_d_Camera_Status) -> IMAPve_d_Camera_Status/1
  SWINve_g_ESC_BrakeOilPress/1 -> Runnable_IMAP_10ms_sys/81(SWINve_g_TMC_pressure)
  SWINve_y_BCM_BrakeLampStaus/1 -> Runnable_IMAP_10ms_sys/5(SWINve_y_BCM_BrakeLampStatus)
  SDFAve_g_ORI_L1_C2/1 -> Runnable_IMAP_10ms_sys/312(SDFAve_g_ORI_L1_C2)
  Runnable_IMAP_10ms_sys/124(IMAPve_d_EMS_Brake_Pedal) -> IMAPve_d_EMS_Brake_Pedal/1
  SWINve_y_BCM_IgnitionSt/1 -> Runnable_IMAP_10ms_sys/30(SWINve_y_GW_BCM_SEV_main_state)
  Runnable_IMAP_10ms_sys/299(IMAPve_d_EPS_SteeringAngle_Flag) -> IMAPve_d_EPS_SteeringAngle_Flag/1
  Runnable_IMAP_10ms_sys/19(IMAPve_d_JA_Brake_Switch) -> IMAPve_d_JA_Brake_Switch/1
  SWINve_y_MP5_DMS_EyeFatigueMonitor/1 -> Runnable_IMAP_10ms_sys/226(SWINve_y_MP5_DMS_EyeFatigueMonitor)
  Runnable_IMAP_10ms_sys/295(IMAPve_d_ESC_TCS_ErrorStatus) -> IMAPve_d_ESC_TCS_ErrorStatus/1
  Runnable_IMAP_10ms_sys/25(IMAPve_d_SAS_Trim_State) -> IMAPve_d_SAS_Trim_State/1
  Runnable_IMAP_10ms_sys/293(IMAPve_d_ESC_FLW_Direction) -> IMAPve_d_ESC_FLW_Direction/1
  Runnable_IMAP_10ms_sys/46(IMAPve_d_BCM_Opening_State) -> IMAPve_d_BCM_Opening_State/1
  Runnable_IMAP_10ms_sys/298(IMAPve_d_ESC_EPB_ErrorStatus) -> IMAPve_d_ESC_EPB_ErrorStatus/1
  Runnable_IMAP_10ms_sys/288(IMAPve_d_TSR_Sign_Type) -> IMAPve_d_TSR_Sign_Type/1
  Runnable_IMAP_10ms_sys/290(IMAPve_d_Camera_State) -> IMAPve_d_Camera_State/1
  SDFAva_g_obj_pos_x/1 -> Runnable_IMAP_10ms_sys/100(SDFAva_g_obj_pos_x)
  Runnable_IMAP_10ms_sys/265(IMAPve_g_R1_C2_Back) -> IMAPve_g_R1_C2_Back/1
  Runnable_IMAP_10ms_sys/310(IMAPve_d_BCM_RightTurn_Switch) -> IMAPve_d_BCM_RightTurn_Switch/1
  SWINve_y_BCM_LeftlightSt/1 -> Runnable_IMAP_10ms_sys/286(SWINve_y_BCM_LeftlightSt)
  SDFAve_g_L0_C3_COEF/1 -> Runnable_IMAP_10ms_sys/122(SDFAve_g_L0_C3_COEF)
  SWINve_y_MP5_DOWActivation/1 -> Runnable_IMAP_10ms_sys/243(SWINve_y_MP5_DOWActivation)
  Runnable_IMAP_10ms_sys/231(IMAPve_g_R0_W) -> IMAPve_g_R0_W/1
  Runnable_IMAP_10ms_sys/282(IMAPve_d_Rrg_Q_BACK) -> IMAPve_d_Rrg_Q_BACK/1
  Runnable_IMAP_10ms_sys/121(IMAPve_d_ACU_Passenger_Belt) -> IMAPve_d_ACU_Passenger_Belt/1
  Runnable_IMAP_10ms_sys/305(IMAPve_d_ACU_RearMiddle_Belt) -> IMAPve_d_ACU_RearMiddle_Belt/1
  Runnable_IMAP_10ms_sys/153(IMAPva_d_ORI_Obj_Class) -> IMAPva_d_ORI_Obj_Class/1
  Runnable_IMAP_10ms_sys/278(IMAPve_g_Rrg_C2_BACK) -> IMAPve_g_Rrg_C2_BACK/1
  Runnable_IMAP_10ms_sys/99(IMAPve_g_ESC_RR_WhlSpd) -> IMAPve_g_ESC_RR_WhlSpd/1
  Runnable_IMAP_10ms_sys/144(IMAPve_d_TBOX_LocalTimeMin) -> IMAPve_d_TBOX_LocalTimeMin/1
  Runnable_IMAP_10ms_sys/166(IMAPve_g_ORI_L0_W) -> IMAPve_g_ORI_L0_W/1
  Runnable_IMAP_10ms_sys/280(IMAPve_g_Rrg_VR_Start_BACK) -> IMAPve_g_Rrg_VR_Start_BACK/1
  SWINve_y_EPS_DriverInitializedESA/1 -> Runnable_IMAP_10ms_sys/205(SWINve_y_EPS_DriverInitializedESA)
  SDFAve_g_ORI_R1_C1/1 -> Runnable_IMAP_10ms_sys/325(SDFAve_g_ORI_R1_C1)
  Runnable_IMAP_10ms_sys/275(IMAPve_d_Lrg_TYPE_BACK) -> IMAPve_d_Lrg_TYPE_BACK/1
  Runnable_IMAP_10ms_sys/122(IMAPve_d_EMS_ACC_CtlAvail) -> IMAPve_d_EMS_ACC_CtlAvail/1
  SWINve_y_ESC_RLWHeelSpdFaultSignal/1 -> Runnable_IMAP_10ms_sys/274(SWINve_y_ESC_RLWHeelSpdFaultSignal)
  Runnable_IMAP_10ms_sys/162(IMAPve_g_ORI_L0_C1) -> IMAPve_g_ORI_L0_C1/1
  Runnable_IMAP_10ms_sys/277(IMAPve_g_Rrg_C1_BACK) -> IMAPve_g_Rrg_C1_BACK/1
  SWINve_g_ESC_RearRightWheelSpd/1 -> Runnable_IMAP_10ms_sys/57(SWINve_g_No_filtered_rear_rignt_speed)
  SWINve_y_ACU_PassengerBeltSwitchSig/1 -> Runnable_IMAP_10ms_sys/45(SWINve_y_IC_passengerBeltSwitchSig)
  Runnable_IMAP_10ms_sys/106(IMAPve_d_TCU_Shift_Valid) -> IMAPve_d_TCU_Shift_Valid/1
  Runnable_IMAP_10ms_sys/229(IMAPve_d_R0_Q) -> IMAPve_d_R0_Q/1
  Runnable_IMAP_10ms_sys/13(IMAPve_d_ELK_Switch) -> IMAPve_d_ELK_Switch/1
  Runnable_IMAP_10ms_sys/47(IMAPve_d_BCM_Trunk_State) -> IMAPve_d_BCM_Trunk_State/1
  SWINve_y_TCU_PRNDLStatus/1 -> Runnable_IMAP_10ms_sys/265(SWINve_y_TCU_PRNDLStatus)
  Runnable_IMAP_10ms_sys/271(IMAPve_g_Lrg_C3_BACK) -> IMAPve_g_Lrg_C3_BACK/1
  Runnable_IMAP_10ms_sys/136(IMAPve_g_EPS_PowerCon) -> IMAPve_g_EPS_PowerCon/1
  Runnable_IMAP_10ms_sys/135(IMAPve_d_EPS_Warning_State) -> IMAPve_d_EPS_Warning_State/1
  Runnable_IMAP_10ms_sys/134(IMAPve_d_EPS_Steer_Hold_State) -> IMAPve_d_EPS_Steer_Hold_State/1
  Runnable_IMAP_10ms_sys/266(IMAPve_g_R1_C3_Back) -> IMAPve_g_R1_C3_Back/1
  Runnable_IMAP_10ms_sys/241(IMAPve_g_R1_C1) -> IMAPve_g_R1_C1/1
  Runnable_IMAP_10ms_sys/291(IMAPve_d_Radar_FaultBitSetting_Signal) -> IMAPve_d_Radar_FaultBitSetting_Signal/1
  Runnable_IMAP_10ms_sys/222(IMAPve_d_L0_Type) -> IMAPve_d_L0_Type/1
  Runnable_IMAP_10ms_sys/261(IMAPve_g_L1_C3_Back) -> IMAPve_g_L1_C3_Back/1
  SWINve_y_ESC_FLWHeelPulseCounterValidity/1 -> Runnable_IMAP_10ms_sys/28(SWINve_y_Front_Left_pulse_malfunction)
  SWINve_y_TCU_TCUAvailable/1 -> Runnable_IMAP_10ms_sys/211(SWINve_y_TCU_TCUAvailable)
  SDFAve_g_R0_C3_COEF/1 -> Runnable_IMAP_10ms_sys/130(SDFAve_g_R0_C3_COEF)
  SDFAve_g_R0_MARK_WIDTH/1 -> Runnable_IMAP_10ms_sys/134(SDFAve_g_R0_MARK_WIDTH)
  Runnable_IMAP_10ms_sys/174(IMAPve_g_ORI_R0_C3) -> IMAPve_g_ORI_R0_C3/1
  Runnable_IMAP_10ms_sys/272(IMAPve_g_Lrg_VR_Start_BACK) -> IMAPve_g_Lrg_VR_Start_BACK/1
  SWINve_y_ESC_ESCOFF/1 -> Runnable_IMAP_10ms_sys/3(SWINve_y_ASR_ESP_disconnected)
  SWINve_d_ESC_FLWHeelPulseCounter/1 -> Runnable_IMAP_10ms_sys/60(SWINve_g_Pulse_counter_front_left_wheel)
  Runnable_IMAP_10ms_sys/257(IMAPve_g_R0_Range_Back) -> IMAPve_g_R0_Range_Back/1
  Runnable_IMAP_10ms_sys/269(IMAPve_g_Lrg_C1_BACK) -> IMAPve_g_Lrg_C1_BACK/1
  SWINve_y_MP5_AEBSwitch/1 -> Runnable_IMAP_10ms_sys/52(SWINve_y_MP5_AEB_Activation_Config)
  Runnable_IMAP_10ms_sys/2(IMAPve_d_LKA_Mode) -> IMAPve_d_LKA_Mode/1
  SDFAva_g_ORI_Obj_AbsAx/1 -> Runnable_IMAP_10ms_sys/299(SDFAva_g_ORI_Obj_AbsAx)
  Runnable_IMAP_10ms_sys/253(IMAPve_g_R0_C0_Back) -> IMAPve_g_R0_C0_Back/1
  Runnable_IMAP_10ms_sys/349(IMAPva_g_ORI_Obj_AbsAyStdDev) -> IMAPva_g_ORI_Obj_AbsAyStdDev/1
  Runnable_IMAP_10ms_sys/296(IMAPve_d_ESC_RLW_Direction) -> IMAPve_d_ESC_RLW_Direction/1
  Runnable_IMAP_10ms_sys/210(IMAPva_d_obj_status) -> IMAPva_d_obj_status/1
  SWINve_y_TCU_GearEngagement/1 -> Runnable_IMAP_10ms_sys/79(SWINve_y_TCU_GearEngagement)
  Runnable_IMAP_10ms_sys/244(IMAPve_g_R1_VR) -> IMAPve_g_R1_VR/1
  SDFAve_d_obj_Num/1 -> Runnable_IMAP_10ms_sys/98(SDFAve_d_obj_Num)
  Runnable_IMAP_10ms_sys/283(IMAPve_d_Rrg_TYPE_BACK) -> IMAPve_d_Rrg_TYPE_BACK/1
  Runnable_IMAP_10ms_sys/178(IMAPve_d_ORI_R0_LT) -> IMAPve_d_ORI_R0_LT/1
  Runnable_IMAP_10ms_sys/248(IMAPve_g_L0_C0_Back) -> IMAPve_g_L0_C0_Back/1
  Runnable_IMAP_10ms_sys/256(IMAPve_g_R0_C3_Back) -> IMAPve_g_R0_C3_Back/1
  Runnable_IMAP_10ms_sys/193(IMAPve_d_Fusion_Status) -> IMAPve_d_Fusion_Status/1
  Runnable_IMAP_10ms_sys/285(IMAPve_d_ISA_Popup_Message) -> IMAPve_d_ISA_Popup_Message/1
  Runnable_IMAP_10ms_sys/367(IMAPva_g_ORI_Obj_3DAngleStdDev) -> IMAPva_g_ORI_Obj_3DAngleStdDev/1
  SWINve_y_ESC_TCSCtlActive/1 -> Runnable_IMAP_10ms_sys/4(SWINve_y_ASR_in_regulation)
  SWINve_y_MP5_DMS_DrinkWaterMonitor/1 -> Runnable_IMAP_10ms_sys/231(SWINve_y_MP5_DMS_DrinkWaterMonitor)
  Runnable_IMAP_10ms_sys/24(IMAPve_d_SAS_Clb_State) -> IMAPve_d_SAS_Clb_State/1
  Runnable_IMAP_10ms_sys/50(IMAPve_d_BCM_RR_Door_State) -> IMAPve_d_BCM_RR_Door_State/1
  Runnable_IMAP_10ms_sys/252(IMAPve_g_L0_Range_Back) -> IMAPve_g_L0_Range_Back/1
  Runnable_IMAP_10ms_sys/68(IMAPve_g_EMS_ACC_VirtualPedal) -> IMAPve_g_EMS_ACC_VirtualPedal/1
  SWINve_y_EMS_AccPedalFaultBit/1 -> Runnable_IMAP_10ms_sys/264(SWINve_y_EMS_AccPedalFaultBit)
  Runnable_IMAP_10ms_sys/143(IMAPve_d_TBOX_LocalTimeH) -> IMAPve_d_TBOX_LocalTimeH/1
  Runnable_IMAP_10ms_sys/49(IMAPve_d_BCM_RF_Door_State) -> IMAPve_d_BCM_RF_Door_State/1
  SWINve_d_ESC_RRWHeelPulseCounter/1 -> Runnable_IMAP_10ms_sys/63(SWINve_g_Pulse_counter_rearright_wheel)
  Runnable_IMAP_10ms_sys/102(IMAPve_d_ESC_FR_Wheel_Pulse) -> IMAPve_d_ESC_FR_Wheel_Pulse/1
  Runnable_IMAP_10ms_sys/246(IMAPve_d_R1_Type) -> IMAPve_d_R1_Type/1
  SWINve_y_EPS_SteeringAngle_Flag/1 -> Runnable_IMAP_10ms_sys/202(SWINve_y_EPS_SteeringAngle_Flag)
  Runnable_IMAP_10ms_sys/236(IMAPve_g_L1_VR) -> IMAPve_g_L1_VR/1
  Runnable_IMAP_10ms_sys/80(IMAPve_d_ESC_OFF) -> IMAPve_d_ESC_OFF/1
  Runnable_IMAP_10ms_sys/287(IMAPve_d_ISA_Status) -> IMAPve_d_ISA_Status/1
  Runnable_IMAP_10ms_sys/242(IMAPve_g_R1_C2) -> IMAPve_g_R1_C2/1
  Runnable_IMAP_10ms_sys/416(IMAPve_g_ORI_RoadedgeR0_DxEnd) -> IMAPve_g_ORI_RoadedgeR0_DxEnd/1
  Runnable_IMAP_10ms_sys/12(IMAPve_d_ESA_Switch) -> IMAPve_d_ESA_Switch/1
  SWINve_y_Mp5_ISASwitch/1 -> Runnable_IMAP_10ms_sys/35(SWINve_y_GW_Mp5_ISA_Switch)
  SDFAve_g_Lrg_C1_BACK_COEF/1 -> Runnable_IMAP_10ms_sys/172(SDFAve_g_Lrg_C1_BACK_COEF)
  Runnable_IMAP_10ms_sys/245(IMAPve_d_R1_Q) -> IMAPve_d_R1_Q/1
  Runnable_IMAP_10ms_sys/224(IMAPve_g_R0_C0) -> IMAPve_g_R0_C0/1
  SWINve_y_TBOX_LocalTimeValid/1 -> Runnable_IMAP_10ms_sys/257(SWINve_y_TBOX_LocalTimeValid)
  Runnable_IMAP_10ms_sys/238(IMAPve_d_L1_Type) -> IMAPve_d_L1_Type/1
  Runnable_IMAP_10ms_sys/226(IMAPve_g_R0_C2) -> IMAPve_g_R0_C2/1
  Runnable_IMAP_10ms_sys/328(IMAPve_d_MP5_DMS_DrinkWater) -> IMAPve_d_MP5_DMS_DrinkWater/1
  Runnable_IMAP_10ms_sys/294(IMAPve_d_ESC_FRW_Direction) -> IMAPve_d_ESC_FRW_Direction/1
  Runnable_IMAP_10ms_sys/220(IMAPve_g_L0_VR) -> IMAPve_g_L0_VR/1
  Runnable_IMAP_10ms_sys/350(IMAPva_g_ORI_Obj_RelVelStdDev) -> IMAPva_g_ORI_Obj_RelVelStdDev/1
  Runnable_IMAP_10ms_sys/58(IMAPve_g_EMS_Pot_WhlT_Max) -> IMAPve_g_EMS_Pot_WhlT_Max/1
  Runnable_IMAP_10ms_sys/232(IMAPve_g_L1_C0) -> IMAPve_g_L1_C0/1
  Runnable_IMAP_10ms_sys/264(IMAPve_g_R1_C1_Back) -> IMAPve_g_R1_C1_Back/1
  Runnable_IMAP_10ms_sys/297(IMAPve_d_ESC_RRW_Direction) -> IMAPve_d_ESC_RRW_Direction/1
  Runnable_IMAP_10ms_sys/67(IMAPve_g_EMS_Realize_TWhl) -> IMAPve_g_EMS_Realize_TWhl/1
  Runnable_IMAP_10ms_sys/177(IMAPve_g_ORI_R0_C0) -> IMAPve_g_ORI_R0_C0/1
  SDFAve_g_R1_VIEW_RANGE/1 -> Runnable_IMAP_10ms_sys/147(SDFAve_g_R1_VIEW_RANGE)
  Runnable_IMAP_10ms_sys/356(IMAPva_d_ORI_Obj_RelVelStdDevValid) -> IMAPva_d_ORI_Obj_RelVelStdDevValid/1
  SDFAve_g_ORI_R1_C3/1 -> Runnable_IMAP_10ms_sys/323(SDFAve_g_ORI_R1_C3)
  SWINve_g_EPS_LKACurrentOverlay/1 -> Runnable_IMAP_10ms_sys/260(SWINve_g_EPS_LKACurrentOverlay)
  SDFAve_g_L0_BACK_RANGE/1 -> Runnable_IMAP_10ms_sys/155(SDFAve_g_L0_BACK_RANGE)
  SDFAve_g_R0_C0_BACK_COEF/1 -> Runnable_IMAP_10ms_sys/156(SDFAve_g_R0_C0_BACK_COEF)
  SDFAve_y_Radar_State/1 -> Runnable_IMAP_10ms_sys/193(SDFAve_y_Radar_State)
  Runnable_IMAP_10ms_sys/341(IMAPve_d_ORI_FS_FrozenWindshield0) -> IMAPve_d_ORI_FS_FrozenWindshield0/1
  Runnable_IMAP_10ms_sys/274(IMAPve_d_Lrg_Q_BACK) -> IMAPve_d_Lrg_Q_BACK/1
  Runnable_IMAP_10ms_sys/179(IMAPve_g_ORI_R0_VR) -> IMAPve_g_ORI_R0_VR/1
  Runnable_IMAP_10ms_sys/169(IMAPve_g_ORI_L1_C1) -> IMAPve_g_ORI_L1_C1/1
  SWINve_y_EMS_EngRunningStatus/1 -> Runnable_IMAP_10ms_sys/21(SWINve_y_EMS_Engine_state)
  Runnable_IMAP_10ms_sys/151(IMAPve_d_ORI_CIPV_ID) -> IMAPve_d_ORI_CIPV_ID/1
  Runnable_IMAP_10ms_sys/209(IMAPva_d_obj_lane) -> IMAPva_d_obj_lane/1
  SWINve_y_ESC_AEBActive/1 -> Runnable_IMAP_10ms_sys/277(SWINve_y_ESC_AEBActive)
  Runnable_IMAP_10ms_sys/227(IMAPve_g_R0_C3) -> IMAPve_g_R0_C3/1
  Runnable_IMAP_10ms_sys/373(IMAPva_g_ORI_Obj_Heading) -> IMAPva_g_ORI_Obj_Heading/1
  SWINve_y_Mp5_LSSMode/1 -> Runnable_IMAP_10ms_sys/49(SWINve_y_LC_Mode)
  SWINve_y_ESC_RRWHeelSpdFaultSignal/1 -> Runnable_IMAP_10ms_sys/275(SWINve_y_ESC_RRWHeelSpdFaultSignal)
  SWINve_d_EMS_RealizedPowertrainWheelTorq/1 -> Runnable_IMAP_10ms_sys/17(SWINve_g_EMS_Actual_whlTrq)
  Runnable_IMAP_10ms_sys/212(IMAPva_d_obj_TurnLight) -> IMAPva_d_obj_TurnLight/1
  SWINve_y_MP5_TLCModeSelection/1 -> Runnable_IMAP_10ms_sys/236(SWINve_y_MP5_TLCModeSelection)
  SWINve_y_ESC_ABSWorkLable/1 -> Runnable_IMAP_10ms_sys/1(SWINve_y_ABS_in_regulation)
  SWINve_g_SAS_SteeringRotSpd/1 -> Runnable_IMAP_10ms_sys/71(SWINve_g_Steering_wheel_rotation_speed)
  Runnable_IMAP_10ms_sys/138(IMAPve_d_ESC_AVH_Status) -> IMAPve_d_ESC_AVH_Status/1
  SWINve_g_EMS_MinPowertrainWheelTorque/1 -> Runnable_IMAP_10ms_sys/25(SWINve_g_EMS_WhlTrq_min)
  SDFAva_g_obj_pos_var_y/1 -> Runnable_IMAP_10ms_sys/107(SDFAva_g_obj_pos_var_y)
  Runnable_IMAP_10ms_sys/172(IMAPve_g_ORI_L1_VR) -> IMAPve_g_ORI_L1_VR/1
  Runnable_IMAP_10ms_sys/249(IMAPve_g_L0_C1_Back) -> IMAPve_g_L0_C1_Back/1
  SWINve_y_MP5_FCWSensitivity/1 -> Runnable_IMAP_10ms_sys/44(SWINve_y_IC_FCW_Sensitivity)
  Runnable_IMAP_10ms_sys/378(IMAPva_d_ORI_Obj_BrakeLight) -> IMAPva_d_ORI_Obj_BrakeLight/1
  SWINve_y_TCU_ShiftLeverPosValidFlag/1 -> Runnable_IMAP_10ms_sys/266(SWINve_y_TCU_ShiftLeverPosValidFlag)
  Runnable_IMAP_10ms_sys/339(IMAPve_d_ORI_FS_PartialBlockage0) -> IMAPve_d_ORI_FS_PartialBlockage0/1
  SDFAva_g_obj_width/1 -> Runnable_IMAP_10ms_sys/109(SDFAva_g_obj_width)
  Runnable_IMAP_10ms_sys/199(IMAPva_g_obj_vel_x) -> IMAPva_g_obj_vel_x/1
  Runnable_IMAP_10ms_sys/217(IMAPve_g_L0_C1) -> IMAPve_g_L0_C1/1
  Runnable_IMAP_10ms_sys/213(IMAPva_d_obj_BrakeLight) -> IMAPva_d_obj_BrakeLight/1
  Runnable_IMAP_10ms_sys/51(IMAPve_d_BCM_LR_Door_State) -> IMAPve_d_BCM_LR_Door_State/1
  SWINve_y_ESC_AVHStatus/1 -> Runnable_IMAP_10ms_sys/285(SWINve_y_ESC_AVHStatus)
  Runnable_IMAP_10ms_sys/247(IMAPve_g_R1_W) -> IMAPve_g_R1_W/1
  Runnable_IMAP_10ms_sys/197(IMAPva_g_obj_pos_x) -> IMAPva_g_obj_pos_x/1
  SWINve_y_TCU_SelectedATMode/1 -> Runnable_IMAP_10ms_sys/80(SWINve_y_TCU_PROGRAMME_ACC)
  Runnable_IMAP_10ms_sys/79(IMAPve_d_SWS_Failure_Status) -> IMAPve_d_SWS_Failure_Status/1
  SWINve_y_ESC_MSRinRegulation/1 -> Runnable_IMAP_10ms_sys/53(SWINve_y_MSR_in_regulation)
  Runnable_IMAP_10ms_sys/205(IMAPva_g_obj_pos_var_xy) -> IMAPva_g_obj_pos_var_xy/1
  SWINve_y_ESC_YawrateValidity/1 -> Runnable_IMAP_10ms_sys/268(SWINve_y_ESC_YawrateValidity)
  Runnable_IMAP_10ms_sys/254(IMAPve_g_R0_C1_Back) -> IMAPve_g_R0_C1_Back/1
  SWINve_g_IC_TotalOdemeter/1 -> Runnable_IMAP_10ms_sys/58(SWINve_g_number_of_kilometer)
  Runnable_IMAP_10ms_sys/198(IMAPva_g_obj_pos_y) -> IMAPva_g_obj_pos_y/1
  Runnable_IMAP_10ms_sys/200(IMAPva_g_obj_vel_y) -> IMAPva_g_obj_vel_y/1
  SWINve_y_MP5_ADASSpeedLimit/1 -> Runnable_IMAP_10ms_sys/235(SWINve_y_MP5_ADASSpeedLimit)
  Runnable_IMAP_10ms_sys/155(IMAPva_g_ORI_Obj_LongDis) -> IMAPva_g_ORI_Obj_LongDis/1
  Runnable_IMAP_10ms_sys/234(IMAPve_g_L1_C2) -> IMAPve_g_L1_C2/1
  SWINve_y_ESC_BLRequest/1 -> Runnable_IMAP_10ms_sys/246(SWINve_y_ESC_BLRequest)
  Runnable_IMAP_10ms_sys/267(IMAPve_g_R1_Range_Back) -> IMAPve_g_R1_Range_Back/1
  Runnable_IMAP_10ms_sys/389(IMAPve_d_ORI_R0_MeasureType) -> IMAPve_d_ORI_R0_MeasureType/1
  Runnable_IMAP_10ms_sys/206(IMAPva_g_obj_width) -> IMAPva_g_obj_width/1
  Runnable_IMAP_10ms_sys/218(IMAPve_g_L0_C2) -> IMAPve_g_L0_C2/1
  Runnable_IMAP_10ms_sys/323(IMAPve_d_MP5_DMS_EyeFatigue) -> IMAPve_d_MP5_DMS_EyeFatigue/1
  Runnable_IMAP_10ms_sys/394(IMAPve_d_ORI_L1_ColorClass) -> IMAPve_d_ORI_L1_ColorClass/1
  SDFAve_g_R0_C1_BACK_COEF/1 -> Runnable_IMAP_10ms_sys/157(SDFAve_g_R0_C1_BACK_COEF)
  Runnable_IMAP_10ms_sys/7(IMAPve_d_TSR_Switch) -> IMAPve_d_TSR_Switch/1
  Runnable_IMAP_10ms_sys/196(IMAPva_d_obj_id) -> IMAPva_d_obj_id/1
  SWINve_y_ACU_RearRightBeltSwitchSig/1 -> Runnable_IMAP_10ms_sys/209(SWINve_y_ACU_RearRightBeltSwitchSig)
  Runnable_IMAP_10ms_sys/219(IMAPve_g_L0_C3) -> IMAPve_g_L0_C3/1
  SWINve_g_EMS_EngSpd/1 -> Runnable_IMAP_10ms_sys/20(SWINve_g_EMS_Engine_RPM)
  Runnable_IMAP_10ms_sys/108(IMAPve_d_TCU_Gear_Engage) -> IMAPve_d_TCU_Gear_Engage/1
  SWINve_y_TBOX_LocalTimeDate/1 -> Runnable_IMAP_10ms_sys/253(SWINve_y_TBOX_LocalTimeDate)
  SWINve_y_BCM_HazardLampSt/1 -> Runnable_IMAP_10ms_sys/8(SWINve_y_BCM_Status_Indicator)
